simulink model "lagrange_model_v2"  (R2022a)
(part 3 of 3)

M32 = 1.3806*(0.19*cos(th4(t))*(cos(th3(t) - 1.5708)*(sin(th2(t) - 1.5708)*(1.0*cos(th1(t)) - 2.6536e-6*sin(th1(t))) - 1.3268e-6*cos(th2(t) - 1.5708)*sin(th1(t))) + sin(th3(t) - 1.5708)*(cos(th2(t) - 1.5708)*(1.0*cos(th1(t)) - 2.6536e-6*sin(th1(t))) + 1.3268e-6*sin(th2(t) - 1.5708)*sin(th1(t)))) + 0.38*cos(th3(t))*(sin(th2(t) - 1.5708)*(1.0*cos(th1(t)) - 2.6536e-6*sin(th1(t))) - 1.3268e-6*cos(th2(t) - 1.5708)*sin(th1(t))) + 0.38*sin(th3(t))*(cos(th2(t) - 1.5708)*(1.0*cos(th1(t)) - 2.6536e-6*sin(th1(t))) + 1.3268e-6*sin(th2(t) - 1.5708)*sin(th1(t))) + 0.19*sin(th4(t))*(cos(th3(t) - 1.5708)*(cos(th2(t) - 1.5708)*(1.0*cos(th1(t)) - 2.6536e-6*sin(th1(t))) + 1.3268e-6*sin(th2(t) - 1.5708)*sin(th1(t))) - 1.0*sin(th3(t) - 1.5708)*(sin(th2(t) - 1.5708)*(1.0*cos(th1(t)) - 2.6536e-6*sin(th1(t))) - 1.3268e-6*cos(th2(t) - 1.5708)*sin(th1(t)))))*(0.19*cos(th4(t))*(cos(th3(t) - 1.5708)*(sin(th2(t) - 1.5708)*(1.0*cos(th1(t)) - 2.6536e-6*sin(th1(t))) - 1.3268e-6*cos(th2(t) - 1.5708)*sin(th1(t))) + sin(th3(t) - 1.5708)*(cos(th2(t) - 1.5708)*(1.0*cos(th1(t)) - 2.6536e-6*sin(th1(t))) + 1.3268e-6*sin(th2(t) - 1.5708)*sin(th1(t)))) - 5.0418e-7*cos(th2(t))*sin(th1(t)) + 0.38*cos(th3(t))*(sin(th2(t) - 1.5708)*(1.0*cos(th1(t)) - 2.6536e-6*sin(th1(t))) - 1.3268e-6*cos(th2(t) - 1.5708)*sin(th1(t))) + 0.38*sin(th2(t))*(1.0*cos(th1(t)) - 2.6536e-6*sin(th1(t))) + 0.38*sin(th3(t))*(cos(th2(t) - 1.5708)*(1.0*cos(th1(t)) - 2.6536e-6*sin(th1(t))) + 1.3268e-6*sin(th2(t) - 1.5708)*sin(th1(t))) + 0.19*sin(th4(t))*(cos(th3(t) - 1.5708)*(cos(th2(t) - 1.5708)*(1.0*cos(th1(t)) - 2.6536e-6*sin(th1(t))) + 1.3268e-6*sin(th2(t) - 1.5708)*sin(th1(t))) - 1.0*sin(th3(t) - 1.5708)*(sin(th2(t) - 1.5708)*(1.0*cos(th1(t)) - 2.6536e-6*sin(th1(t))) - 1.3268e-6*cos(th2(t) - 1.5708)*sin(th1(t))))) - 1.3806*(0.38*sin(th3(t))*(3.5208e-12*cos(th2(t) - 1.5708) + 1.0*sin(th2(t) - 1.5708)) + 0.19*sin(th4(t))*(cos(th3(t) - 1.5708)*(3.5208e-12*cos(th2(t) - 1.5708) + 1.0*sin(th2(t) - 1.5708)) + sin(th3(t) - 1.5708)*(1.0*cos(th2(t) - 1.5708) - 3.5208e-12*sin(th2(t) - 1.5708))) - 0.19*cos(th4(t))*(cos(th3(t) - 1.5708)*(1.0*cos(th2(t) - 1.5708) - 3.5208e-12*sin(th2(t) - 1.5708)) - 1.0*sin(th3(t) - 1.5708)*(3.5208e-12*cos(th2(t) - 1.5708) + 1.0*sin(th2(t) - 1.5708))) - 0.38*cos(th3(t))*(1.0*cos(th2(t) - 1.5708) - 3.5208e-12*sin(th2(t) - 1.5708)))*(0.38*cos(th2(t)) - 1.3379e-12*sin(th2(t)) - 0.38*sin(th3(t))*(3.5208e-12*cos(th2(t) - 1.5708) + 1.0*sin(th2(t) - 1.5708)) - 0.19*sin(th4(t))*(cos(th3(t) - 1.5708)*(3.5208e-12*cos(th2(t) - 1.5708) + 1.0*sin(th2(t) - 1.5708)) + sin(th3(t) - 1.5708)*(1.0*cos(th2(t) - 1.5708) - 3.5208e-12*sin(th2(t) - 1.5708))) + 0.19*cos(th4(t))*(cos(th3(t) - 1.5708)*(1.0*cos(th2(t) - 1.5708) - 3.5208e-12*sin(th2(t) - 1.5708)) - 1.0*sin(th3(t) - 1.5708)*(3.5208e-12*cos(th2(t) - 1.5708) + 1.0*sin(th2(t) - 1.5708))) + 0.38*cos(th3(t))*(1.0*cos(th2(t) - 1.5708) - 3.5208e-12*sin(th2(t) - 1.5708))) + 0.13038*(0.38*cos(th3(t))*(sin(th2(t) - 1.5708)*(2.6536e-6*cos(th1(t)) + 1.0*sin(th1(t))) + 1.3268e-6*cos(th2(t) - 1.5708)*cos(th1(t))) - 0.38*sin(th4(t))*(sin(th3(t) - 1.5708)*(sin(th2(t) - 1.5708)*(2.6536e-6*cos(th1(t)) + 1.0*sin(th1(t))) + 1.3268e-6*cos(th2(t) - 1.5708)*cos(th1(t))) - cos(th3(t) - 1.5708)*(1.0*cos(th2(t) - 1.5708)*(2.6536e-6*cos(th1(t)) + 1.0*sin(th1(t))) - 1.3268e-6*sin(th2(t) - 1.5708)*cos(th1(t)))) + 0.38*sin(th3(t))*(1.0*cos(th2(t) - 1.5708)*(2.6536e-6*cos(th1(t)) + 1.0*sin(th1(t))) - 1.3268e-6*sin(th2(t) - 1.5708)*cos(th1(t))) - 0.02*cos(th5(t))*(sin(th4(t) - 3.1416)*(sin(th3(t) - 1.5708)*(sin(th2(t) - 1.5708)*(2.6536e-6*cos(th1(t)) + 1.0*sin(th1(t))) + 1.3268e-6*cos(th2(t) - 1.5708)*cos(th1(t))) - cos(th3(t) - 1.5708)*(1.0*cos(th2(t) - 1.5708)*(2.6536e-6*cos(th1(t)) + 1.0*sin(th1(t))) - 1.3268e-6*sin(th2(t) - 1.5708)*cos(th1(t)))) + cos(th4(t) - 3.1416)*(cos(th3(t) - 1.5708)*(sin(th2(t) - 1.5708)*(2.6536e-6*cos(th1(t)) + 1.0*sin(th1(t))) + 1.3268e-6*cos(th2(t) - 1.5708)*cos(th1(t))) + 1.0*sin(th3(t) - 1.5708)*(1.0*cos(th2(t) - 1.5708)*(2.6536e-6*cos(th1(t)) + 1.0*sin(th1(t))) - 1.3268e-6*sin(th2(t) - 1.5708)*cos(th1(t))))) + 0.38*cos(th4(t))*(cos(th3(t) - 1.5708)*(sin(th2(t) - 1.5708)*(2.6536e-6*cos(th1(t)) + 1.0*sin(th1(t))) + 1.3268e-6*cos(th2(t) - 1.5708)*cos(th1(t))) + 1.0*sin(th3(t) - 1.5708)*(1.0*cos(th2(t) - 1.5708)*(2.6536e-6*cos(th1(t)) + 1.0*sin(th1(t))) - 1.3268e-6*sin(th2(t) - 1.5708)*cos(th1(t)))) + 0.02*sin(th5(t))*(cos(th4(t) - 3.1416)*(sin(th3(t) - 1.5708)*(sin(th2(t) - 1.5708)*(2.6536e-6*cos(th1(t)) + 1.0*sin(th1(t))) + 1.3268e-6*cos(th2(t) - 1.5708)*cos(th1(t))) - cos(th3(t) - 1.5708)*(1.0*cos(th2(t) - 1.5708)*(2.6536e-6*cos(th1(t)) + 1.0*sin(th1(t))) - 1.3268e-6*sin(th2(t) - 1.5708)*cos(th1(t)))) - 1.0*sin(th4(t) - 3.1416)*(cos(th3(t) - 1.5708)*(sin(th2(t) - 1.5708)*(2.6536e-6*cos(th1(t)) + 1.0*sin(th1(t))) + 1.3268e-6*cos(th2(t) - 1.5708)*cos(th1(t))) + 1.0*sin(th3(t) - 1.5708)*(1.0*cos(th2(t) - 1.5708)*(2.6536e-6*cos(th1(t)) + 1.0*sin(th1(t))) - 1.3268e-6*sin(th2(t) - 1.5708)*cos(th1(t))))))*(0.38*cos(th3(t))*(sin(th2(t) - 1.5708)*(2.6536e-6*cos(th1(t)) + 1.0*sin(th1(t))) + 1.3268e-6*cos(th2(t) - 1.5708)*cos(th1(t))) + 0.38*sin(th2(t))*(2.6536e-6*cos(th1(t)) + 1.0*sin(th1(t))) - 0.38*sin(th4(t))*(sin(th3(t) - 1.5708)*(sin(th2(t) - 1.5708)*(2.6536e-6*cos(th1(t)) + 1.0*sin(th1(t))) + 1.3268e-6*cos(th2(t) - 1.5708)*cos(th1(t))) - cos(th3(t) - 1.5708)*(1.0*cos(th2(t) - 1.5708)*(2.6536e-6*cos(th1(t)) + 1.0*sin(th1(t))) - 1.3268e-6*sin(th2(t) - 1.5708)*cos(th1(t)))) + 0.38*sin(th3(t))*(1.0*cos(th2(t) - 1.5708)*(2.6536e-6*cos(th1(t)) + 1.0*sin(th1(t))) - 1.3268e-6*sin(th2(t) - 1.5708)*cos(th1(t))) - 0.02*cos(th5(t))*(sin(th4(t) - 3.1416)*(sin(th3(t) - 1.5708)*(sin(th2(t) - 1.5708)*(2.6536e-6*cos(th1(t)) + 1.0*sin(th1(t))) + 1.3268e-6*cos(th2(t) - 1.5708)*cos(th1(t))) - cos(th3(t) - 1.5708)*(1.0*cos(th2(t) - 1.5708)*(2.6536e-6*cos(th1(t)) + 1.0*sin(th1(t))) - 1.3268e-6*sin(th2(t) - 1.5708)*cos(th1(t)))) + cos(th4(t) - 3.1416)*(cos(th3(t) - 1.5708)*(sin(th2(t) - 1.5708)*(2.6536e-6*cos(th1(t)) + 1.0*sin(th1(t))) + 1.3268e-6*cos(th2(t) - 1.5708)*cos(th1(t))) + 1.0*sin(th3(t) - 1.5708)*(1.0*cos(th2(t) - 1.5708)*(2.6536e-6*cos(th1(t)) + 1.0*sin(th1(t))) - 1.3268e-6*sin(th2(t) - 1.5708)*cos(th1(t))))) + 0.38*cos(th4(t))*(cos(th3(t) - 1.5708)*(sin(th2(t) - 1.5708)*(2.6536e-6*cos(th1(t)) + 1.0*sin(th1(t))) + 1.3268e-6*cos(th2(t) - 1.5708)*cos(th1(t))) + 1.0*sin(th3(t) - 1.5708)*(1.0*cos(th2(t) - 1.5708)*(2.6536e-6*cos(th1(t)) + 1.0*sin(th1(t))) - 1.3268e-6*sin(th2(t) - 1.5708)*cos(th1(t)))) + 0.02*sin(th5(t))*(cos(th4(t) - 3.1416)*(sin(th3(t) - 1.5708)*(sin(th2(t) - 1.5708)*(2.6536e-6*cos(th1(t)) + 1.0*sin(th1(t))) + 1.3268e-6*cos(th2(t) - 1.5708)*cos(th1(t))) - cos(th3(t) - 1.5708)*(1.0*cos(th2(t) - 1.5708)*(2.6536e-6*cos(th1(t)) + 1.0*sin(th1(t))) - 1.3268e-6*sin(th2(t) - 1.5708)*cos(th1(t)))) - 1.0*sin(th4(t) - 3.1416)*(cos(th3(t) - 1.5708)*(sin(th2(t) - 1.5708)*(2.6536e-6*cos(th1(t)) + 1.0*sin(th1(t))) + 1.3268e-6*cos(th2(t) - 1.5708)*cos(th1(t))) + 1.0*sin(th3(t) - 1.5708)*(1.0*cos(th2(t) - 1.5708)*(2.6536e-6*cos(th1(t)) + 1.0*sin(th1(t))) - 1.3268e-6*sin(th2(t) - 1.5708)*cos(th1(t))))) + 5.0418e-7*cos(th1(t))*cos(th2(t))) + 0.49277*(0.19*cos(th3(t))*(sin(th2(t) - 1.5708)*(2.6536e-6*cos(th1(t)) + 1.0*sin(th1(t))) + 1.3268e-6*cos(th2(t) - 1.5708)*cos(th1(t))) + 0.19*sin(th3(t))*(1.0*cos(th2(t) - 1.5708)*(2.6536e-6*cos(th1(t)) + 1.0*sin(th1(t))) - 1.3268e-6*sin(th2(t) - 1.5708)*cos(th1(t))))*(0.19*cos(th3(t))*(sin(th2(t) - 1.5708)*(2.6536e-6*cos(th1(t)) + 1.0*sin(th1(t))) + 1.3268e-6*cos(th2(t) - 1.5708)*cos(th1(t))) + 0.38*sin(th2(t))*(2.6536e-6*cos(th1(t)) + 1.0*sin(th1(t))) + 0.19*sin(th3(t))*(1.0*cos(th2(t) - 1.5708)*(2.6536e-6*cos(th1(t)) + 1.0*sin(th1(t))) - 1.3268e-6*sin(th2(t) - 1.5708)*cos(th1(t))) + 5.0418e-7*cos(th1(t))*cos(th2(t))) + 0.13038*(0.38*cos(th4(t))*(cos(th3(t) - 1.5708)*(sin(th2(t) - 1.5708)*(1.0*cos(th1(t)) - 2.6536e-6*sin(th1(t))) - 1.3268e-6*cos(th2(t) - 1.5708)*sin(th1(t))) + sin(th3(t) - 1.5708)*(cos(th2(t) - 1.5708)*(1.0*cos(th1(t)) - 2.6536e-6*sin(th1(t))) + 1.3268e-6*sin(th2(t) - 1.5708)*sin(th1(t)))) + 0.38*cos(th3(t))*(sin(th2(t) - 1.5708)*(1.0*cos(th1(t)) - 2.6536e-6*sin(th1(t))) - 1.3268e-6*cos(th2(t) - 1.5708)*sin(th1(t))) + 0.38*sin(th3(t))*(cos(th2(t) - 1.5708)*(1.0*cos(th1(t)) - 2.6536e-6*sin(th1(t))) + 1.3268e-6*sin(th2(t) - 1.5708)*sin(th1(t))) - 0.02*sin(th5(t))*(sin(th4(t) - 3.1416)*(cos(th3(t) - 1.5708)*(sin(th2(t) - 1.5708)*(1.0*cos(th1(t)) - 2.6536e-6*sin(th1(t))) - 1.3268e-6*cos(th2(t) - 1.5708)*sin(th1(t))) + sin(th3(t) - 1.5708)*(cos(th2(t) - 1.5708)*(1.0*cos(th1(t)) - 2.6536e-6*sin(th1(t))) + 1.3268e-6*sin(th2(t) - 1.5708)*sin(th1(t)))) + cos(th4(t) - 3.1416)*(cos(th3(t) - 1.5708)*(cos(th2(t) - 1.5708)*(1.0*cos(th1(t)) - 2.6536e-6*sin(th1(t))) + 1.3268e-6*sin(th2(t) - 1.5708)*sin(th1(t))) - 1.0*sin(th3(t) - 1.5708)*(sin(th2(t) - 1.5708)*(1.0*cos(th1(t)) - 2.6536e-6*sin(th1(t))) - 1.3268e-6*cos(th2(t) - 1.5708)*sin(th1(t))))) + 0.38*sin(th4(t))*(cos(th3(t) - 1.5708)*(cos(th2(t) - 1.5708)*(1.0*cos(th1(t)) - 2.6536e-6*sin(th1(t))) + 1.3268e-6*sin(th2(t) - 1.5708)*sin(th1(t))) - 1.0*sin(th3(t) - 1.5708)*(sin(th2(t) - 1.5708)*(1.0*cos(th1(t)) - 2.6536e-6*sin(th1(t))) - 1.3268e-6*cos(th2(t) - 1.5708)*sin(th1(t)))) - 0.02*cos(th5(t))*(cos(th4(t) - 3.1416)*(cos(th3(t) - 1.5708)*(sin(th2(t) - 1.5708)*(1.0*cos(th1(t)) - 2.6536e-6*sin(th1(t))) - 1.3268e-6*cos(th2(t) - 1.5708)*sin(th1(t))) + sin(th3(t) - 1.5708)*(cos(th2(t) - 1.5708)*(1.0*cos(th1(t)) - 2.6536e-6*sin(th1(t))) + 1.3268e-6*sin(th2(t) - 1.5708)*sin(th1(t)))) - 1.0*sin(th4(t) - 3.1416)*(cos(th3(t) - 1.5708)*(cos(th2(t) - 1.5708)*(1.0*cos(th1(t)) - 2.6536e-6*sin(th1(t))) + 1.3268e-6*sin(th2(t) - 1.5708)*sin(th1(t))) - 1.0*sin(th3(t) - 1.5708)*(sin(th2(t) - 1.5708)*(1.0*cos(th1(t)) - 2.6536e-6*sin(th1(t))) - 1.3268e-6*cos(th2(t) - 1.5708)*sin(th1(t))))))*(0.38*cos(th4(t))*(cos(th3(t) - 1.5708)*(sin(th2(t) - 1.5708)*(1.0*cos(th1(t)) - 2.6536e-6*sin(th1(t))) - 1.3268e-6*cos(th2(t) - 1.5708)*sin(th1(t))) + sin(th3(t) - 1.5708)*(cos(th2(t) - 1.5708)*(1.0*cos(th1(t)) - 2.6536e-6*sin(th1(t))) + 1.3268e-6*sin(th2(t) - 1.5708)*sin(th1(t)))) - 5.0418e-7*cos(th2(t))*sin(th1(t)) + 0.38*cos(th3(t))*(sin(th2(t) - 1.5708)*(1.0*cos(th1(t)) - 2.6536e-6*sin(th1(t))) - 1.3268e-6*cos(th2(t) - 1.5708)*sin(th1(t))) + 0.38*sin(th2(t))*(1.0*cos(th1(t)) - 2.6536e-6*sin(th1(t))) + 0.38*sin(th3(t))*(cos(th2(t) - 1.5708)*(1.0*cos(th1(t)) - 2.6536e-6*sin(th1(t))) + 1.3268e-6*sin(th2(t) - 1.5708)*sin(th1(t))) - 0.02*sin(th5(t))*(sin(th4(t) - 3.1416)*(cos(th3(t) - 1.5708)*(sin(th2(t) - 1.5708)*(1.0*cos(th1(t)) - 2.6536e-6*sin(th1(t))) - 1.3268e-6*cos(th2(t) - 1.5708)*sin(th1(t))) + sin(th3(t) - 1.5708)*(cos(th2(t) - 1.5708)*(1.0*cos(th1(t)) - 2.6536e-6*sin(th1(t))) + 1.3268e-6*sin(th2(t) - 1.5708)*sin(th1(t)))) + cos(th4(t) - 3.1416)*(cos(th3(t) - 1.5708)*(cos(th2(t) - 1.5708)*(1.0*cos(th1(t)) - 2.6536e-6*sin(th1(t))) + 1.3268e-6*sin(th2(t) - 1.5708)*sin(th1(t))) - 1.0*sin(th3(t) - 1.5708)*(sin(th2(t) - 1.5708)*(1.0*cos(th1(t)) - 2.6536e-6*sin(th1(t))) - 1.3268e-6*cos(th2(t) - 1.5708)*sin(th1(t))))) + 0.38*sin(th4(t))*(cos(th3(t) - 1.5708)*(cos(th2(t) - 1.5708)*(1.0*cos(th1(t)) - 2.6536e-6*sin(th1(t))) + 1.3268e-6*sin(th2(t) - 1.5708)*sin(th1(t))) - 1.0*sin(th3(t) - 1.5708)*(sin(th2(t) - 1.5708)*(1.0*cos(th1(t)) - 2.6536e-6*sin(th1(t))) - 1.3268e-6*cos(th2(t) - 1.5708)*sin(th1(t)))) - 0.02*cos(th5(t))*(cos(th4(t) - 3.1416)*(cos(th3(t) - 1.5708)*(sin(th2(t) - 1.5708)*(1.0*cos(th1(t)) - 2.6536e-6*sin(th1(t))) - 1.3268e-6*cos(th2(t) - 1.5708)*sin(th1(t))) + sin(th3(t) - 1.5708)*(cos(th2(t) - 1.5708)*(1.0*cos(th1(t)) - 2.6536e-6*sin(th1(t))) + 1.3268e-6*sin(th2(t) - 1.5708)*sin(th1(t)))) - 1.0*sin(th4(t) - 3.1416)*(cos(th3(t) - 1.5708)*(cos(th2(t) - 1.5708)*(1.0*cos(th1(t)) - 2.6536e-6*sin(th1(t))) + 1.3268e-6*sin(th2(t) - 1.5708)*sin(th1(t))) - 1.0*sin(th3(t) - 1.5708)*(sin(th2(t) - 1.5708)*(1.0*cos(th1(t)) - 2.6536e-6*sin(th1(t))) - 1.3268e-6*cos(th2(t) - 1.5708)*sin(th1(t)))))) - 0.49277*(0.19*sin(th3(t))*(3.5208e-12*cos(th2(t) - 1.5708) + 1.0*sin(th2(t) - 1.5708)) - 0.19*cos(th3(t))*(1.0*cos(th2(t) - 1.5708) - 3.5208e-12*sin(th2(t) - 1.5708)))*(0.38*cos(th2(t)) - 1.3379e-12*sin(th2(t)) - 0.19*sin(th3(t))*(3.5208e-12*cos(th2(t) - 1.5708) + 1.0*sin(th2(t) - 1.5708)) + 0.19*cos(th3(t))*(1.0*cos(th2(t) - 1.5708) - 3.5208e-12*sin(th2(t) - 1.5708))) + 1.3806*(0.38*cos(th3(t))*(sin(th2(t) - 1.5708)*(2.6536e-6*cos(th1(t)) + 1.0*sin(th1(t))) + 1.3268e-6*cos(th2(t) - 1.5708)*cos(th1(t))) - 0.19*sin(th4(t))*(sin(th3(t) - 1.5708)*(sin(th2(t) - 1.5708)*(2.6536e-6*cos(th1(t)) + 1.0*sin(th1(t))) + 1.3268e-6*cos(th2(t) - 1.5708)*cos(th1(t))) - cos(th3(t) - 1.5708)*(1.0*cos(th2(t) - 1.5708)*(2.6536e-6*cos(th1(t)) + 1.0*sin(th1(t))) - 1.3268e-6*sin(th2(t) - 1.5708)*cos(th1(t)))) + 0.38*sin(th3(t))*(1.0*cos(th2(t) - 1.5708)*(2.6536e-6*cos(th1(t)) + 1.0*sin(th1(t))) - 1.3268e-6*sin(th2(t) - 1.5708)*cos(th1(t))) + 0.19*cos(th4(t))*(cos(th3(t) - 1.5708)*(sin(th2(t) - 1.5708)*(2.6536e-6*cos(th1(t)) + 1.0*sin(th1(t))) + 1.3268e-6*cos(th2(t) - 1.5708)*cos(th1(t))) + 1.0*sin(th3(t) - 1.5708)*(1.0*cos(th2(t) - 1.5708)*(2.6536e-6*cos(th1(t)) + 1.0*sin(th1(t))) - 1.3268e-6*sin(th2(t) - 1.5708)*cos(th1(t)))))*(0.38*cos(th3(t))*(sin(th2(t) - 1.5708)*(2.6536e-6*cos(th1(t)) + 1.0*sin(th1(t))) + 1.3268e-6*cos(th2(t) - 1.5708)*cos(th1(t))) + 0.38*sin(th2(t))*(2.6536e-6*cos(th1(t)) + 1.0*sin(th1(t))) - 0.19*sin(th4(t))*(sin(th3(t) - 1.5708)*(sin(th2(t) - 1.5708)*(2.6536e-6*cos(th1(t)) + 1.0*sin(th1(t))) + 1.3268e-6*cos(th2(t) - 1.5708)*cos(th1(t))) - cos(th3(t) - 1.5708)*(1.0*cos(th2(t) - 1.5708)*(2.6536e-6*cos(th1(t)) + 1.0*sin(th1(t))) - 1.3268e-6*sin(th2(t) - 1.5708)*cos(th1(t)))) + 0.38*sin(th3(t))*(1.0*cos(th2(t) - 1.5708)*(2.6536e-6*cos(th1(t)) + 1.0*sin(th1(t))) - 1.3268e-6*sin(th2(t) - 1.5708)*cos(th1(t))) + 0.19*cos(th4(t))*(cos(th3(t) - 1.5708)*(sin(th2(t) - 1.5708)*(2.6536e-6*cos(th1(t)) + 1.0*sin(th1(t))) + 1.3268e-6*cos(th2(t) - 1.5708)*cos(th1(t))) + 1.0*sin(th3(t) - 1.5708)*(1.0*cos(th2(t) - 1.5708)*(2.6536e-6*cos(th1(t)) + 1.0*sin(th1(t))) - 1.3268e-6*sin(th2(t) - 1.5708)*cos(th1(t)))) + 5.0418e-7*cos(th1(t))*cos(th2(t))) - 0.13038*(0.38*sin(th3(t))*(3.5208e-12*cos(th2(t) - 1.5708) + 1.0*sin(th2(t) - 1.5708)) - 0.02*sin(th5(t))*(cos(th4(t) - 3.1416)*(cos(th3(t) - 1.5708)*(3.5208e-12*cos(th2(t) - 1.5708) + 1.0*sin(th2(t) - 1.5708)) + sin(th3(t) - 1.5708)*(1.0*cos(th2(t) - 1.5708) - 3.5208e-12*sin(th2(t) - 1.5708))) - 1.0*sin(th4(t) - 3.1416)*(cos(th3(t) - 1.5708)*(1.0*cos(th2(t) - 1.5708) - 3.5208e-12*sin(th2(t) - 1.5708)) - 1.0*sin(th3(t) - 1.5708)*(3.5208e-12*cos(th2(t) - 1.5708) + 1.0*sin(th2(t) - 1.5708)))) + 0.38*sin(th4(t))*(cos(th3(t) - 1.5708)*(3.5208e-12*cos(th2(t) - 1.5708) + 1.0*sin(th2(t) - 1.5708)) + sin(th3(t) - 1.5708)*(1.0*cos(th2(t) - 1.5708) - 3.5208e-12*sin(th2(t) - 1.5708))) - 0.38*cos(th4(t))*(cos(th3(t) - 1.5708)*(1.0*cos(th2(t) - 1.5708) - 3.5208e-12*sin(th2(t) - 1.5708)) - 1.0*sin(th3(t) - 1.5708)*(3.5208e-12*cos(th2(t) - 1.5708) + 1.0*sin(th2(t) - 1.5708))) - 0.38*cos(th3(t))*(1.0*cos(th2(t) - 1.5708) - 3.5208e-12*sin(th2(t) - 1.5708)) + 0.02*cos(th5(t))*(sin(th4(t) - 3.1416)*(cos(th3(t) - 1.5708)*(3.5208e-12*cos(th2(t) - 1.5708) + 1.0*sin(th2(t) - 1.5708)) + sin(th3(t) - 1.5708)*(1.0*cos(th2(t) - 1.5708) - 3.5208e-12*sin(th2(t) - 1.5708))) + cos(th4(t) - 3.1416)*(cos(th3(t) - 1.5708)*(1.0*cos(th2(t) - 1.5708) - 3.5208e-12*sin(th2(t) - 1.5708)) - 1.0*sin(th3(t) - 1.5708)*(3.5208e-12*cos(th2(t) - 1.5708) + 1.0*sin(th2(t) - 1.5708)))))*(0.38*cos(th2(t)) - 1.3379e-12*sin(th2(t)) - 0.38*sin(th3(t))*(3.5208e-12*cos(th2(t) - 1.5708) + 1.0*sin(th2(t) - 1.5708)) + 0.02*sin(th5(t))*(cos(th4(t) - 3.1416)*(cos(th3(t) - 1.5708)*(3.5208e-12*cos(th2(t) - 1.5708) + 1.0*sin(th2(t) - 1.5708)) + sin(th3(t) - 1.5708)*(1.0*cos(th2(t) - 1.5708) - 3.5208e-12*sin(th2(t) - 1.5708))) - 1.0*sin(th4(t) - 3.1416)*(cos(th3(t) - 1.5708)*(1.0*cos(th2(t) - 1.5708) - 3.5208e-12*sin(th2(t) - 1.5708)) - 1.0*sin(th3(t) - 1.5708)*(3.5208e-12*cos(th2(t) - 1.5708) + 1.0*sin(th2(t) - 1.5708)))) - 0.38*sin(th4(t))*(cos(th3(t) - 1.5708)*(3.5208e-12*cos(th2(t) - 1.5708) + 1.0*sin(th2(t) - 1.5708)) + sin(th3(t) - 1.5708)*(1.0*cos(th2(t) - 1.5708) - 3.5208e-12*sin(th2(t) - 1.5708))) + 0.38*cos(th4(t))*(cos(th3(t) - 1.5708)*(1.0*cos(th2(t) - 1.5708) - 3.5208e-12*sin(th2(t) - 1.5708)) - 1.0*sin(th3(t) - 1.5708)*(3.5208e-12*cos(th2(t) - 1.5708) + 1.0*sin(th2(t) - 1.5708))) + 0.38*cos(th3(t))*(1.0*cos(th2(t) - 1.5708) - 3.5208e-12*sin(th2(t) - 1.5708)) - 0.02*cos(th5(t))*(sin(th4(t) - 3.1416)*(cos(th3(t) - 1.5708)*(3.5208e-12*cos(th2(t) - 1.5708) + 1.0*sin(th2(t) - 1.5708)) + sin(th3(t) - 1.5708)*(1.0*cos(th2(t) - 1.5708) - 3.5208e-12*sin(th2(t) - 1.5708))) + cos(th4(t) - 3.1416)*(cos(th3(t) - 1.5708)*(1.0*cos(th2(t) - 1.5708) - 3.5208e-12*sin(th2(t) - 1.5708)) - 1.0*sin(th3(t) - 1.5708)*(3.5208e-12*cos(th2(t) - 1.5708) + 1.0*sin(th2(t) - 1.5708))))) + 0.49277*(0.19*cos(th3(t))*(sin(th2(t) - 1.5708)*(1.0*cos(th1(t)) - 2.6536e-6*sin(th1(t))) - 1.3268e-6*cos(th2(t) - 1.5708)*sin(th1(t))) + 0.19*sin(th3(t))*(cos(th2(t) - 1.5708)*(1.0*cos(th1(t)) - 2.6536e-6*sin(th1(t))) + 1.3268e-6*sin(th2(t) - 1.5708)*sin(th1(t))))*(0.19*cos(th3(t))*(sin(th2(t) - 1.5708)*(1.0*cos(th1(t)) - 2.6536e-6*sin(th1(t))) - 1.3268e-6*cos(th2(t) - 1.5708)*sin(th1(t))) - 5.0418e-7*cos(th2(t))*sin(th1(t)) + 0.38*sin(th2(t))*(1.0*cos(th1(t)) - 2.6536e-6*sin(th1(t))) + 0.19*sin(th3(t))*(cos(th2(t) - 1.5708)*(1.0*cos(th1(t)) - 2.6536e-6*sin(th1(t))) + 1.3268e-6*sin(th2(t) - 1.5708)*sin(th1(t)))) + 0.051004;
M33 = 1.3806*(0.38*cos(th3(t))*(sin(th2(t) - 1.5708)*(2.6536e-6*cos(th1(t)) + 1.0*sin(th1(t))) + 1.3268e-6*cos(th2(t) - 1.5708)*cos(th1(t))) - 0.19*sin(th4(t))*(sin(th3(t) - 1.5708)*(sin(th2(t) - 1.5708)*(2.6536e-6*cos(th1(t)) + 1.0*sin(th1(t))) + 1.3268e-6*cos(th2(t) - 1.5708)*cos(th1(t))) - cos(th3(t) - 1.5708)*(1.0*cos(th2(t) - 1.5708)*(2.6536e-6*cos(th1(t)) + 1.0*sin(th1(t))) - 1.3268e-6*sin(th2(t) - 1.5708)*cos(th1(t)))) + 0.38*sin(th3(t))*(1.0*cos(th2(t) - 1.5708)*(2.6536e-6*cos(th1(t)) + 1.0*sin(th1(t))) - 1.3268e-6*sin(th2(t) - 1.5708)*cos(th1(t))) + 0.19*cos(th4(t))*(cos(th3(t) - 1.5708)*(sin(th2(t) - 1.5708)*(2.6536e-6*cos(th1(t)) + 1.0*sin(th1(t))) + 1.3268e-6*cos(th2(t) - 1.5708)*cos(th1(t))) + 1.0*sin(th3(t) - 1.5708)*(1.0*cos(th2(t) - 1.5708)*(2.6536e-6*cos(th1(t)) + 1.0*sin(th1(t))) - 1.3268e-6*sin(th2(t) - 1.5708)*cos(th1(t)))))^2 + 0.49277*(0.19*cos(th3(t))*(sin(th2(t) - 1.5708)*(1.0*cos(th1(t)) - 2.6536e-6*sin(th1(t))) - 1.3268e-6*cos(th2(t) - 1.5708)*sin(th1(t))) + 0.19*sin(th3(t))*(cos(th2(t) - 1.5708)*(1.0*cos(th1(t)) - 2.6536e-6*sin(th1(t))) + 1.3268e-6*sin(th2(t) - 1.5708)*sin(th1(t))))^2 + 0.13038*(0.38*cos(th3(t))*(sin(th2(t) - 1.5708)*(2.6536e-6*cos(th1(t)) + 1.0*sin(th1(t))) + 1.3268e-6*cos(th2(t) - 1.5708)*cos(th1(t))) - 0.38*sin(th4(t))*(sin(th3(t) - 1.5708)*(sin(th2(t) - 1.5708)*(2.6536e-6*cos(th1(t)) + 1.0*sin(th1(t))) + 1.3268e-6*cos(th2(t) - 1.5708)*cos(th1(t))) - cos(th3(t) - 1.5708)*(1.0*cos(th2(t) - 1.5708)*(2.6536e-6*cos(th1(t)) + 1.0*sin(th1(t))) - 1.3268e-6*sin(th2(t) - 1.5708)*cos(th1(t)))) + 0.38*sin(th3(t))*(1.0*cos(th2(t) - 1.5708)*(2.6536e-6*cos(th1(t)) + 1.0*sin(th1(t))) - 1.3268e-6*sin(th2(t) - 1.5708)*cos(th1(t))) - 0.02*cos(th5(t))*(sin(th4(t) - 3.1416)*(sin(th3(t) - 1.5708)*(sin(th2(t) - 1.5708)*(2.6536e-6*cos(th1(t)) + 1.0*sin(th1(t))) + 1.3268e-6*cos(th2(t) - 1.5708)*cos(th1(t))) - cos(th3(t) - 1.5708)*(1.0*cos(th2(t) - 1.5708)*(2.6536e-6*cos(th1(t)) + 1.0*sin(th1(t))) - 1.3268e-6*sin(th2(t) - 1.5708)*cos(th1(t)))) + cos(th4(t) - 3.1416)*(cos(th3(t) - 1.5708)*(sin(th2(t) - 1.5708)*(2.6536e-6*cos(th1(t)) + 1.0*sin(th1(t))) + 1.3268e-6*cos(th2(t) - 1.5708)*cos(th1(t))) + 1.0*sin(th3(t) - 1.5708)*(1.0*cos(th2(t) - 1.5708)*(2.6536e-6*cos(th1(t)) + 1.0*sin(th1(t))) - 1.3268e-6*sin(th2(t) - 1.5708)*cos(th1(t))))) + 0.38*cos(th4(t))*(cos(th3(t) - 1.5708)*(sin(th2(t) - 1.5708)*(2.6536e-6*cos(th1(t)) + 1.0*sin(th1(t))) + 1.3268e-6*cos(th2(t) - 1.5708)*cos(th1(t))) + 1.0*sin(th3(t) - 1.5708)*(1.0*cos(th2(t) - 1.5708)*(2.6536e-6*cos(th1(t)) + 1.0*sin(th1(t))) - 1.3268e-6*sin(th2(t) - 1.5708)*cos(th1(t)))) + 0.02*sin(th5(t))*(cos(th4(t) - 3.1416)*(sin(th3(t) - 1.5708)*(sin(th2(t) - 1.5708)*(2.6536e-6*cos(th1(t)) + 1.0*sin(th1(t))) + 1.3268e-6*cos(th2(t) - 1.5708)*cos(th1(t))) - cos(th3(t) - 1.5708)*(1.0*cos(th2(t) - 1.5708)*(2.6536e-6*cos(th1(t)) + 1.0*sin(th1(t))) - 1.3268e-6*sin(th2(t) - 1.5708)*cos(th1(t)))) - 1.0*sin(th4(t) - 3.1416)*(cos(th3(t) - 1.5708)*(sin(th2(t) - 1.5708)*(2.6536e-6*cos(th1(t)) + 1.0*sin(th1(t))) + 1.3268e-6*cos(th2(t) - 1.5708)*cos(th1(t))) + 1.0*sin(th3(t) - 1.5708)*(1.0*cos(th2(t) - 1.5708)*(2.6536e-6*cos(th1(t)) + 1.0*sin(th1(t))) - 1.3268e-6*sin(th2(t) - 1.5708)*cos(th1(t))))))^2 + 0.49277*(0.19*cos(th3(t))*(sin(th2(t) - 1.5708)*(2.6536e-6*cos(th1(t)) + 1.0*sin(th1(t))) + 1.3268e-6*cos(th2(t) - 1.5708)*cos(th1(t))) + 0.19*sin(th3(t))*(1.0*cos(th2(t) - 1.5708)*(2.6536e-6*cos(th1(t)) + 1.0*sin(th1(t))) - 1.3268e-6*sin(th2(t) - 1.5708)*cos(th1(t))))^2 + 0.13038*(0.38*cos(th4(t))*(cos(th3(t) - 1.5708)*(sin(th2(t) - 1.5708)*(1.0*cos(th1(t)) - 2.6536e-6*sin(th1(t))) - 1.3268e-6*cos(th2(t) - 1.5708)*sin(th1(t))) + sin(th3(t) - 1.5708)*(cos(th2(t) - 1.5708)*(1.0*cos(th1(t)) - 2.6536e-6*sin(th1(t))) + 1.3268e-6*sin(th2(t) - 1.5708)*sin(th1(t)))) + 0.38*cos(th3(t))*(sin(th2(t) - 1.5708)*(1.0*cos(th1(t)) - 2.6536e-6*sin(th1(t))) - 1.3268e-6*cos(th2(t) - 1.5708)*sin(th1(t))) + 0.38*sin(th3(t))*(cos(th2(t) - 1.5708)*(1.0*cos(th1(t)) - 2.6536e-6*sin(th1(t))) + 1.3268e-6*sin(th2(t) - 1.5708)*sin(th1(t))) - 0.02*sin(th5(t))*(sin(th4(t) - 3.1416)*(cos(th3(t) - 1.5708)*(sin(th2(t) - 1.5708)*(1.0*cos(th1(t)) - 2.6536e-6*sin(th1(t))) - 1.3268e-6*cos(th2(t) - 1.5708)*sin(th1(t))) + sin(th3(t) - 1.5708)*(cos(th2(t) - 1.5708)*(1.0*cos(th1(t)) - 2.6536e-6*sin(th1(t))) + 1.3268e-6*sin(th2(t) - 1.5708)*sin(th1(t)))) + cos(th4(t) - 3.1416)*(cos(th3(t) - 1.5708)*(cos(th2(t) - 1.5708)*(1.0*cos(th1(t)) - 2.6536e-6*sin(th1(t))) + 1.3268e-6*sin(th2(t) - 1.5708)*sin(th1(t))) - 1.0*sin(th3(t) - 1.5708)*(sin(th2(t) - 1.5708)*(1.0*cos(th1(t)) - 2.6536e-6*sin(th1(t))) - 1.3268e-6*cos(th2(t) - 1.5708)*sin(th1(t))))) + 0.38*sin(th4(t))*(cos(th3(t) - 1.5708)*(cos(th2(t) - 1.5708)*(1.0*cos(th1(t)) - 2.6536e-6*sin(th1(t))) + 1.3268e-6*sin(th2(t) - 1.5708)*sin(th1(t))) - 1.0*sin(th3(t) - 1.5708)*(sin(th2(t) - 1.5708)*(1.0*cos(th1(t)) - 2.6536e-6*sin(th1(t))) - 1.3268e-6*cos(th2(t) - 1.5708)*sin(th1(t)))) - 0.02*cos(th5(t))*(cos(th4(t) - 3.1416)*(cos(th3(t) - 1.5708)*(sin(th2(t) - 1.5708)*(1.0*cos(th1(t)) - 2.6536e-6*sin(th1(t))) - 1.3268e-6*cos(th2(t) - 1.5708)*sin(th1(t))) + sin(th3(t) - 1.5708)*(cos(th2(t) - 1.5708)*(1.0*cos(th1(t)) - 2.6536e-6*sin(th1(t))) + 1.3268e-6*sin(th2(t) - 1.5708)*sin(th1(t)))) - 1.0*sin(th4(t) - 3.1416)*(cos(th3(t) - 1.5708)*(cos(th2(t) - 1.5708)*(1.0*cos(th1(t)) - 2.6536e-6*sin(th1(t))) + 1.3268e-6*sin(th2(t) - 1.5708)*sin(th1(t))) - 1.0*sin(th3(t) - 1.5708)*(sin(th2(t) - 1.5708)*(1.0*cos(th1(t)) - 2.6536e-6*sin(th1(t))) - 1.3268e-6*cos(th2(t) - 1.5708)*sin(th1(t))))))^2 + 0.49277*(0.19*sin(th3(t))*(3.5208e-12*cos(th2(t) - 1.5708) + 1.0*sin(th2(t) - 1.5708)) - 0.19*cos(th3(t))*(1.0*cos(th2(t) - 1.5708) - 3.5208e-12*sin(th2(t) - 1.5708)))^2 + 0.13038*(0.38*sin(th3(t))*(3.5208e-12*cos(th2(t) - 1.5708) + 1.0*sin(th2(t) - 1.5708)) - 0.02*sin(th5(t))*(cos(th4(t) - 3.1416)*(cos(th3(t) - 1.5708)*(3.5208e-12*cos(th2(t) - 1.5708) + 1.0*sin(th2(t) - 1.5708)) + sin(th3(t) - 1.5708)*(1.0*cos(th2(t) - 1.5708) - 3.5208e-12*sin(th2(t) - 1.5708))) - 1.0*sin(th4(t) - 3.1416)*(cos(th3(t) - 1.5708)*(1.0*cos(th2(t) - 1.5708) - 3.5208e-12*sin(th2(t) - 1.5708)) - 1.0*sin(th3(t) - 1.5708)*(3.5208e-12*cos(th2(t) - 1.5708) + 1.0*sin(th2(t) - 1.5708)))) + 0.38*sin(th4(t))*(cos(th3(t) - 1.5708)*(3.5208e-12*cos(th2(t) - 1.5708) + 1.0*sin(th2(t) - 1.5708)) + sin(th3(t) - 1.5708)*(1.0*cos(th2(t) - 1.5708) - 3.5208e-12*sin(th2(t) - 1.5708))) - 0.38*cos(th4(t))*(cos(th3(t) - 1.5708)*(1.0*cos(th2(t) - 1.5708) - 3.5208e-12*sin(th2(t) - 1.5708)) - 1.0*sin(th3(t) - 1.5708)*(3.5208e-12*cos(th2(t) - 1.5708) + 1.0*sin(th2(t) - 1.5708))) - 0.38*cos(th3(t))*(1.0*cos(th2(t) - 1.5708) - 3.5208e-12*sin(th2(t) - 1.5708)) + 0.02*cos(th5(t))*(sin(th4(t) - 3.1416)*(cos(th3(t) - 1.5708)*(3.5208e-12*cos(th2(t) - 1.5708) + 1.0*sin(th2(t) - 1.5708)) + sin(th3(t) - 1.5708)*(1.0*cos(th2(t) - 1.5708) - 3.5208e-12*sin(th2(t) - 1.5708))) + cos(th4(t) - 3.1416)*(cos(th3(t) - 1.5708)*(1.0*cos(th2(t) - 1.5708) - 3.5208e-12*sin(th2(t) - 1.5708)) - 1.0*sin(th3(t) - 1.5708)*(3.5208e-12*cos(th2(t) - 1.5708) + 1.0*sin(th2(t) - 1.5708)))))^2 + 1.3806*(0.38*sin(th3(t))*(3.5208e-12*cos(th2(t) - 1.5708) + 1.0*sin(th2(t) - 1.5708)) + 0.19*sin(th4(t))*(cos(th3(t) - 1.5708)*(3.5208e-12*cos(th2(t) - 1.5708) + 1.0*sin(th2(t) - 1.5708)) + sin(th3(t) - 1.5708)*(1.0*cos(th2(t) - 1.5708) - 3.5208e-12*sin(th2(t) - 1.5708))) - 0.19*cos(th4(t))*(cos(th3(t) - 1.5708)*(1.0*cos(th2(t) - 1.5708) - 3.5208e-12*sin(th2(t) - 1.5708)) - 1.0*sin(th3(t) - 1.5708)*(3.5208e-12*cos(th2(t) - 1.5708) + 1.0*sin(th2(t) - 1.5708))) - 0.38*cos(th3(t))*(1.0*cos(th2(t) - 1.5708) - 3.5208e-12*sin(th2(t) - 1.5708)))^2 + 1.3806*(0.19*cos(th4(t))*(cos(th3(t) - 1.5708)*(sin(th2(t) - 1.5708)*(1.0*cos(th1(t)) - 2.6536e-6*sin(th1(t))) - 1.3268e-6*cos(th2(t) - 1.5708)*sin(th1(t))) + sin(th3(t) - 1.5708)*(cos(th2(t) - 1.5708)*(1.0*cos(th1(t)) - 2.6536e-6*sin(th1(t))) + 1.3268e-6*sin(th2(t) - 1.5708)*sin(th1(t)))) + 0.38*cos(th3(t))*(sin(th2(t) - 1.5708)*(1.0*cos(th1(t)) - 2.6536e-6*sin(th1(t))) - 1.3268e-6*cos(th2(t) - 1.5708)*sin(th1(t))) + 0.38*sin(th3(t))*(cos(th2(t) - 1.5708)*(1.0*cos(th1(t)) - 2.6536e-6*sin(th1(t))) + 1.3268e-6*sin(th2(t) - 1.5708)*sin(th1(t))) + 0.19*sin(th4(t))*(cos(th3(t) - 1.5708)*(cos(th2(t) - 1.5708)*(1.0*cos(th1(t)) - 2.6536e-6*sin(th1(t))) + 1.3268e-6*sin(th2(t) - 1.5708)*sin(th1(t))) - 1.0*sin(th3(t) - 1.5708)*(sin(th2(t) - 1.5708)*(1.0*cos(th1(t)) - 2.6536e-6*sin(th1(t))) - 1.3268e-6*cos(th2(t) - 1.5708)*sin(th1(t)))))^2 + 0.051004;
M34 = 0.13038*(0.02*sin(th5(t))*(cos(th4(t) - 3.1416)*(cos(th3(t) - 1.5708)*(3.5208e-12*cos(th2(t) - 1.5708) + 1.0*sin(th2(t) - 1.5708)) + sin(th3(t) - 1.5708)*(1.0*cos(th2(t) - 1.5708) - 3.5208e-12*sin(th2(t) - 1.5708))) - 1.0*sin(th4(t) - 3.1416)*(cos(th3(t) - 1.5708)*(1.0*cos(th2(t) - 1.5708) - 3.5208e-12*sin(th2(t) - 1.5708)) - 1.0*sin(th3(t) - 1.5708)*(3.5208e-12*cos(th2(t) - 1.5708) + 1.0*sin(th2(t) - 1.5708)))) + 0.38*sin(th4(t))*(cos(th3(t) - 1.5708)*(3.5208e-12*cos(th2(t) - 1.5708) + 1.0*sin(th2(t) - 1.5708)) + sin(th3(t) - 1.5708)*(1.0*cos(th2(t) - 1.5708) - 3.5208e-12*sin(th2(t) - 1.5708))) - 0.38*cos(th4(t))*(cos(th3(t) - 1.5708)*(1.0*cos(th2(t) - 1.5708) - 3.5208e-12*sin(th2(t) - 1.5708)) - 1.0*sin(th3(t) - 1.5708)*(3.5208e-12*cos(th2(t) - 1.5708) + 1.0*sin(th2(t) - 1.5708))) - 0.02*cos(th5(t))*(sin(th4(t) - 3.1416)*(cos(th3(t) - 1.5708)*(3.5208e-12*cos(th2(t) - 1.5708) + 1.0*sin(th2(t) - 1.5708)) + sin(th3(t) - 1.5708)*(1.0*cos(th2(t) - 1.5708) - 3.5208e-12*sin(th2(t) - 1.5708))) + cos(th4(t) - 3.1416)*(cos(th3(t) - 1.5708)*(1.0*cos(th2(t) - 1.5708) - 3.5208e-12*sin(th2(t) - 1.5708)) - 1.0*sin(th3(t) - 1.5708)*(3.5208e-12*cos(th2(t) - 1.5708) + 1.0*sin(th2(t) - 1.5708)))))*(0.38*sin(th3(t))*(3.5208e-12*cos(th2(t) - 1.5708) + 1.0*sin(th2(t) - 1.5708)) - 0.02*sin(th5(t))*(cos(th4(t) - 3.1416)*(cos(th3(t) - 1.5708)*(3.5208e-12*cos(th2(t) - 1.5708) + 1.0*sin(th2(t) - 1.5708)) + sin(th3(t) - 1.5708)*(1.0*cos(th2(t) - 1.5708) - 3.5208e-12*sin(th2(t) - 1.5708))) - 1.0*sin(th4(t) - 3.1416)*(cos(th3(t) - 1.5708)*(1.0*cos(th2(t) - 1.5708) - 3.5208e-12*sin(th2(t) - 1.5708)) - 1.0*sin(th3(t) - 1.5708)*(3.5208e-12*cos(th2(t) - 1.5708) + 1.0*sin(th2(t) - 1.5708)))) + 0.38*sin(th4(t))*(cos(th3(t) - 1.5708)*(3.5208e-12*cos(th2(t) - 1.5708) + 1.0*sin(th2(t) - 1.5708)) + sin(th3(t) - 1.5708)*(1.0*cos(th2(t) - 1.5708) - 3.5208e-12*sin(th2(t) - 1.5708))) - 0.38*cos(th4(t))*(cos(th3(t) - 1.5708)*(1.0*cos(th2(t) - 1.5708) - 3.5208e-12*sin(th2(t) - 1.5708)) - 1.0*sin(th3(t) - 1.5708)*(3.5208e-12*cos(th2(t) - 1.5708) + 1.0*sin(th2(t) - 1.5708))) - 0.38*cos(th3(t))*(1.0*cos(th2(t) - 1.5708) - 3.5208e-12*sin(th2(t) - 1.5708)) + 0.02*cos(th5(t))*(sin(th4(t) - 3.1416)*(cos(th3(t) - 1.5708)*(3.5208e-12*cos(th2(t) - 1.5708) + 1.0*sin(th2(t) - 1.5708)) + sin(th3(t) - 1.5708)*(1.0*cos(th2(t) - 1.5708) - 3.5208e-12*sin(th2(t) - 1.5708))) + cos(th4(t) - 3.1416)*(cos(th3(t) - 1.5708)*(1.0*cos(th2(t) - 1.5708) - 3.5208e-12*sin(th2(t) - 1.5708)) - 1.0*sin(th3(t) - 1.5708)*(3.5208e-12*cos(th2(t) - 1.5708) + 1.0*sin(th2(t) - 1.5708))))) + 1.3806*(0.19*sin(th4(t))*(cos(th3(t) - 1.5708)*(3.5208e-12*cos(th2(t) - 1.5708) + 1.0*sin(th2(t) - 1.5708)) + sin(th3(t) - 1.5708)*(1.0*cos(th2(t) - 1.5708) - 3.5208e-12*sin(th2(t) - 1.5708))) - 0.19*cos(th4(t))*(cos(th3(t) - 1.5708)*(1.0*cos(th2(t) - 1.5708) - 3.5208e-12*sin(th2(t) - 1.5708)) - 1.0*sin(th3(t) - 1.5708)*(3.5208e-12*cos(th2(t) - 1.5708) + 1.0*sin(th2(t) - 1.5708))))*(0.38*sin(th3(t))*(3.5208e-12*cos(th2(t) - 1.5708) + 1.0*sin(th2(t) - 1.5708)) + 0.19*sin(th4(t))*(cos(th3(t) - 1.5708)*(3.5208e-12*cos(th2(t) - 1.5708) + 1.0*sin(th2(t) - 1.5708)) + sin(th3(t) - 1.5708)*(1.0*cos(th2(t) - 1.5708) - 3.5208e-12*sin(th2(t) - 1.5708))) - 0.19*cos(th4(t))*(cos(th3(t) - 1.5708)*(1.0*cos(th2(t) - 1.5708) - 3.5208e-12*sin(th2(t) - 1.5708)) - 1.0*sin(th3(t) - 1.5708)*(3.5208e-12*cos(th2(t) - 1.5708) + 1.0*sin(th2(t) - 1.5708))) - 0.38*cos(th3(t))*(1.0*cos(th2(t) - 1.5708) - 3.5208e-12*sin(th2(t) - 1.5708))) - 1.3806*(0.19*sin(th4(t))*(sin(th3(t) - 1.5708)*(sin(th2(t) - 1.5708)*(2.6536e-6*cos(th1(t)) + 1.0*sin(th1(t))) + 1.3268e-6*cos(th2(t) - 1.5708)*cos(th1(t))) - cos(th3(t) - 1.5708)*(1.0*cos(th2(t) - 1.5708)*(2.6536e-6*cos(th1(t)) + 1.0*sin(th1(t))) - 1.3268e-6*sin(th2(t) - 1.5708)*cos(th1(t)))) - 0.19*cos(th4(t))*(cos(th3(t) - 1.5708)*(sin(th2(t) - 1.5708)*(2.6536e-6*cos(th1(t)) + 1.0*sin(th1(t))) + 1.3268e-6*cos(th2(t) - 1.5708)*cos(th1(t))) + 1.0*sin(th3(t) - 1.5708)*(1.0*cos(th2(t) - 1.5708)*(2.6536e-6*cos(th1(t)) + 1.0*sin(th1(t))) - 1.3268e-6*sin(th2(t) - 1.5708)*cos(th1(t)))))*(0.38*cos(th3(t))*(sin(th2(t) - 1.5708)*(2.6536e-6*cos(th1(t)) + 1.0*sin(th1(t))) + 1.3268e-6*cos(th2(t) - 1.5708)*cos(th1(t))) - 0.19*sin(th4(t))*(sin(th3(t) - 1.5708)*(sin(th2(t) - 1.5708)*(2.6536e-6*cos(th1(t)) + 1.0*sin(th1(t))) + 1.3268e-6*cos(th2(t) - 1.5708)*cos(th1(t))) - cos(th3(t) - 1.5708)*(1.0*cos(th2(t) - 1.5708)*(2.6536e-6*cos(th1(t)) + 1.0*sin(th1(t))) - 1.3268e-6*sin(th2(t) - 1.5708)*cos(th1(t)))) + 0.38*sin(th3(t))*(1.0*cos(th2(t) - 1.5708)*(2.6536e-6*cos(th1(t)) + 1.0*sin(th1(t))) - 1.3268e-6*sin(th2(t) - 1.5708)*cos(th1(t))) + 0.19*cos(th4(t))*(cos(th3(t) - 1.5708)*(sin(th2(t) - 1.5708)*(2.6536e-6*cos(th1(t)) + 1.0*sin(th1(t))) + 1.3268e-6*cos(th2(t) - 1.5708)*cos(th1(t))) + 1.0*sin(th3(t) - 1.5708)*(1.0*cos(th2(t) - 1.5708)*(2.6536e-6*cos(th1(t)) + 1.0*sin(th1(t))) - 1.3268e-6*sin(th2(t) - 1.5708)*cos(th1(t))))) - 0.13038*(0.38*sin(th4(t))*(sin(th3(t) - 1.5708)*(sin(th2(t) - 1.5708)*(2.6536e-6*cos(th1(t)) + 1.0*sin(th1(t))) + 1.3268e-6*cos(th2(t) - 1.5708)*cos(th1(t))) - cos(th3(t) - 1.5708)*(1.0*cos(th2(t) - 1.5708)*(2.6536e-6*cos(th1(t)) + 1.0*sin(th1(t))) - 1.3268e-6*sin(th2(t) - 1.5708)*cos(th1(t)))) - 0.02*cos(th5(t))*(sin(th4(t) - 3.1416)*(sin(th3(t) - 1.5708)*(sin(th2(t) - 1.5708)*(2.6536e-6*cos(th1(t)) + 1.0*sin(th1(t))) + 1.3268e-6*cos(th2(t) - 1.5708)*cos(th1(t))) - cos(th3(t) - 1.5708)*(1.0*cos(th2(t) - 1.5708)*(2.6536e-6*cos(th1(t)) + 1.0*sin(th1(t))) - 1.3268e-6*sin(th2(t) - 1.5708)*cos(th1(t)))) + cos(th4(t) - 3.1416)*(cos(th3(t) - 1.5708)*(sin(th2(t) - 1.5708)*(2.6536e-6*cos(th1(t)) + 1.0*sin(th1(t))) + 1.3268e-6*cos(th2(t) - 1.5708)*cos(th1(t))) + 1.0*sin(th3(t) - 1.5708)*(1.0*cos(th2(t) - 1.5708)*(2.6536e-6*cos(th1(t)) + 1.0*sin(th1(t))) - 1.3268e-6*sin(th2(t) - 1.5708)*cos(th1(t))))) - 0.38*cos(th4(t))*(cos(th3(t) - 1.5708)*(sin(th2(t) - 1.5708)*(2.6536e-6*cos(th1(t)) + 1.0*sin(th1(t))) + 1.3268e-6*cos(th2(t) - 1.5708)*cos(th1(t))) + 1.0*sin(th3(t) - 1.5708)*(1.0*cos(th2(t) - 1.5708)*(2.6536e-6*cos(th1(t)) + 1.0*sin(th1(t))) - 1.3268e-6*sin(th2(t) - 1.5708)*cos(th1(t)))) + 0.02*sin(th5(t))*(cos(th4(t) - 3.1416)*(sin(th3(t) - 1.5708)*(sin(th2(t) - 1.5708)*(2.6536e-6*cos(th1(t)) + 1.0*sin(th1(t))) + 1.3268e-6*cos(th2(t) - 1.5708)*cos(th1(t))) - cos(th3(t) - 1.5708)*(1.0*cos(th2(t) - 1.5708)*(2.6536e-6*cos(th1(t)) + 1.0*sin(th1(t))) - 1.3268e-6*sin(th2(t) - 1.5708)*cos(th1(t)))) - 1.0*sin(th4(t) - 3.1416)*(cos(th3(t) - 1.5708)*(sin(th2(t) - 1.5708)*(2.6536e-6*cos(th1(t)) + 1.0*sin(th1(t))) + 1.3268e-6*cos(th2(t) - 1.5708)*cos(th1(t))) + 1.0*sin(th3(t) - 1.5708)*(1.0*cos(th2(t) - 1.5708)*(2.6536e-6*cos(th1(t)) + 1.0*sin(th1(t))) - 1.3268e-6*sin(th2(t) - 1.5708)*cos(th1(t))))))*(0.38*cos(th3(t))*(sin(th2(t) - 1.5708)*(2.6536e-6*cos(th1(t)) + 1.0*sin(th1(t))) + 1.3268e-6*cos(th2(t) - 1.5708)*cos(th1(t))) - 0.38*sin(th4(t))*(sin(th3(t) - 1.5708)*(sin(th2(t) - 1.5708)*(2.6536e-6*cos(th1(t)) + 1.0*sin(th1(t))) + 1.3268e-6*cos(th2(t) - 1.5708)*cos(th1(t))) - cos(th3(t) - 1.5708)*(1.0*cos(th2(t) - 1.5708)*(2.6536e-6*cos(th1(t)) + 1.0*sin(th1(t))) - 1.3268e-6*sin(th2(t) - 1.5708)*cos(th1(t)))) + 0.38*sin(th3(t))*(1.0*cos(th2(t) - 1.5708)*(2.6536e-6*cos(th1(t)) + 1.0*sin(th1(t))) - 1.3268e-6*sin(th2(t) - 1.5708)*cos(th1(t))) - 0.02*cos(th5(t))*(sin(th4(t) - 3.1416)*(sin(th3(t) - 1.5708)*(sin(th2(t) - 1.5708)*(2.6536e-6*cos(th1(t)) + 1.0*sin(th1(t))) + 1.3268e-6*cos(th2(t) - 1.5708)*cos(th1(t))) - cos(th3(t) - 1.5708)*(1.0*cos(th2(t) - 1.5708)*(2.6536e-6*cos(th1(t)) + 1.0*sin(th1(t))) - 1.3268e-6*sin(th2(t) - 1.5708)*cos(th1(t)))) + cos(th4(t) - 3.1416)*(cos(th3(t) - 1.5708)*(sin(th2(t) - 1.5708)*(2.6536e-6*cos(th1(t)) + 1.0*sin(th1(t))) + 1.3268e-6*cos(th2(t) - 1.5708)*cos(th1(t))) + 1.0*sin(th3(t) - 1.5708)*(1.0*cos(th2(t) - 1.5708)*(2.6536e-6*cos(th1(t)) + 1.0*sin(th1(t))) - 1.3268e-6*sin(th2(t) - 1.5708)*cos(th1(t))))) + 0.38*cos(th4(t))*(cos(th3(t) - 1.5708)*(sin(th2(t) - 1.5708)*(2.6536e-6*cos(th1(t)) + 1.0*sin(th1(t))) + 1.3268e-6*cos(th2(t) - 1.5708)*cos(th1(t))) + 1.0*sin(th3(t) - 1.5708)*(1.0*cos(th2(t) - 1.5708)*(2.6536e-6*cos(th1(t)) + 1.0*sin(th1(t))) - 1.3268e-6*sin(th2(t) - 1.5708)*cos(th1(t)))) + 0.02*sin(th5(t))*(cos(th4(t) - 3.1416)*(sin(th3(t) - 1.5708)*(sin(th2(t) - 1.5708)*(2.6536e-6*cos(th1(t)) + 1.0*sin(th1(t))) + 1.3268e-6*cos(th2(t) - 1.5708)*cos(th1(t))) - cos(th3(t) - 1.5708)*(1.0*cos(th2(t) - 1.5708)*(2.6536e-6*cos(th1(t)) + 1.0*sin(th1(t))) - 1.3268e-6*sin(th2(t) - 1.5708)*cos(th1(t)))) - 1.0*sin(th4(t) - 3.1416)*(cos(th3(t) - 1.5708)*(sin(th2(t) - 1.5708)*(2.6536e-6*cos(th1(t)) + 1.0*sin(th1(t))) + 1.3268e-6*cos(th2(t) - 1.5708)*cos(th1(t))) + 1.0*sin(th3(t) - 1.5708)*(1.0*cos(th2(t) - 1.5708)*(2.6536e-6*cos(th1(t)) + 1.0*sin(th1(t))) - 1.3268e-6*sin(th2(t) - 1.5708)*cos(th1(t)))))) + 1.3806*(0.19*cos(th4(t))*(cos(th3(t) - 1.5708)*(sin(th2(t) - 1.5708)*(1.0*cos(th1(t)) - 2.6536e-6*sin(th1(t))) - 1.3268e-6*cos(th2(t) - 1.5708)*sin(th1(t))) + sin(th3(t) - 1.5708)*(cos(th2(t) - 1.5708)*(1.0*cos(th1(t)) - 2.6536e-6*sin(th1(t))) + 1.3268e-6*sin(th2(t) - 1.5708)*sin(th1(t)))) + 0.19*sin(th4(t))*(cos(th3(t) - 1.5708)*(cos(th2(t) - 1.5708)*(1.0*cos(th1(t)) - 2.6536e-6*sin(th1(t))) + 1.3268e-6*sin(th2(t) - 1.5708)*sin(th1(t))) - 1.0*sin(th3(t) - 1.5708)*(sin(th2(t) - 1.5708)*(1.0*cos(th1(t)) - 2.6536e-6*sin(th1(t))) - 1.3268e-6*cos(th2(t) - 1.5708)*sin(th1(t)))))*(0.19*cos(th4(t))*(cos(th3(t) - 1.5708)*(sin(th2(t) - 1.5708)*(1.0*cos(th1(t)) - 2.6536e-6*sin(th1(t))) - 1.3268e-6*cos(th2(t) - 1.5708)*sin(th1(t))) + sin(th3(t) - 1.5708)*(cos(th2(t) - 1.5708)*(1.0*cos(th1(t)) - 2.6536e-6*sin(th1(t))) + 1.3268e-6*sin(th2(t) - 1.5708)*sin(th1(t)))) + 0.38*cos(th3(t))*(sin(th2(t) - 1.5708)*(1.0*cos(th1(t)) - 2.6536e-6*sin(th1(t))) - 1.3268e-6*cos(th2(t) - 1.5708)*sin(th1(t))) + 0.38*sin(th3(t))*(cos(th2(t) - 1.5708)*(1.0*cos(th1(t)) - 2.6536e-6*sin(th1(t))) + 1.3268e-6*sin(th2(t) - 1.5708)*sin(th1(t))) + 0.19*sin(th4(t))*(cos(th3(t) - 1.5708)*(cos(th2(t) - 1.5708)*(1.0*cos(th1(t)) - 2.6536e-6*sin(th1(t))) + 1.3268e-6*sin(th2(t) - 1.5708)*sin(th1(t))) - 1.0*sin(th3(t) - 1.5708)*(sin(th2(t) - 1.5708)*(1.0*cos(th1(t)) - 2.6536e-6*sin(th1(t))) - 1.3268e-6*cos(th2(t) - 1.5708)*sin(th1(t))))) + 0.13038*(0.38*cos(th4(t))*(cos(th3(t) - 1.5708)*(sin(th2(t) - 1.5708)*(1.0*cos(th1(t)) - 2.6536e-6*sin(th1(t))) - 1.3268e-6*cos(th2(t) - 1.5708)*sin(th1(t))) + sin(th3(t) - 1.5708)*(cos(th2(t) - 1.5708)*(1.0*cos(th1(t)) - 2.6536e-6*sin(th1(t))) + 1.3268e-6*sin(th2(t) - 1.5708)*sin(th1(t)))) + 0.02*sin(th5(t))*(sin(th4(t) - 3.1416)*(cos(th3(t) - 1.5708)*(sin(th2(t) - 1.5708)*(1.0*cos(th1(t)) - 2.6536e-6*sin(th1(t))) - 1.3268e-6*cos(th2(t) - 1.5708)*sin(th1(t))) + sin(th3(t) - 1.5708)*(cos(th2(t) - 1.5708)*(1.0*cos(th1(t)) - 2.6536e-6*sin(th1(t))) + 1.3268e-6*sin(th2(t) - 1.5708)*sin(th1(t)))) + cos(th4(t) - 3.1416)*(cos(th3(t) - 1.5708)*(cos(th2(t) - 1.5708)*(1.0*cos(th1(t)) - 2.6536e-6*sin(th1(t))) + 1.3268e-6*sin(th2(t) - 1.5708)*sin(th1(t))) - 1.0*sin(th3(t) - 1.5708)*(sin(th2(t) - 1.5708)*(1.0*cos(th1(t)) - 2.6536e-6*sin(th1(t))) - 1.3268e-6*cos(th2(t) - 1.5708)*sin(th1(t))))) + 0.38*sin(th4(t))*(cos(th3(t) - 1.5708)*(cos(th2(t) - 1.5708)*(1.0*cos(th1(t)) - 2.6536e-6*sin(th1(t))) + 1.3268e-6*sin(th2(t) - 1.5708)*sin(th1(t))) - 1.0*sin(th3(t) - 1.5708)*(sin(th2(t) - 1.5708)*(1.0*cos(th1(t)) - 2.6536e-6*sin(th1(t))) - 1.3268e-6*cos(th2(t) - 1.5708)*sin(th1(t)))) + 0.02*cos(th5(t))*(cos(th4(t) - 3.1416)*(cos(th3(t) - 1.5708)*(sin(th2(t) - 1.5708)*(1.0*cos(th1(t)) - 2.6536e-6*sin(th1(t))) - 1.3268e-6*cos(th2(t) - 1.5708)*sin(th1(t))) + sin(th3(t) - 1.5708)*(cos(th2(t) - 1.5708)*(1.0*cos(th1(t)) - 2.6536e-6*sin(th1(t))) + 1.3268e-6*sin(th2(t) - 1.5708)*sin(th1(t)))) - 1.0*sin(th4(t) - 3.1416)*(cos(th3(t) - 1.5708)*(cos(th2(t) - 1.5708)*(1.0*cos(th1(t)) - 2.6536e-6*sin(th1(t))) + 1.3268e-6*sin(th2(t) - 1.5708)*sin(th1(t))) - 1.0*sin(th3(t) - 1.5708)*(sin(th2(t) - 1.5708)*(1.0*cos(th1(t)) - 2.6536e-6*sin(th1(t))) - 1.3268e-6*cos(th2(t) - 1.5708)*sin(th1(t))))))*(0.38*cos(th4(t))*(cos(th3(t) - 1.5708)*(sin(th2(t) - 1.5708)*(1.0*cos(th1(t)) - 2.6536e-6*sin(th1(t))) - 1.3268e-6*cos(th2(t) - 1.5708)*sin(th1(t))) + sin(th3(t) - 1.5708)*(cos(th2(t) - 1.5708)*(1.0*cos(th1(t)) - 2.6536e-6*sin(th1(t))) + 1.3268e-6*sin(th2(t) - 1.5708)*sin(th1(t)))) + 0.38*cos(th3(t))*(sin(th2(t) - 1.5708)*(1.0*cos(th1(t)) - 2.6536e-6*sin(th1(t))) - 1.3268e-6*cos(th2(t) - 1.5708)*sin(th1(t))) + 0.38*sin(th3(t))*(cos(th2(t) - 1.5708)*(1.0*cos(th1(t)) - 2.6536e-6*sin(th1(t))) + 1.3268e-6*sin(th2(t) - 1.5708)*sin(th1(t))) - 0.02*sin(th5(t))*(sin(th4(t) - 3.1416)*(cos(th3(t) - 1.5708)*(sin(th2(t) - 1.5708)*(1.0*cos(th1(t)) - 2.6536e-6*sin(th1(t))) - 1.3268e-6*cos(th2(t) - 1.5708)*sin(th1(t))) + sin(th3(t) - 1.5708)*(cos(th2(t) - 1.5708)*(1.0*cos(th1(t)) - 2.6536e-6*sin(th1(t))) + 1.3268e-6*sin(th2(t) - 1.5708)*sin(th1(t)))) + cos(th4(t) - 3.1416)*(cos(th3(t) - 1.5708)*(cos(th2(t) - 1.5708)*(1.0*cos(th1(t)) - 2.6536e-6*sin(th1(t))) + 1.3268e-6*sin(th2(t) - 1.5708)*sin(th1(t))) - 1.0*sin(th3(t) - 1.5708)*(sin(th2(t) - 1.5708)*(1.0*cos(th1(t)) - 2.6536e-6*sin(th1(t))) - 1.3268e-6*cos(th2(t) - 1.5708)*sin(th1(t))))) + 0.38*sin(th4(t))*(cos(th3(t) - 1.5708)*(cos(th2(t) - 1.5708)*(1.0*cos(th1(t)) - 2.6536e-6*sin(th1(t))) + 1.3268e-6*sin(th2(t) - 1.5708)*sin(th1(t))) - 1.0*sin(th3(t) - 1.5708)*(sin(th2(t) - 1.5708)*(1.0*cos(th1(t)) - 2.6536e-6*sin(th1(t))) - 1.3268e-6*cos(th2(t) - 1.5708)*sin(th1(t)))) - 0.02*cos(th5(t))*(cos(th4(t) - 3.1416)*(cos(th3(t) - 1.5708)*(sin(th2(t) - 1.5708)*(1.0*cos(th1(t)) - 2.6536e-6*sin(th1(t))) - 1.3268e-6*cos(th2(t) - 1.5708)*sin(th1(t))) + sin(th3(t) - 1.5708)*(cos(th2(t) - 1.5708)*(1.0*cos(th1(t)) - 2.6536e-6*sin(th1(t))) + 1.3268e-6*sin(th2(t) - 1.5708)*sin(th1(t)))) - 1.0*sin(th4(t) - 3.1416)*(cos(th3(t) - 1.5708)*(cos(th2(t) - 1.5708)*(1.0*cos(th1(t)) - 2.6536e-6*sin(th1(t))) + 1.3268e-6*sin(th2(t) - 1.5708)*sin(th1(t))) - 1.0*sin(th3(t) - 1.5708)*(sin(th2(t) - 1.5708)*(1.0*cos(th1(t)) - 2.6536e-6*sin(th1(t))) - 1.3268e-6*cos(th2(t) - 1.5708)*sin(th1(t)))))) + 0.042427;
M35 = 0.00018665 - 0.13038*(0.02*cos(th5(t))*(sin(th4(t) - 3.1416)*(sin(th3(t) - 1.5708)*(sin(th2(t) - 1.5708)*(2.6536e-6*cos(th1(t)) + 1.0*sin(th1(t))) + 1.3268e-6*cos(th2(t) - 1.5708)*cos(th1(t))) - cos(th3(t) - 1.5708)*(1.0*cos(th2(t) - 1.5708)*(2.6536e-6*cos(th1(t)) + 1.0*sin(th1(t))) - 1.3268e-6*sin(th2(t) - 1.5708)*cos(th1(t)))) + cos(th4(t) - 3.1416)*(cos(th3(t) - 1.5708)*(sin(th2(t) - 1.5708)*(2.6536e-6*cos(th1(t)) + 1.0*sin(th1(t))) + 1.3268e-6*cos(th2(t) - 1.5708)*cos(th1(t))) + 1.0*sin(th3(t) - 1.5708)*(1.0*cos(th2(t) - 1.5708)*(2.6536e-6*cos(th1(t)) + 1.0*sin(th1(t))) - 1.3268e-6*sin(th2(t) - 1.5708)*cos(th1(t))))) - 0.02*sin(th5(t))*(cos(th4(t) - 3.1416)*(sin(th3(t) - 1.5708)*(sin(th2(t) - 1.5708)*(2.6536e-6*cos(th1(t)) + 1.0*sin(th1(t))) + 1.3268e-6*cos(th2(t) - 1.5708)*cos(th1(t))) - cos(th3(t) - 1.5708)*(1.0*cos(th2(t) - 1.5708)*(2.6536e-6*cos(th1(t)) + 1.0*sin(th1(t))) - 1.3268e-6*sin(th2(t) - 1.5708)*cos(th1(t)))) - 1.0*sin(th4(t) - 3.1416)*(cos(th3(t) - 1.5708)*(sin(th2(t) - 1.5708)*(2.6536e-6*cos(th1(t)) + 1.0*sin(th1(t))) + 1.3268e-6*cos(th2(t) - 1.5708)*cos(th1(t))) + 1.0*sin(th3(t) - 1.5708)*(1.0*cos(th2(t) - 1.5708)*(2.6536e-6*cos(th1(t)) + 1.0*sin(th1(t))) - 1.3268e-6*sin(th2(t) - 1.5708)*cos(th1(t))))))*(0.38*cos(th3(t))*(sin(th2(t) - 1.5708)*(2.6536e-6*cos(th1(t)) + 1.0*sin(th1(t))) + 1.3268e-6*cos(th2(t) - 1.5708)*cos(th1(t))) - 0.38*sin(th4(t))*(sin(th3(t) - 1.5708)*(sin(th2(t) - 1.5708)*(2.6536e-6*cos(th1(t)) + 1.0*sin(th1(t))) + 1.3268e-6*cos(th2(t) - 1.5708)*cos(th1(t))) - cos(th3(t) - 1.5708)*(1.0*cos(th2(t) - 1.5708)*(2.6536e-6*cos(th1(t)) + 1.0*sin(th1(t))) - 1.3268e-6*sin(th2(t) - 1.5708)*cos(th1(t)))) + 0.38*sin(th3(t))*(1.0*cos(th2(t) - 1.5708)*(2.6536e-6*cos(th1(t)) + 1.0*sin(th1(t))) - 1.3268e-6*sin(th2(t) - 1.5708)*cos(th1(t))) - 0.02*cos(th5(t))*(sin(th4(t) - 3.1416)*(sin(th3(t) - 1.5708)*(sin(th2(t) - 1.5708)*(2.6536e-6*cos(th1(t)) + 1.0*sin(th1(t))) + 1.3268e-6*cos(th2(t) - 1.5708)*cos(th1(t))) - cos(th3(t) - 1.5708)*(1.0*cos(th2(t) - 1.5708)*(2.6536e-6*cos(th1(t)) + 1.0*sin(th1(t))) - 1.3268e-6*sin(th2(t) - 1.5708)*cos(th1(t)))) + cos(th4(t) - 3.1416)*(cos(th3(t) - 1.5708)*(sin(th2(t) - 1.5708)*(2.6536e-6*cos(th1(t)) + 1.0*sin(th1(t))) + 1.3268e-6*cos(th2(t) - 1.5708)*cos(th1(t))) + 1.0*sin(th3(t) - 1.5708)*(1.0*cos(th2(t) - 1.5708)*(2.6536e-6*cos(th1(t)) + 1.0*sin(th1(t))) - 1.3268e-6*sin(th2(t) - 1.5708)*cos(th1(t))))) + 0.38*cos(th4(t))*(cos(th3(t) - 1.5708)*(sin(th2(t) - 1.5708)*(2.6536e-6*cos(th1(t)) + 1.0*sin(th1(t))) + 1.3268e-6*cos(th2(t) - 1.5708)*cos(th1(t))) + 1.0*sin(th3(t) - 1.5708)*(1.0*cos(th2(t) - 1.5708)*(2.6536e-6*cos(th1(t)) + 1.0*sin(th1(t))) - 1.3268e-6*sin(th2(t) - 1.5708)*cos(th1(t)))) + 0.02*sin(th5(t))*(cos(th4(t) - 3.1416)*(sin(th3(t) - 1.5708)*(sin(th2(t) - 1.5708)*(2.6536e-6*cos(th1(t)) + 1.0*sin(th1(t))) + 1.3268e-6*cos(th2(t) - 1.5708)*cos(th1(t))) - cos(th3(t) - 1.5708)*(1.0*cos(th2(t) - 1.5708)*(2.6536e-6*cos(th1(t)) + 1.0*sin(th1(t))) - 1.3268e-6*sin(th2(t) - 1.5708)*cos(th1(t)))) - 1.0*sin(th4(t) - 3.1416)*(cos(th3(t) - 1.5708)*(sin(th2(t) - 1.5708)*(2.6536e-6*cos(th1(t)) + 1.0*sin(th1(t))) + 1.3268e-6*cos(th2(t) - 1.5708)*cos(th1(t))) + 1.0*sin(th3(t) - 1.5708)*(1.0*cos(th2(t) - 1.5708)*(2.6536e-6*cos(th1(t)) + 1.0*sin(th1(t))) - 1.3268e-6*sin(th2(t) - 1.5708)*cos(th1(t)))))) - 0.13038*(0.02*sin(th5(t))*(cos(th4(t) - 3.1416)*(cos(th3(t) - 1.5708)*(3.5208e-12*cos(th2(t) - 1.5708) + 1.0*sin(th2(t) - 1.5708)) + sin(th3(t) - 1.5708)*(1.0*cos(th2(t) - 1.5708) - 3.5208e-12*sin(th2(t) - 1.5708))) - 1.0*sin(th4(t) - 3.1416)*(cos(th3(t) - 1.5708)*(1.0*cos(th2(t) - 1.5708) - 3.5208e-12*sin(th2(t) - 1.5708)) - 1.0*sin(th3(t) - 1.5708)*(3.5208e-12*cos(th2(t) - 1.5708) + 1.0*sin(th2(t) - 1.5708)))) - 0.02*cos(th5(t))*(sin(th4(t) - 3.1416)*(cos(th3(t) - 1.5708)*(3.5208e-12*cos(th2(t) - 1.5708) + 1.0*sin(th2(t) - 1.5708)) + sin(th3(t) - 1.5708)*(1.0*cos(th2(t) - 1.5708) - 3.5208e-12*sin(th2(t) - 1.5708))) + cos(th4(t) - 3.1416)*(cos(th3(t) - 1.5708)*(1.0*cos(th2(t) - 1.5708) - 3.5208e-12*sin(th2(t) - 1.5708)) - 1.0*sin(th3(t) - 1.5708)*(3.5208e-12*cos(th2(t) - 1.5708) + 1.0*sin(th2(t) - 1.5708)))))*(0.38*sin(th3(t))*(3.5208e-12*cos(th2(t) - 1.5708) + 1.0*sin(th2(t) - 1.5708)) - 0.02*sin(th5(t))*(cos(th4(t) - 3.1416)*(cos(th3(t) - 1.5708)*(3.5208e-12*cos(th2(t) - 1.5708) + 1.0*sin(th2(t) - 1.5708)) + sin(th3(t) - 1.5708)*(1.0*cos(th2(t) - 1.5708) - 3.5208e-12*sin(th2(t) - 1.5708))) - 1.0*sin(th4(t) - 3.1416)*(cos(th3(t) - 1.5708)*(1.0*cos(th2(t) - 1.5708) - 3.5208e-12*sin(th2(t) - 1.5708)) - 1.0*sin(th3(t) - 1.5708)*(3.5208e-12*cos(th2(t) - 1.5708) + 1.0*sin(th2(t) - 1.5708)))) + 0.38*sin(th4(t))*(cos(th3(t) - 1.5708)*(3.5208e-12*cos(th2(t) - 1.5708) + 1.0*sin(th2(t) - 1.5708)) + sin(th3(t) - 1.5708)*(1.0*cos(th2(t) - 1.5708) - 3.5208e-12*sin(th2(t) - 1.5708))) - 0.38*cos(th4(t))*(cos(th3(t) - 1.5708)*(1.0*cos(th2(t) - 1.5708) - 3.5208e-12*sin(th2(t) - 1.5708)) - 1.0*sin(th3(t) - 1.5708)*(3.5208e-12*cos(th2(t) - 1.5708) + 1.0*sin(th2(t) - 1.5708))) - 0.38*cos(th3(t))*(1.0*cos(th2(t) - 1.5708) - 3.5208e-12*sin(th2(t) - 1.5708)) + 0.02*cos(th5(t))*(sin(th4(t) - 3.1416)*(cos(th3(t) - 1.5708)*(3.5208e-12*cos(th2(t) - 1.5708) + 1.0*sin(th2(t) - 1.5708)) + sin(th3(t) - 1.5708)*(1.0*cos(th2(t) - 1.5708) - 3.5208e-12*sin(th2(t) - 1.5708))) + cos(th4(t) - 3.1416)*(cos(th3(t) - 1.5708)*(1.0*cos(th2(t) - 1.5708) - 3.5208e-12*sin(th2(t) - 1.5708)) - 1.0*sin(th3(t) - 1.5708)*(3.5208e-12*cos(th2(t) - 1.5708) + 1.0*sin(th2(t) - 1.5708))))) - 0.13038*(0.02*sin(th5(t))*(sin(th4(t) - 3.1416)*(cos(th3(t) - 1.5708)*(sin(th2(t) - 1.5708)*(1.0*cos(th1(t)) - 2.6536e-6*sin(th1(t))) - 1.3268e-6*cos(th2(t) - 1.5708)*sin(th1(t))) + sin(th3(t) - 1.5708)*(cos(th2(t) - 1.5708)*(1.0*cos(th1(t)) - 2.6536e-6*sin(th1(t))) + 1.3268e-6*sin(th2(t) - 1.5708)*sin(th1(t)))) + cos(th4(t) - 3.1416)*(cos(th3(t) - 1.5708)*(cos(th2(t) - 1.5708)*(1.0*cos(th1(t)) - 2.6536e-6*sin(th1(t))) + 1.3268e-6*sin(th2(t) - 1.5708)*sin(th1(t))) - 1.0*sin(th3(t) - 1.5708)*(sin(th2(t) - 1.5708)*(1.0*cos(th1(t)) - 2.6536e-6*sin(th1(t))) - 1.3268e-6*cos(th2(t) - 1.5708)*sin(th1(t))))) + 0.02*cos(th5(t))*(cos(th4(t) - 3.1416)*(cos(th3(t) - 1.5708)*(sin(th2(t) - 1.5708)*(1.0*cos(th1(t)) - 2.6536e-6*sin(th1(t))) - 1.3268e-6*cos(th2(t) - 1.5708)*sin(th1(t))) + sin(th3(t) - 1.5708)*(cos(th2(t) - 1.5708)*(1.0*cos(th1(t)) - 2.6536e-6*sin(th1(t))) + 1.3268e-6*sin(th2(t) - 1.5708)*sin(th1(t)))) - 1.0*sin(th4(t) - 3.1416)*(cos(th3(t) - 1.5708)*(cos(th2(t) - 1.5708)*(1.0*cos(th1(t)) - 2.6536e-6*sin(th1(t))) + 1.3268e-6*sin(th2(t) - 1.5708)*sin(th1(t))) - 1.0*sin(th3(t) - 1.5708)*(sin(th2(t) - 1.5708)*(1.0*cos(th1(t)) - 2.6536e-6*sin(th1(t))) - 1.3268e-6*cos(th2(t) - 1.5708)*sin(th1(t))))))*(0.38*cos(th4(t))*(cos(th3(t) - 1.5708)*(sin(th2(t) - 1.5708)*(1.0*cos(th1(t)) - 2.6536e-6*sin(th1(t))) - 1.3268e-6*cos(th2(t) - 1.5708)*sin(th1(t))) + sin(th3(t) - 1.5708)*(cos(th2(t) - 1.5708)*(1.0*cos(th1(t)) - 2.6536e-6*sin(th1(t))) + 1.3268e-6*sin(th2(t) - 1.5708)*sin(th1(t)))) + 0.38*cos(th3(t))*(sin(th2(t) - 1.5708)*(1.0*cos(th1(t)) - 2.6536e-6*sin(th1(t))) - 1.3268e-6*cos(th2(t) - 1.5708)*sin(th1(t))) + 0.38*sin(th3(t))*(cos(th2(t) - 1.5708)*(1.0*cos(th1(t)) - 2.6536e-6*sin(th1(t))) + 1.3268e-6*sin(th2(t) - 1.5708)*sin(th1(t))) - 0.02*sin(th5(t))*(sin(th4(t) - 3.1416)*(cos(th3(t) - 1.5708)*(sin(th2(t) - 1.5708)*(1.0*cos(th1(t)) - 2.6536e-6*sin(th1(t))) - 1.3268e-6*cos(th2(t) - 1.5708)*sin(th1(t))) + sin(th3(t) - 1.5708)*(cos(th2(t) - 1.5708)*(1.0*cos(th1(t)) - 2.6536e-6*sin(th1(t))) + 1.3268e-6*sin(th2(t) - 1.5708)*sin(th1(t)))) + cos(th4(t) - 3.1416)*(cos(th3(t) - 1.5708)*(cos(th2(t) - 1.5708)*(1.0*cos(th1(t)) - 2.6536e-6*sin(th1(t))) + 1.3268e-6*sin(th2(t) - 1.5708)*sin(th1(t))) - 1.0*sin(th3(t) - 1.5708)*(sin(th2(t) - 1.5708)*(1.0*cos(th1(t)) - 2.6536e-6*sin(th1(t))) - 1.3268e-6*cos(th2(t) - 1.5708)*sin(th1(t))))) + 0.38*sin(th4(t))*(cos(th3(t) - 1.5708)*(cos(th2(t) - 1.5708)*(1.0*cos(th1(t)) - 2.6536e-6*sin(th1(t))) + 1.3268e-6*sin(th2(t) - 1.5708)*sin(th1(t))) - 1.0*sin(th3(t) - 1.5708)*(sin(th2(t) - 1.5708)*(1.0*cos(th1(t)) - 2.6536e-6*sin(th1(t))) - 1.3268e-6*cos(th2(t) - 1.5708)*sin(th1(t)))) - 0.02*cos(th5(t))*(cos(th4(t) - 3.1416)*(cos(th3(t) - 1.5708)*(sin(th2(t) - 1.5708)*(1.0*cos(th1(t)) - 2.6536e-6*sin(th1(t))) - 1.3268e-6*cos(th2(t) - 1.5708)*sin(th1(t))) + sin(th3(t) - 1.5708)*(cos(th2(t) - 1.5708)*(1.0*cos(th1(t)) - 2.6536e-6*sin(th1(t))) + 1.3268e-6*sin(th2(t) - 1.5708)*sin(th1(t)))) - 1.0*sin(th4(t) - 3.1416)*(cos(th3(t) - 1.5708)*(cos(th2(t) - 1.5708)*(1.0*cos(th1(t)) - 2.6536e-6*sin(th1(t))) + 1.3268e-6*sin(th2(t) - 1.5708)*sin(th1(t))) - 1.0*sin(th3(t) - 1.5708)*(sin(th2(t) - 1.5708)*(1.0*cos(th1(t)) - 2.6536e-6*sin(th1(t))) - 1.3268e-6*cos(th2(t) - 1.5708)*sin(th1(t))))));

M41 = 0.13038*(0.38*sin(th4(t))*(sin(th3(t) - 1.5708)*(sin(th2(t) - 1.5708)*(2.6536e-6*cos(th1(t)) + 1.0*sin(th1(t))) + 1.3268e-6*cos(th2(t) - 1.5708)*cos(th1(t))) - cos(th3(t) - 1.5708)*(1.0*cos(th2(t) - 1.5708)*(2.6536e-6*cos(th1(t)) + 1.0*sin(th1(t))) - 1.3268e-6*sin(th2(t) - 1.5708)*cos(th1(t)))) - 0.02*cos(th5(t))*(sin(th4(t) - 3.1416)*(sin(th3(t) - 1.5708)*(sin(th2(t) - 1.5708)*(2.6536e-6*cos(th1(t)) + 1.0*sin(th1(t))) + 1.3268e-6*cos(th2(t) - 1.5708)*cos(th1(t))) - cos(th3(t) - 1.5708)*(1.0*cos(th2(t) - 1.5708)*(2.6536e-6*cos(th1(t)) + 1.0*sin(th1(t))) - 1.3268e-6*sin(th2(t) - 1.5708)*cos(th1(t)))) + cos(th4(t) - 3.1416)*(cos(th3(t) - 1.5708)*(sin(th2(t) - 1.5708)*(2.6536e-6*cos(th1(t)) + 1.0*sin(th1(t))) + 1.3268e-6*cos(th2(t) - 1.5708)*cos(th1(t))) + 1.0*sin(th3(t) - 1.5708)*(1.0*cos(th2(t) - 1.5708)*(2.6536e-6*cos(th1(t)) + 1.0*sin(th1(t))) - 1.3268e-6*sin(th2(t) - 1.5708)*cos(th1(t))))) - 0.38*cos(th4(t))*(cos(th3(t) - 1.5708)*(sin(th2(t) - 1.5708)*(2.6536e-6*cos(th1(t)) + 1.0*sin(th1(t))) + 1.3268e-6*cos(th2(t) - 1.5708)*cos(th1(t))) + 1.0*sin(th3(t) - 1.5708)*(1.0*cos(th2(t) - 1.5708)*(2.6536e-6*cos(th1(t)) + 1.0*sin(th1(t))) - 1.3268e-6*sin(th2(t) - 1.5708)*cos(th1(t)))) + 0.02*sin(th5(t))*(cos(th4(t) - 3.1416)*(sin(th3(t) - 1.5708)*(sin(th2(t) - 1.5708)*(2.6536e-6*cos(th1(t)) + 1.0*sin(th1(t))) + 1.3268e-6*cos(th2(t) - 1.5708)*cos(th1(t))) - cos(th3(t) - 1.5708)*(1.0*cos(th2(t) - 1.5708)*(2.6536e-6*cos(th1(t)) + 1.0*sin(th1(t))) - 1.3268e-6*sin(th2(t) - 1.5708)*cos(th1(t)))) - 1.0*sin(th4(t) - 3.1416)*(cos(th3(t) - 1.5708)*(sin(th2(t) - 1.5708)*(2.6536e-6*cos(th1(t)) + 1.0*sin(th1(t))) + 1.3268e-6*cos(th2(t) - 1.5708)*cos(th1(t))) + 1.0*sin(th3(t) - 1.5708)*(1.0*cos(th2(t) - 1.5708)*(2.6536e-6*cos(th1(t)) + 1.0*sin(th1(t))) - 1.3268e-6*sin(th2(t) - 1.5708)*cos(th1(t))))))*(5.0418e-7*sin(th1(t))*sin(th2(t)) - 0.02*cos(th5(t))*(cos(th4(t) - 3.1416)*(cos(th3(t) - 1.5708)*(cos(th2(t) - 1.5708)*(1.0*cos(th1(t)) - 2.6536e-6*sin(th1(t))) + 1.3268e-6*sin(th2(t) - 1.5708)*sin(th1(t))) - sin(th3(t) - 1.5708)*(1.0*sin(th2(t) - 1.5708)*(1.0*cos(th1(t)) - 2.6536e-6*sin(th1(t))) - 1.3268e-6*cos(th2(t) - 1.5708)*sin(th1(t)))) + 1.0*sin(th4(t) - 3.1416)*(1.0*sin(th3(t) - 1.5708)*(cos(th2(t) - 1.5708)*(1.0*cos(th1(t)) - 2.6536e-6*sin(th1(t))) + 1.3268e-6*sin(th2(t) - 1.5708)*sin(th1(t))) + cos(th3(t) - 1.5708)*(1.0*sin(th2(t) - 1.5708)*(1.0*cos(th1(t)) - 2.6536e-6*sin(th1(t))) - 1.3268e-6*cos(th2(t) - 1.5708)*sin(th1(t))))) + 0.38*cos(th2(t))*(1.0*cos(th1(t)) - 2.6536e-6*sin(th1(t))) + 0.38*cos(th3(t))*(cos(th2(t) - 1.5708)*(1.0*cos(th1(t)) - 2.6536e-6*sin(th1(t))) + 1.3268e-6*sin(th2(t) - 1.5708)*sin(th1(t))) + 0.38*cos(th4(t))*(cos(th3(t) - 1.5708)*(cos(th2(t) - 1.5708)*(1.0*cos(th1(t)) - 2.6536e-6*sin(th1(t))) + 1.3268e-6*sin(th2(t) - 1.5708)*sin(th1(t))) - sin(th3(t) - 1.5708)*(1.0*sin(th2(t) - 1.5708)*(1.0*cos(th1(t)) - 2.6536e-6*sin(th1(t))) - 1.3268e-6*cos(th2(t) - 1.5708)*sin(th1(t)))) - 0.38*sin(th3(t))*(1.0*sin(th2(t) - 1.5708)*(1.0*cos(th1(t)) - 2.6536e-6*sin(th1(t))) - 1.3268e-6*cos(th2(t) - 1.5708)*sin(th1(t))) - 0.38*sin(th4(t))*(1.0*sin(th3(t) - 1.5708)*(cos(th2(t) - 1.5708)*(1.0*cos(th1(t)) - 2.6536e-6*sin(th1(t))) + 1.3268e-6*sin(th2(t) - 1.5708)*sin(th1(t))) + cos(th3(t) - 1.5708)*(1.0*sin(th2(t) - 1.5708)*(1.0*cos(th1(t)) - 2.6536e-6*sin(th1(t))) - 1.3268e-6*cos(th2(t) - 1.5708)*sin(th1(t)))) - 0.02*sin(th5(t))*(sin(th4(t) - 3.1416)*(cos(th3(t) - 1.5708)*(cos(th2(t) - 1.5708)*(1.0*cos(th1(t)) - 2.6536e-6*sin(th1(t))) + 1.3268e-6*sin(th2(t) - 1.5708)*sin(th1(t))) - sin(th3(t) - 1.5708)*(1.0*sin(th2(t) - 1.5708)*(1.0*cos(th1(t)) - 2.6536e-6*sin(th1(t))) - 1.3268e-6*cos(th2(t) - 1.5708)*sin(th1(t)))) - cos(th4(t) - 3.1416)*(1.0*sin(th3(t) - 1.5708)*(cos(th2(t) - 1.5708)*(1.0*cos(th1(t)) - 2.6536e-6*sin(th1(t))) + 1.3268e-6*sin(th2(t) - 1.5708)*sin(th1(t))) + cos(th3(t) - 1.5708)*(1.0*sin(th2(t) - 1.5708)*(1.0*cos(th1(t)) - 2.6536e-6*sin(th1(t))) - 1.3268e-6*cos(th2(t) - 1.5708)*sin(th1(t)))))) - 1.3806*(0.19*cos(th4(t))*(cos(th3(t) - 1.5708)*(sin(th2(t) - 1.5708)*(1.0*cos(th1(t)) - 2.6536e-6*sin(th1(t))) - 1.3268e-6*cos(th2(t) - 1.5708)*sin(th1(t))) + sin(th3(t) - 1.5708)*(cos(th2(t) - 1.5708)*(1.0*cos(th1(t)) - 2.6536e-6*sin(th1(t))) + 1.3268e-6*sin(th2(t) - 1.5708)*sin(th1(t)))) + 0.19*sin(th4(t))*(cos(th3(t) - 1.5708)*(cos(th2(t) - 1.5708)*(1.0*cos(th1(t)) - 2.6536e-6*sin(th1(t))) + 1.3268e-6*sin(th2(t) - 1.5708)*sin(th1(t))) - 1.0*sin(th3(t) - 1.5708)*(sin(th2(t) - 1.5708)*(1.0*cos(th1(t)) - 2.6536e-6*sin(th1(t))) - 1.3268e-6*cos(th2(t) - 1.5708)*sin(th1(t)))))*(5.0418e-7*cos(th1(t))*sin(th2(t)) + 0.19*sin(th4(t))*(cos(th3(t) - 1.5708)*(sin(th2(t) - 1.5708)*(2.6536e-6*cos(th1(t)) + 1.0*sin(th1(t))) + 1.3268e-6*cos(th2(t) - 1.5708)*cos(th1(t))) + sin(th3(t) - 1.5708)*(cos(th2(t) - 1.5708)*(2.6536e-6*cos(th1(t)) + 1.0*sin(th1(t))) - 1.3268e-6*sin(th2(t) - 1.5708)*cos(th1(t)))) - 0.38*cos(th3(t))*(cos(th2(t) - 1.5708)*(2.6536e-6*cos(th1(t)) + 1.0*sin(th1(t))) - 1.3268e-6*sin(th2(t) - 1.5708)*cos(th1(t))) - 0.38*cos(th2(t))*(2.6536e-6*cos(th1(t)) + 1.0*sin(th1(t))) + 0.38*sin(th3(t))*(sin(th2(t) - 1.5708)*(2.6536e-6*cos(th1(t)) + 1.0*sin(th1(t))) + 1.3268e-6*cos(th2(t) - 1.5708)*cos(th1(t))) - 0.19*cos(th4(t))*(cos(th3(t) - 1.5708)*(cos(th2(t) - 1.5708)*(2.6536e-6*cos(th1(t)) + 1.0*sin(th1(t))) - 1.3268e-6*sin(th2(t) - 1.5708)*cos(th1(t))) - 1.0*sin(th3(t) - 1.5708)*(sin(th2(t) - 1.5708)*(2.6536e-6*cos(th1(t)) + 1.0*sin(th1(t))) + 1.3268e-6*cos(th2(t) - 1.5708)*cos(th1(t))))) - 0.13038*(0.38*cos(th4(t))*(cos(th3(t) - 1.5708)*(sin(th2(t) - 1.5708)*(1.0*cos(th1(t)) - 2.6536e-6*sin(th1(t))) - 1.3268e-6*cos(th2(t) - 1.5708)*sin(th1(t))) + sin(th3(t) - 1.5708)*(cos(th2(t) - 1.5708)*(1.0*cos(th1(t)) - 2.6536e-6*sin(th1(t))) + 1.3268e-6*sin(th2(t) - 1.5708)*sin(th1(t)))) + 0.02*sin(th5(t))*(sin(th4(t) - 3.1416)*(cos(th3(t) - 1.5708)*(sin(th2(t) - 1.5708)*(1.0*cos(th1(t)) - 2.6536e-6*sin(th1(t))) - 1.3268e-6*cos(th2(t) - 1.5708)*sin(th1(t))) + sin(th3(t) - 1.5708)*(cos(th2(t) - 1.5708)*(1.0*cos(th1(t)) - 2.6536e-6*sin(th1(t))) + 1.3268e-6*sin(th2(t) - 1.5708)*sin(th1(t)))) + cos(th4(t) - 3.1416)*(cos(th3(t) - 1.5708)*(cos(th2(t) - 1.5708)*(1.0*cos(th1(t)) - 2.6536e-6*sin(th1(t))) + 1.3268e-6*sin(th2(t) - 1.5708)*sin(th1(t))) - 1.0*sin(th3(t) - 1.5708)*(sin(th2(t) - 1.5708)*(1.0*cos(th1(t)) - 2.6536e-6*sin(th1(t))) - 1.3268e-6*cos(th2(t) - 1.5708)*sin(th1(t))))) + 0.38*sin(th4(t))*(cos(th3(t) - 1.5708)*(cos(th2(t) - 1.5708)*(1.0*cos(th1(t)) - 2.6536e-6*sin(th1(t))) + 1.3268e-6*sin(th2(t) - 1.5708)*sin(th1(t))) - 1.0*sin(th3(t) - 1.5708)*(sin(th2(t) - 1.5708)*(1.0*cos(th1(t)) - 2.6536e-6*sin(th1(t))) - 1.3268e-6*cos(th2(t) - 1.5708)*sin(th1(t)))) + 0.02*cos(th5(t))*(cos(th4(t) - 3.1416)*(cos(th3(t) - 1.5708)*(sin(th2(t) - 1.5708)*(1.0*cos(th1(t)) - 2.6536e-6*sin(th1(t))) - 1.3268e-6*cos(th2(t) - 1.5708)*sin(th1(t))) + sin(th3(t) - 1.5708)*(cos(th2(t) - 1.5708)*(1.0*cos(th1(t)) - 2.6536e-6*sin(th1(t))) + 1.3268e-6*sin(th2(t) - 1.5708)*sin(th1(t)))) - 1.0*sin(th4(t) - 3.1416)*(cos(th3(t) - 1.5708)*(cos(th2(t) - 1.5708)*(1.0*cos(th1(t)) - 2.6536e-6*sin(th1(t))) + 1.3268e-6*sin(th2(t) - 1.5708)*sin(th1(t))) - 1.0*sin(th3(t) - 1.5708)*(sin(th2(t) - 1.5708)*(1.0*cos(th1(t)) - 2.6536e-6*sin(th1(t))) - 1.3268e-6*cos(th2(t) - 1.5708)*sin(th1(t))))))*(5.0418e-7*cos(th1(t))*sin(th2(t)) + 0.02*cos(th5(t))*(cos(th4(t) - 3.1416)*(cos(th3(t) - 1.5708)*(cos(th2(t) - 1.5708)*(2.6536e-6*cos(th1(t)) + 1.0*sin(th1(t))) - 1.3268e-6*sin(th2(t) - 1.5708)*cos(th1(t))) - 1.0*sin(th3(t) - 1.5708)*(sin(th2(t) - 1.5708)*(2.6536e-6*cos(th1(t)) + 1.0*sin(th1(t))) + 1.3268e-6*cos(th2(t) - 1.5708)*cos(th1(t)))) + sin(th4(t) - 3.1416)*(cos(th3(t) - 1.5708)*(sin(th2(t) - 1.5708)*(2.6536e-6*cos(th1(t)) + 1.0*sin(th1(t))) + 1.3268e-6*cos(th2(t) - 1.5708)*cos(th1(t))) + sin(th3(t) - 1.5708)*(cos(th2(t) - 1.5708)*(2.6536e-6*cos(th1(t)) + 1.0*sin(th1(t))) - 1.3268e-6*sin(th2(t) - 1.5708)*cos(th1(t))))) + 0.38*sin(th4(t))*(cos(th3(t) - 1.5708)*(sin(th2(t) - 1.5708)*(2.6536e-6*cos(th1(t)) + 1.0*sin(th1(t))) + 1.3268e-6*cos(th2(t) - 1.5708)*cos(th1(t))) + sin(th3(t) - 1.5708)*(cos(th2(t) - 1.5708)*(2.6536e-6*cos(th1(t)) + 1.0*sin(th1(t))) - 1.3268e-6*sin(th2(t) - 1.5708)*cos(th1(t)))) - 0.38*cos(th3(t))*(cos(th2(t) - 1.5708)*(2.6536e-6*cos(th1(t)) + 1.0*sin(th1(t))) - 1.3268e-6*sin(th2(t) - 1.5708)*cos(th1(t))) - 0.38*cos(th2(t))*(2.6536e-6*cos(th1(t)) + 1.0*sin(th1(t))) + 0.38*sin(th3(t))*(sin(th2(t) - 1.5708)*(2.6536e-6*cos(th1(t)) + 1.0*sin(th1(t))) + 1.3268e-6*cos(th2(t) - 1.5708)*cos(th1(t))) - 0.38*cos(th4(t))*(cos(th3(t) - 1.5708)*(cos(th2(t) - 1.5708)*(2.6536e-6*cos(th1(t)) + 1.0*sin(th1(t))) - 1.3268e-6*sin(th2(t) - 1.5708)*cos(th1(t))) - 1.0*sin(th3(t) - 1.5708)*(sin(th2(t) - 1.5708)*(2.6536e-6*cos(th1(t)) + 1.0*sin(th1(t))) + 1.3268e-6*cos(th2(t) - 1.5708)*cos(th1(t)))) + 0.02*sin(th5(t))*(1.0*sin(th4(t) - 3.1416)*(cos(th3(t) - 1.5708)*(cos(th2(t) - 1.5708)*(2.6536e-6*cos(th1(t)) + 1.0*sin(th1(t))) - 1.3268e-6*sin(th2(t) - 1.5708)*cos(th1(t))) - 1.0*sin(th3(t) - 1.5708)*(sin(th2(t) - 1.5708)*(2.6536e-6*cos(th1(t)) + 1.0*sin(th1(t))) + 1.3268e-6*cos(th2(t) - 1.5708)*cos(th1(t)))) - cos(th4(t) - 3.1416)*(cos(th3(t) - 1.5708)*(sin(th2(t) - 1.5708)*(2.6536e-6*cos(th1(t)) + 1.0*sin(th1(t))) + 1.3268e-6*cos(th2(t) - 1.5708)*cos(th1(t))) + sin(th3(t) - 1.5708)*(cos(th2(t) - 1.5708)*(2.6536e-6*cos(th1(t)) + 1.0*sin(th1(t))) - 1.3268e-6*sin(th2(t) - 1.5708)*cos(th1(t)))))) + 1.3806*(0.19*sin(th4(t))*(sin(th3(t) - 1.5708)*(sin(th2(t) - 1.5708)*(2.6536e-6*cos(th1(t)) + 1.0*sin(th1(t))) + 1.3268e-6*cos(th2(t) - 1.5708)*cos(th1(t))) - cos(th3(t) - 1.5708)*(1.0*cos(th2(t) - 1.5708)*(2.6536e-6*cos(th1(t)) + 1.0*sin(th1(t))) - 1.3268e-6*sin(th2(t) - 1.5708)*cos(th1(t)))) - 0.19*cos(th4(t))*(cos(th3(t) - 1.5708)*(sin(th2(t) - 1.5708)*(2.6536e-6*cos(th1(t)) + 1.0*sin(th1(t))) + 1.3268e-6*cos(th2(t) - 1.5708)*cos(th1(t))) + 1.0*sin(th3(t) - 1.5708)*(1.0*cos(th2(t) - 1.5708)*(2.6536e-6*cos(th1(t)) + 1.0*sin(th1(t))) - 1.3268e-6*sin(th2(t) - 1.5708)*cos(th1(t)))))*(5.0418e-7*sin(th1(t))*sin(th2(t)) + 0.38*cos(th2(t))*(1.0*cos(th1(t)) - 2.6536e-6*sin(th1(t))) + 0.38*cos(th3(t))*(cos(th2(t) - 1.5708)*(1.0*cos(th1(t)) - 2.6536e-6*sin(th1(t))) + 1.3268e-6*sin(th2(t) - 1.5708)*sin(th1(t))) + 0.19*cos(th4(t))*(cos(th3(t) - 1.5708)*(cos(th2(t) - 1.5708)*(1.0*cos(th1(t)) - 2.6536e-6*sin(th1(t))) + 1.3268e-6*sin(th2(t) - 1.5708)*sin(th1(t))) - sin(th3(t) - 1.5708)*(1.0*sin(th2(t) - 1.5708)*(1.0*cos(th1(t)) - 2.6536e-6*sin(th1(t))) - 1.3268e-6*cos(th2(t) - 1.5708)*sin(th1(t)))) - 0.38*sin(th3(t))*(1.0*sin(th2(t) - 1.5708)*(1.0*cos(th1(t)) - 2.6536e-6*sin(th1(t))) - 1.3268e-6*cos(th2(t) - 1.5708)*sin(th1(t))) - 0.19*sin(th4(t))*(1.0*sin(th3(t) - 1.5708)*(cos(th2(t) - 1.5708)*(1.0*cos(th1(t)) - 2.6536e-6*sin(th1(t))) + 1.3268e-6*sin(th2(t) - 1.5708)*sin(th1(t))) + cos(th3(t) - 1.5708)*(1.0*sin(th2(t) - 1.5708)*(1.0*cos(th1(t)) - 2.6536e-6*sin(th1(t))) - 1.3268e-6*cos(th2(t) - 1.5708)*sin(th1(t))))) + 0.042427;
M42 = 0.13038*(0.38*cos(th4(t))*(cos(th3(t) - 1.5708)*(sin(th2(t) - 1.5708)*(1.0*cos(th1(t)) - 2.6536e-6*sin(th1(t))) - 1.3268e-6*cos(th2(t) - 1.5708)*sin(th1(t))) + sin(th3(t) - 1.5708)*(cos(th2(t) - 1.5708)*(1.0*cos(th1(t)) - 2.6536e-6*sin(th1(t))) + 1.3268e-6*sin(th2(t) - 1.5708)*sin(th1(t)))) + 0.02*sin(th5(t))*(sin(th4(t) - 3.1416)*(cos(th3(t) - 1.5708)*(sin(th2(t) - 1.5708)*(1.0*cos(th1(t)) - 2.6536e-6*sin(th1(t))) - 1.3268e-6*cos(th2(t) - 1.5708)*sin(th1(t))) + sin(th3(t) - 1.5708)*(cos(th2(t) - 1.5708)*(1.0*cos(th1(t)) - 2.6536e-6*sin(th1(t))) + 1.3268e-6*sin(th2(t) - 1.5708)*sin(th1(t)))) + cos(th4(t) - 3.1416)*(cos(th3(t) - 1.5708)*(cos(th2(t) - 1.5708)*(1.0*cos(th1(t)) - 2.6536e-6*sin(th1(t))) + 1.3268e-6*sin(th2(t) - 1.5708)*sin(th1(t))) - 1.0*sin(th3(t) - 1.5708)*(sin(th2(t) - 1.5708)*(1.0*cos(th1(t)) - 2.6536e-6*sin(th1(t))) - 1.3268e-6*cos(th2(t) - 1.5708)*sin(th1(t))))) + 0.38*sin(th4(t))*(cos(th3(t) - 1.5708)*(cos(th2(t) - 1.5708)*(1.0*cos(th1(t)) - 2.6536e-6*sin(th1(t))) + 1.3268e-6*sin(th2(t) - 1.5708)*sin(th1(t))) - 1.0*sin(th3(t) - 1.5708)*(sin(th2(t) - 1.5708)*(1.0*cos(th1(t)) - 2.6536e-6*sin(th1(t))) - 1.3268e-6*cos(th2(t) - 1.5708)*sin(th1(t)))) + 0.02*cos(th5(t))*(cos(th4(t) - 3.1416)*(cos(th3(t) - 1.5708)*(sin(th2(t) - 1.5708)*(1.0*cos(th1(t)) - 2.6536e-6*sin(th1(t))) - 1.3268e-6*cos(th2(t) - 1.5708)*sin(th1(t))) + sin(th3(t) - 1.5708)*(cos(th2(t) - 1.5708)*(1.0*cos(th1(t)) - 2.6536e-6*sin(th1(t))) + 1.3268e-6*sin(th2(t) - 1.5708)*sin(th1(t)))) - 1.0*sin(th4(t) - 3.1416)*(cos(th3(t) - 1.5708)*(cos(th2(t) - 1.5708)*(1.0*cos(th1(t)) - 2.6536e-6*sin(th1(t))) + 1.3268e-6*sin(th2(t) - 1.5708)*sin(th1(t))) - 1.0*sin(th3(t) - 1.5708)*(sin(th2(t) - 1.5708)*(1.0*cos(th1(t)) - 2.6536e-6*sin(th1(t))) - 1.3268e-6*cos(th2(t) - 1.5708)*sin(th1(t))))))*(0.38*cos(th4(t))*(cos(th3(t) - 1.5708)*(sin(th2(t) - 1.5708)*(1.0*cos(th1(t)) - 2.6536e-6*sin(th1(t))) - 1.3268e-6*cos(th2(t) - 1.5708)*sin(th1(t))) + sin(th3(t) - 1.5708)*(cos(th2(t) - 1.5708)*(1.0*cos(th1(t)) - 2.6536e-6*sin(th1(t))) + 1.3268e-6*sin(th2(t) - 1.5708)*sin(th1(t)))) - 5.0418e-7*cos(th2(t))*sin(th1(t)) + 0.38*cos(th3(t))*(sin(th2(t) - 1.5708)*(1.0*cos(th1(t)) - 2.6536e-6*sin(th1(t))) - 1.3268e-6*cos(th2(t) - 1.5708)*sin(th1(t))) + 0.38*sin(th2(t))*(1.0*cos(th1(t)) - 2.6536e-6*sin(th1(t))) + 0.38*sin(th3(t))*(cos(th2(t) - 1.5708)*(1.0*cos(th1(t)) - 2.6536e-6*sin(th1(t))) + 1.3268e-6*sin(th2(t) - 1.5708)*sin(th1(t))) - 0.02*sin(th5(t))*(sin(th4(t) - 3.1416)*(cos(th3(t) - 1.5708)*(sin(th2(t) - 1.5708)*(1.0*cos(th1(t)) - 2.6536e-6*sin(th1(t))) - 1.3268e-6*cos(th2(t) - 1.5708)*sin(th1(t))) + sin(th3(t) - 1.5708)*(cos(th2(t) - 1.5708)*(1.0*cos(th1(t)) - 2.6536e-6*sin(th1(t))) + 1.3268e-6*sin(th2(t) - 1.5708)*sin(th1(t)))) + cos(th4(t) - 3.1416)*(cos(th3(t) - 1.5708)*(cos(th2(t) - 1.5708)*(1.0*cos(th1(t)) - 2.6536e-6*sin(th1(t))) + 1.3268e-6*sin(th2(t) - 1.5708)*sin(th1(t))) - 1.0*sin(th3(t) - 1.5708)*(sin(th2(t) - 1.5708)*(1.0*cos(th1(t)) - 2.6536e-6*sin(th1(t))) - 1.3268e-6*cos(th2(t) - 1.5708)*sin(th1(t))))) + 0.38*sin(th4(t))*(cos(th3(t) - 1.5708)*(cos(th2(t) - 1.5708)*(1.0*cos(th1(t)) - 2.6536e-6*sin(th1(t))) + 1.3268e-6*sin(th2(t) - 1.5708)*sin(th1(t))) - 1.0*sin(th3(t) - 1.5708)*(sin(th2(t) - 1.5708)*(1.0*cos(th1(t)) - 2.6536e-6*sin(th1(t))) - 1.3268e-6*cos(th2(t) - 1.5708)*sin(th1(t)))) - 0.02*cos(th5(t))*(cos(th4(t) - 3.1416)*(cos(th3(t) - 1.5708)*(sin(th2(t) - 1.5708)*(1.0*cos(th1(t)) - 2.6536e-6*sin(th1(t))) - 1.3268e-6*cos(th2(t) - 1.5708)*sin(th1(t))) + sin(th3(t) - 1.5708)*(cos(th2(t) - 1.5708)*(1.0*cos(th1(t)) - 2.6536e-6*sin(th1(t))) + 1.3268e-6*sin(th2(t) - 1.5708)*sin(th1(t)))) - 1.0*sin(th4(t) - 3.1416)*(cos(th3(t) - 1.5708)*(cos(th2(t) - 1.5708)*(1.0*cos(th1(t)) - 2.6536e-6*sin(th1(t))) + 1.3268e-6*sin(th2(t) - 1.5708)*sin(th1(t))) - 1.0*sin(th3(t) - 1.5708)*(sin(th2(t) - 1.5708)*(1.0*cos(th1(t)) - 2.6536e-6*sin(th1(t))) - 1.3268e-6*cos(th2(t) - 1.5708)*sin(th1(t)))))) - 0.13038*(0.02*sin(th5(t))*(cos(th4(t) - 3.1416)*(cos(th3(t) - 1.5708)*(3.5208e-12*cos(th2(t) - 1.5708) + 1.0*sin(th2(t) - 1.5708)) + sin(th3(t) - 1.5708)*(1.0*cos(th2(t) - 1.5708) - 3.5208e-12*sin(th2(t) - 1.5708))) - 1.0*sin(th4(t) - 3.1416)*(cos(th3(t) - 1.5708)*(1.0*cos(th2(t) - 1.5708) - 3.5208e-12*sin(th2(t) - 1.5708)) - 1.0*sin(th3(t) - 1.5708)*(3.5208e-12*cos(th2(t) - 1.5708) + 1.0*sin(th2(t) - 1.5708)))) + 0.38*sin(th4(t))*(cos(th3(t) - 1.5708)*(3.5208e-12*cos(th2(t) - 1.5708) + 1.0*sin(th2(t) - 1.5708)) + sin(th3(t) - 1.5708)*(1.0*cos(th2(t) - 1.5708) - 3.5208e-12*sin(th2(t) - 1.5708))) - 0.38*cos(th4(t))*(cos(th3(t) - 1.5708)*(1.0*cos(th2(t) - 1.5708) - 3.5208e-12*sin(th2(t) - 1.5708)) - 1.0*sin(th3(t) - 1.5708)*(3.5208e-12*cos(th2(t) - 1.5708) + 1.0*sin(th2(t) - 1.5708))) - 0.02*cos(th5(t))*(sin(th4(t) - 3.1416)*(cos(th3(t) - 1.5708)*(3.5208e-12*cos(th2(t) - 1.5708) + 1.0*sin(th2(t) - 1.5708)) + sin(th3(t) - 1.5708)*(1.0*cos(th2(t) - 1.5708) - 3.5208e-12*sin(th2(t) - 1.5708))) + cos(th4(t) - 3.1416)*(cos(th3(t) - 1.5708)*(1.0*cos(th2(t) - 1.5708) - 3.5208e-12*sin(th2(t) - 1.5708)) - 1.0*sin(th3(t) - 1.5708)*(3.5208e-12*cos(th2(t) - 1.5708) + 1.0*sin(th2(t) - 1.5708)))))*(0.38*cos(th2(t)) - 1.3379e-12*sin(th2(t)) - 0.38*sin(th3(t))*(3.5208e-12*cos(th2(t) - 1.5708) + 1.0*sin(th2(t) - 1.5708)) + 0.02*sin(th5(t))*(cos(th4(t) - 3.1416)*(cos(th3(t) - 1.5708)*(3.5208e-12*cos(th2(t) - 1.5708) + 1.0*sin(th2(t) - 1.5708)) + sin(th3(t) - 1.5708)*(1.0*cos(th2(t) - 1.5708) - 3.5208e-12*sin(th2(t) - 1.5708))) - 1.0*sin(th4(t) - 3.1416)*(cos(th3(t) - 1.5708)*(1.0*cos(th2(t) - 1.5708) - 3.5208e-12*sin(th2(t) - 1.5708)) - 1.0*sin(th3(t) - 1.5708)*(3.5208e-12*cos(th2(t) - 1.5708) + 1.0*sin(th2(t) - 1.5708)))) - 0.38*sin(th4(t))*(cos(th3(t) - 1.5708)*(3.5208e-12*cos(th2(t) - 1.5708) + 1.0*sin(th2(t) - 1.5708)) + sin(th3(t) - 1.5708)*(1.0*cos(th2(t) - 1.5708) - 3.5208e-12*sin(th2(t) - 1.5708))) + 0.38*cos(th4(t))*(cos(th3(t) - 1.5708)*(1.0*cos(th2(t) - 1.5708) - 3.5208e-12*sin(th2(t) - 1.5708)) - 1.0*sin(th3(t) - 1.5708)*(3.5208e-12*cos(th2(t) - 1.5708) + 1.0*sin(th2(t) - 1.5708))) + 0.38*cos(th3(t))*(1.0*cos(th2(t) - 1.5708) - 3.5208e-12*sin(th2(t) - 1.5708)) - 0.02*cos(th5(t))*(sin(th4(t) - 3.1416)*(cos(th3(t) - 1.5708)*(3.5208e-12*cos(th2(t) - 1.5708) + 1.0*sin(th2(t) - 1.5708)) + sin(th3(t) - 1.5708)*(1.0*cos(th2(t) - 1.5708) - 3.5208e-12*sin(th2(t) - 1.5708))) + cos(th4(t) - 3.1416)*(cos(th3(t) - 1.5708)*(1.0*cos(th2(t) - 1.5708) - 3.5208e-12*sin(th2(t) - 1.5708)) - 1.0*sin(th3(t) - 1.5708)*(3.5208e-12*cos(th2(t) - 1.5708) + 1.0*sin(th2(t) - 1.5708))))) - 1.3806*(0.19*sin(th4(t))*(sin(th3(t) - 1.5708)*(sin(th2(t) - 1.5708)*(2.6536e-6*cos(th1(t)) + 1.0*sin(th1(t))) + 1.3268e-6*cos(th2(t) - 1.5708)*cos(th1(t))) - cos(th3(t) - 1.5708)*(1.0*cos(th2(t) - 1.5708)*(2.6536e-6*cos(th1(t)) + 1.0*sin(th1(t))) - 1.3268e-6*sin(th2(t) - 1.5708)*cos(th1(t)))) - 0.19*cos(th4(t))*(cos(th3(t) - 1.5708)*(sin(th2(t) - 1.5708)*(2.6536e-6*cos(th1(t)) + 1.0*sin(th1(t))) + 1.3268e-6*cos(th2(t) - 1.5708)*cos(th1(t))) + 1.0*sin(th3(t) - 1.5708)*(1.0*cos(th2(t) - 1.5708)*(2.6536e-6*cos(th1(t)) + 1.0*sin(th1(t))) - 1.3268e-6*sin(th2(t) - 1.5708)*cos(th1(t)))))*(0.38*cos(th3(t))*(sin(th2(t) - 1.5708)*(2.6536e-6*cos(th1(t)) + 1.0*sin(th1(t))) + 1.3268e-6*cos(th2(t) - 1.5708)*cos(th1(t))) + 0.38*sin(th2(t))*(2.6536e-6*cos(th1(t)) + 1.0*sin(th1(t))) - 0.19*sin(th4(t))*(sin(th3(t) - 1.5708)*(sin(th2(t) - 1.5708)*(2.6536e-6*cos(th1(t)) + 1.0*sin(th1(t))) + 1.3268e-6*cos(th2(t) - 1.5708)*cos(th1(t))) - cos(th3(t) - 1.5708)*(1.0*cos(th2(t) - 1.5708)*(2.6536e-6*cos(th1(t)) + 1.0*sin(th1(t))) - 1.3268e-6*sin(th2(t) - 1.5708)*cos(th1(t)))) + 0.38*sin(th3(t))*(1.0*cos(th2(t) - 1.5708)*(2.6536e-6*cos(th1(t)) + 1.0*sin(th1(t))) - 1.3268e-6*sin(th2(t) - 1.5708)*cos(th1(t))) + 0.19*cos(th4(t))*(cos(th3(t) - 1.5708)*(sin(th2(t) - 1.5708)*(2.6536e-6*cos(th1(t)) + 1.0*sin(th1(t))) + 1.3268e-6*cos(th2(t) - 1.5708)*cos(th1(t))) + 1.0*sin(th3(t) - 1.5708)*(1.0*cos(th2(t) - 1.5708)*(2.6536e-6*cos(th1(t)) + 1.0*sin(th1(t))) - 1.3268e-6*sin(th2(t) - 1.5708)*cos(th1(t)))) + 5.0418e-7*cos(th1(t))*cos(th2(t))) - 1.3806*(0.19*sin(th4(t))*(cos(th3(t) - 1.5708)*(3.5208e-12*cos(th2(t) - 1.5708) + 1.0*sin(th2(t) - 1.5708)) + sin(th3(t) - 1.5708)*(1.0*cos(th2(t) - 1.5708) - 3.5208e-12*sin(th2(t) - 1.5708))) - 0.19*cos(th4(t))*(cos(th3(t) - 1.5708)*(1.0*cos(th2(t) - 1.5708) - 3.5208e-12*sin(th2(t) - 1.5708)) - 1.0*sin(th3(t) - 1.5708)*(3.5208e-12*cos(th2(t) - 1.5708) + 1.0*sin(th2(t) - 1.5708))))*(0.38*cos(th2(t)) - 1.3379e-12*sin(th2(t)) - 0.38*sin(th3(t))*(3.5208e-12*cos(th2(t) - 1.5708) + 1.0*sin(th2(t) - 1.5708)) - 0.19*sin(th4(t))*(cos(th3(t) - 1.5708)*(3.5208e-12*cos(th2(t) - 1.5708) + 1.0*sin(th2(t) - 1.5708)) + sin(th3(t) - 1.5708)*(1.0*cos(th2(t) - 1.5708) - 3.5208e-12*sin(th2(t) - 1.5708))) + 0.19*cos(th4(t))*(cos(th3(t) - 1.5708)*(1.0*cos(th2(t) - 1.5708) - 3.5208e-12*sin(th2(t) - 1.5708)) - 1.0*sin(th3(t) - 1.5708)*(3.5208e-12*cos(th2(t) - 1.5708) + 1.0*sin(th2(t) - 1.5708))) + 0.38*cos(th3(t))*(1.0*cos(th2(t) - 1.5708) - 3.5208e-12*sin(th2(t) - 1.5708))) - 0.13038*(0.38*sin(th4(t))*(sin(th3(t) - 1.5708)*(sin(th2(t) - 1.5708)*(2.6536e-6*cos(th1(t)) + 1.0*sin(th1(t))) + 1.3268e-6*cos(th2(t) - 1.5708)*cos(th1(t))) - cos(th3(t) - 1.5708)*(1.0*cos(th2(t) - 1.5708)*(2.6536e-6*cos(th1(t)) + 1.0*sin(th1(t))) - 1.3268e-6*sin(th2(t) - 1.5708)*cos(th1(t)))) - 0.02*cos(th5(t))*(sin(th4(t) - 3.1416)*(sin(th3(t) - 1.5708)*(sin(th2(t) - 1.5708)*(2.6536e-6*cos(th1(t)) + 1.0*sin(th1(t))) + 1.3268e-6*cos(th2(t) - 1.5708)*cos(th1(t))) - cos(th3(t) - 1.5708)*(1.0*cos(th2(t) - 1.5708)*(2.6536e-6*cos(th1(t)) + 1.0*sin(th1(t))) - 1.3268e-6*sin(th2(t) - 1.5708)*cos(th1(t)))) + cos(th4(t) - 3.1416)*(cos(th3(t) - 1.5708)*(sin(th2(t) - 1.5708)*(2.6536e-6*cos(th1(t)) + 1.0*sin(th1(t))) + 1.3268e-6*cos(th2(t) - 1.5708)*cos(th1(t))) + 1.0*sin(th3(t) - 1.5708)*(1.0*cos(th2(t) - 1.5708)*(2.6536e-6*cos(th1(t)) + 1.0*sin(th1(t))) - 1.3268e-6*sin(th2(t) - 1.5708)*cos(th1(t))))) - 0.38*cos(th4(t))*(cos(th3(t) - 1.5708)*(sin(th2(t) - 1.5708)*(2.6536e-6*cos(th1(t)) + 1.0*sin(th1(t))) + 1.3268e-6*cos(th2(t) - 1.5708)*cos(th1(t))) + 1.0*sin(th3(t) - 1.5708)*(1.0*cos(th2(t) - 1.5708)*(2.6536e-6*cos(th1(t)) + 1.0*sin(th1(t))) - 1.3268e-6*sin(th2(t) - 1.5708)*cos(th1(t)))) + 0.02*sin(th5(t))*(cos(th4(t) - 3.1416)*(sin(th3(t) - 1.5708)*(sin(th2(t) - 1.5708)*(2.6536e-6*cos(th1(t)) + 1.0*sin(th1(t))) + 1.3268e-6*cos(th2(t) - 1.5708)*cos(th1(t))) - cos(th3(t) - 1.5708)*(1.0*cos(th2(t) - 1.5708)*(2.6536e-6*cos(th1(t)) + 1.0*sin(th1(t))) - 1.3268e-6*sin(th2(t) - 1.5708)*cos(th1(t)))) - 1.0*sin(th4(t) - 3.1416)*(cos(th3(t) - 1.5708)*(sin(th2(t) - 1.5708)*(2.6536e-6*cos(th1(t)) + 1.0*sin(th1(t))) + 1.3268e-6*cos(th2(t) - 1.5708)*cos(th1(t))) + 1.0*sin(th3(t) - 1.5708)*(1.0*cos(th2(t) - 1.5708)*(2.6536e-6*cos(th1(t)) + 1.0*sin(th1(t))) - 1.3268e-6*sin(th2(t) - 1.5708)*cos(th1(t))))))*(0.38*cos(th3(t))*(sin(th2(t) - 1.5708)*(2.6536e-6*cos(th1(t)) + 1.0*sin(th1(t))) + 1.3268e-6*cos(th2(t) - 1.5708)*cos(th1(t))) + 0.38*sin(th2(t))*(2.6536e-6*cos(th1(t)) + 1.0*sin(th1(t))) - 0.38*sin(th4(t))*(sin(th3(t) - 1.5708)*(sin(th2(t) - 1.5708)*(2.6536e-6*cos(th1(t)) + 1.0*sin(th1(t))) + 1.3268e-6*cos(th2(t) - 1.5708)*cos(th1(t))) - cos(th3(t) - 1.5708)*(1.0*cos(th2(t) - 1.5708)*(2.6536e-6*cos(th1(t)) + 1.0*sin(th1(t))) - 1.3268e-6*sin(th2(t) - 1.5708)*cos(th1(t)))) + 0.38*sin(th3(t))*(1.0*cos(th2(t) - 1.5708)*(2.6536e-6*cos(th1(t)) + 1.0*sin(th1(t))) - 1.3268e-6*sin(th2(t) - 1.5708)*cos(th1(t))) - 0.02*cos(th5(t))*(sin(th4(t) - 3.1416)*(sin(th3(t) - 1.5708)*(sin(th2(t) - 1.5708)*(2.6536e-6*cos(th1(t)) + 1.0*sin(th1(t))) + 1.3268e-6*cos(th2(t) - 1.5708)*cos(th1(t))) - cos(th3(t) - 1.5708)*(1.0*cos(th2(t) - 1.5708)*(2.6536e-6*cos(th1(t)) + 1.0*sin(th1(t))) - 1.3268e-6*sin(th2(t) - 1.5708)*cos(th1(t)))) + cos(th4(t) - 3.1416)*(cos(th3(t) - 1.5708)*(sin(th2(t) - 1.5708)*(2.6536e-6*cos(th1(t)) + 1.0*sin(th1(t))) + 1.3268e-6*cos(th2(t) - 1.5708)*cos(th1(t))) + 1.0*sin(th3(t) - 1.5708)*(1.0*cos(th2(t) - 1.5708)*(2.6536e-6*cos(th1(t)) + 1.0*sin(th1(t))) - 1.3268e-6*sin(th2(t) - 1.5708)*cos(th1(t))))) + 0.38*cos(th4(t))*(cos(th3(t) - 1.5708)*(sin(th2(t) - 1.5708)*(2.6536e-6*cos(th1(t)) + 1.0*sin(th1(t))) + 1.3268e-6*cos(th2(t) - 1.5708)*cos(th1(t))) + 1.0*sin(th3(t) - 1.5708)*(1.0*cos(th2(t) - 1.5708)*(2.6536e-6*cos(th1(t)) + 1.0*sin(th1(t))) - 1.3268e-6*sin(th2(t) - 1.5708)*cos(th1(t)))) + 0.02*sin(th5(t))*(cos(th4(t) - 3.1416)*(sin(th3(t) - 1.5708)*(sin(th2(t) - 1.5708)*(2.6536e-6*cos(th1(t)) + 1.0*sin(th1(t))) + 1.3268e-6*cos(th2(t) - 1.5708)*cos(th1(t))) - cos(th3(t) - 1.5708)*(1.0*cos(th2(t) - 1.5708)*(2.6536e-6*cos(th1(t)) + 1.0*sin(th1(t))) - 1.3268e-6*sin(th2(t) - 1.5708)*cos(th1(t)))) - 1.0*sin(th4(t) - 3.1416)*(cos(th3(t) - 1.5708)*(sin(th2(t) - 1.5708)*(2.6536e-6*cos(th1(t)) + 1.0*sin(th1(t))) + 1.3268e-6*cos(th2(t) - 1.5708)*cos(th1(t))) + 1.0*sin(th3(t) - 1.5708)*(1.0*cos(th2(t) - 1.5708)*(2.6536e-6*cos(th1(t)) + 1.0*sin(th1(t))) - 1.3268e-6*sin(th2(t) - 1.5708)*cos(th1(t))))) + 5.0418e-7*cos(th1(t))*cos(th2(t))) + 1.3806*(0.19*cos(th4(t))*(cos(th3(t) - 1.5708)*(sin(th2(t) - 1.5708)*(1.0*cos(th1(t)) - 2.6536e-6*sin(th1(t))) - 1.3268e-6*cos(th2(t) - 1.5708)*sin(th1(t))) + sin(th3(t) - 1.5708)*(cos(th2(t) - 1.5708)*(1.0*cos(th1(t)) - 2.6536e-6*sin(th1(t))) + 1.3268e-6*sin(th2(t) - 1.5708)*sin(th1(t)))) + 0.19*sin(th4(t))*(cos(th3(t) - 1.5708)*(cos(th2(t) - 1.5708)*(1.0*cos(th1(t)) - 2.6536e-6*sin(th1(t))) + 1.3268e-6*sin(th2(t) - 1.5708)*sin(th1(t))) - 1.0*sin(th3(t) - 1.5708)*(sin(th2(t) - 1.5708)*(1.0*cos(th1(t)) - 2.6536e-6*sin(th1(t))) - 1.3268e-6*cos(th2(t) - 1.5708)*sin(th1(t)))))*(0.19*cos(th4(t))*(cos(th3(t) - 1.5708)*(sin(th2(t) - 1.5708)*(1.0*cos(th1(t)) - 2.6536e-6*sin(th1(t))) - 1.3268e-6*cos(th2(t) - 1.5708)*sin(th1(t))) + sin(th3(t) - 1.5708)*(cos(th2(t) - 1.5708)*(1.0*cos(th1(t)) - 2.6536e-6*sin(th1(t))) + 1.3268e-6*sin(th2(t) - 1.5708)*sin(th1(t)))) - 5.0418e-7*cos(th2(t))*sin(th1(t)) + 0.38*cos(th3(t))*(sin(th2(t) - 1.5708)*(1.0*cos(th1(t)) - 2.6536e-6*sin(th1(t))) - 1.3268e-6*cos(th2(t) - 1.5708)*sin(th1(t))) + 0.38*sin(th2(t))*(1.0*cos(th1(t)) - 2.6536e-6*sin(th1(t))) + 0.38*sin(th3(t))*(cos(th2(t) - 1.5708)*(1.0*cos(th1(t)) - 2.6536e-6*sin(th1(t))) + 1.3268e-6*sin(th2(t) - 1.5708)*sin(th1(t))) + 0.19*sin(th4(t))*(cos(th3(t) - 1.5708)*(cos(th2(t) - 1.5708)*(1.0*cos(th1(t)) - 2.6536e-6*sin(th1(t))) + 1.3268e-6*sin(th2(t) - 1.5708)*sin(th1(t))) - 1.0*sin(th3(t) - 1.5708)*(sin(th2(t) - 1.5708)*(1.0*cos(th1(t)) - 2.6536e-6*sin(th1(t))) - 1.3268e-6*cos(th2(t) - 1.5708)*sin(th1(t))))) + 0.042427;
M43 = 0.13038*(0.02*sin(th5(t))*(cos(th4(t) - 3.1416)*(cos(th3(t) - 1.5708)*(3.5208e-12*cos(th2(t) - 1.5708) + 1.0*sin(th2(t) - 1.5708)) + sin(th3(t) - 1.5708)*(1.0*cos(th2(t) - 1.5708) - 3.5208e-12*sin(th2(t) - 1.5708))) - 1.0*sin(th4(t) - 3.1416)*(cos(th3(t) - 1.5708)*(1.0*cos(th2(t) - 1.5708) - 3.5208e-12*sin(th2(t) - 1.5708)) - 1.0*sin(th3(t) - 1.5708)*(3.5208e-12*cos(th2(t) - 1.5708) + 1.0*sin(th2(t) - 1.5708)))) + 0.38*sin(th4(t))*(cos(th3(t) - 1.5708)*(3.5208e-12*cos(th2(t) - 1.5708) + 1.0*sin(th2(t) - 1.5708)) + sin(th3(t) - 1.5708)*(1.0*cos(th2(t) - 1.5708) - 3.5208e-12*sin(th2(t) - 1.5708))) - 0.38*cos(th4(t))*(cos(th3(t) - 1.5708)*(1.0*cos(th2(t) - 1.5708) - 3.5208e-12*sin(th2(t) - 1.5708)) - 1.0*sin(th3(t) - 1.5708)*(3.5208e-12*cos(th2(t) - 1.5708) + 1.0*sin(th2(t) - 1.5708))) - 0.02*cos(th5(t))*(sin(th4(t) - 3.1416)*(cos(th3(t) - 1.5708)*(3.5208e-12*cos(th2(t) - 1.5708) + 1.0*sin(th2(t) - 1.5708)) + sin(th3(t) - 1.5708)*(1.0*cos(th2(t) - 1.5708) - 3.5208e-12*sin(th2(t) - 1.5708))) + cos(th4(t) - 3.1416)*(cos(th3(t) - 1.5708)*(1.0*cos(th2(t) - 1.5708) - 3.5208e-12*sin(th2(t) - 1.5708)) - 1.0*sin(th3(t) - 1.5708)*(3.5208e-12*cos(th2(t) - 1.5708) + 1.0*sin(th2(t) - 1.5708)))))*(0.38*sin(th3(t))*(3.5208e-12*cos(th2(t) - 1.5708) + 1.0*sin(th2(t) - 1.5708)) - 0.02*sin(th5(t))*(cos(th4(t) - 3.1416)*(cos(th3(t) - 1.5708)*(3.5208e-12*cos(th2(t) - 1.5708) + 1.0*sin(th2(t) - 1.5708)) + sin(th3(t) - 1.5708)*(1.0*cos(th2(t) - 1.5708) - 3.5208e-12*sin(th2(t) - 1.5708))) - 1.0*sin(th4(t) - 3.1416)*(cos(th3(t) - 1.5708)*(1.0*cos(th2(t) - 1.5708) - 3.5208e-12*sin(th2(t) - 1.5708)) - 1.0*sin(th3(t) - 1.5708)*(3.5208e-12*cos(th2(t) - 1.5708) + 1.0*sin(th2(t) - 1.5708)))) + 0.38*sin(th4(t))*(cos(th3(t) - 1.5708)*(3.5208e-12*cos(th2(t) - 1.5708) + 1.0*sin(th2(t) - 1.5708)) + sin(th3(t) - 1.5708)*(1.0*cos(th2(t) - 1.5708) - 3.5208e-12*sin(th2(t) - 1.5708))) - 0.38*cos(th4(t))*(cos(th3(t) - 1.5708)*(1.0*cos(th2(t) - 1.5708) - 3.5208e-12*sin(th2(t) - 1.5708)) - 1.0*sin(th3(t) - 1.5708)*(3.5208e-12*cos(th2(t) - 1.5708) + 1.0*sin(th2(t) - 1.5708))) - 0.38*cos(th3(t))*(1.0*cos(th2(t) - 1.5708) - 3.5208e-12*sin(th2(t) - 1.5708)) + 0.02*cos(th5(t))*(sin(th4(t) - 3.1416)*(cos(th3(t) - 1.5708)*(3.5208e-12*cos(th2(t) - 1.5708) + 1.0*sin(th2(t) - 1.5708)) + sin(th3(t) - 1.5708)*(1.0*cos(th2(t) - 1.5708) - 3.5208e-12*sin(th2(t) - 1.5708))) + cos(th4(t) - 3.1416)*(cos(th3(t) - 1.5708)*(1.0*cos(th2(t) - 1.5708) - 3.5208e-12*sin(th2(t) - 1.5708)) - 1.0*sin(th3(t) - 1.5708)*(3.5208e-12*cos(th2(t) - 1.5708) + 1.0*sin(th2(t) - 1.5708))))) + 1.3806*(0.19*sin(th4(t))*(cos(th3(t) - 1.5708)*(3.5208e-12*cos(th2(t) - 1.5708) + 1.0*sin(th2(t) - 1.5708)) + sin(th3(t) - 1.5708)*(1.0*cos(th2(t) - 1.5708) - 3.5208e-12*sin(th2(t) - 1.5708))) - 0.19*cos(th4(t))*(cos(th3(t) - 1.5708)*(1.0*cos(th2(t) - 1.5708) - 3.5208e-12*sin(th2(t) - 1.5708)) - 1.0*sin(th3(t) - 1.5708)*(3.5208e-12*cos(th2(t) - 1.5708) + 1.0*sin(th2(t) - 1.5708))))*(0.38*sin(th3(t))*(3.5208e-12*cos(th2(t) - 1.5708) + 1.0*sin(th2(t) - 1.5708)) + 0.19*sin(th4(t))*(cos(th3(t) - 1.5708)*(3.5208e-12*cos(th2(t) - 1.5708) + 1.0*sin(th2(t) - 1.5708)) + sin(th3(t) - 1.5708)*(1.0*cos(th2(t) - 1.5708) - 3.5208e-12*sin(th2(t) - 1.5708))) - 0.19*cos(th4(t))*(cos(th3(t) - 1.5708)*(1.0*cos(th2(t) - 1.5708) - 3.5208e-12*sin(th2(t) - 1.5708)) - 1.0*sin(th3(t) - 1.5708)*(3.5208e-12*cos(th2(t) - 1.5708) + 1.0*sin(th2(t) - 1.5708))) - 0.38*cos(th3(t))*(1.0*cos(th2(t) - 1.5708) - 3.5208e-12*sin(th2(t) - 1.5708))) - 1.3806*(0.19*sin(th4(t))*(sin(th3(t) - 1.5708)*(sin(th2(t) - 1.5708)*(2.6536e-6*cos(th1(t)) + 1.0*sin(th1(t))) + 1.3268e-6*cos(th2(t) - 1.5708)*cos(th1(t))) - cos(th3(t) - 1.5708)*(1.0*cos(th2(t) - 1.5708)*(2.6536e-6*cos(th1(t)) + 1.0*sin(th1(t))) - 1.3268e-6*sin(th2(t) - 1.5708)*cos(th1(t)))) - 0.19*cos(th4(t))*(cos(th3(t) - 1.5708)*(sin(th2(t) - 1.5708)*(2.6536e-6*cos(th1(t)) + 1.0*sin(th1(t))) + 1.3268e-6*cos(th2(t) - 1.5708)*cos(th1(t))) + 1.0*sin(th3(t) - 1.5708)*(1.0*cos(th2(t) - 1.5708)*(2.6536e-6*cos(th1(t)) + 1.0*sin(th1(t))) - 1.3268e-6*sin(th2(t) - 1.5708)*cos(th1(t)))))*(0.38*cos(th3(t))*(sin(th2(t) - 1.5708)*(2.6536e-6*cos(th1(t)) + 1.0*sin(th1(t))) + 1.3268e-6*cos(th2(t) - 1.5708)*cos(th1(t))) - 0.19*sin(th4(t))*(sin(th3(t) - 1.5708)*(sin(th2(t) - 1.5708)*(2.6536e-6*cos(th1(t)) + 1.0*sin(th1(t))) + 1.3268e-6*cos(th2(t) - 1.5708)*cos(th1(t))) - cos(th3(t) - 1.5708)*(1.0*cos(th2(t) - 1.5708)*(2.6536e-6*cos(th1(t)) + 1.0*sin(th1(t))) - 1.3268e-6*sin(th2(t) - 1.5708)*cos(th1(t)))) + 0.38*sin(th3(t))*(1.0*cos(th2(t) - 1.5708)*(2.6536e-6*cos(th1(t)) + 1.0*sin(th1(t))) - 1.3268e-6*sin(th2(t) - 1.5708)*cos(th1(t))) + 0.19*cos(th4(t))*(cos(th3(t) - 1.5708)*(sin(th2(t) - 1.5708)*(2.6536e-6*cos(th1(t)) + 1.0*sin(th1(t))) + 1.3268e-6*cos(th2(t) - 1.5708)*cos(th1(t))) + 1.0*sin(th3(t) - 1.5708)*(1.0*cos(th2(t) - 1.5708)*(2.6536e-6*cos(th1(t)) + 1.0*sin(th1(t))) - 1.3268e-6*sin(th2(t) - 1.5708)*cos(th1(t))))) - 0.13038*(0.38*sin(th4(t))*(sin(th3(t) - 1.5708)*(sin(th2(t) - 1.5708)*(2.6536e-6*cos(th1(t)) + 1.0*sin(th1(t))) + 1.3268e-6*cos(th2(t) - 1.5708)*cos(th1(t))) - cos(th3(t) - 1.5708)*(1.0*cos(th2(t) - 1.5708)*(2.6536e-6*cos(th1(t)) + 1.0*sin(th1(t))) - 1.3268e-6*sin(th2(t) - 1.5708)*cos(th1(t)))) - 0.02*cos(th5(t))*(sin(th4(t) - 3.1416)*(sin(th3(t) - 1.5708)*(sin(th2(t) - 1.5708)*(2.6536e-6*cos(th1(t)) + 1.0*sin(th1(t))) + 1.3268e-6*cos(th2(t) - 1.5708)*cos(th1(t))) - cos(th3(t) - 1.5708)*(1.0*cos(th2(t) - 1.5708)*(2.6536e-6*cos(th1(t)) + 1.0*sin(th1(t))) - 1.3268e-6*sin(th2(t) - 1.5708)*cos(th1(t)))) + cos(th4(t) - 3.1416)*(cos(th3(t) - 1.5708)*(sin(th2(t) - 1.5708)*(2.6536e-6*cos(th1(t)) + 1.0*sin(th1(t))) + 1.3268e-6*cos(th2(t) - 1.5708)*cos(th1(t))) + 1.0*sin(th3(t) - 1.5708)*(1.0*cos(th2(t) - 1.5708)*(2.6536e-6*cos(th1(t)) + 1.0*sin(th1(t))) - 1.3268e-6*sin(th2(t) - 1.5708)*cos(th1(t))))) - 0.38*cos(th4(t))*(cos(th3(t) - 1.5708)*(sin(th2(t) - 1.5708)*(2.6536e-6*cos(th1(t)) + 1.0*sin(th1(t))) + 1.3268e-6*cos(th2(t) - 1.5708)*cos(th1(t))) + 1.0*sin(th3(t) - 1.5708)*(1.0*cos(th2(t) - 1.5708)*(2.6536e-6*cos(th1(t)) + 1.0*sin(th1(t))) - 1.3268e-6*sin(th2(t) - 1.5708)*cos(th1(t)))) + 0.02*sin(th5(t))*(cos(th4(t) - 3.1416)*(sin(th3(t) - 1.5708)*(sin(th2(t) - 1.5708)*(2.6536e-6*cos(th1(t)) + 1.0*sin(th1(t))) + 1.3268e-6*cos(th2(t) - 1.5708)*cos(th1(t))) - cos(th3(t) - 1.5708)*(1.0*cos(th2(t) - 1.5708)*(2.6536e-6*cos(th1(t)) + 1.0*sin(th1(t))) - 1.3268e-6*sin(th2(t) - 1.5708)*cos(th1(t)))) - 1.0*sin(th4(t) - 3.1416)*(cos(th3(t) - 1.5708)*(sin(th2(t) - 1.5708)*(2.6536e-6*cos(th1(t)) + 1.0*sin(th1(t))) + 1.3268e-6*cos(th2(t) - 1.5708)*cos(th1(t))) + 1.0*sin(th3(t) - 1.5708)*(1.0*cos(th2(t) - 1.5708)*(2.6536e-6*cos(th1(t)) + 1.0*sin(th1(t))) - 1.3268e-6*sin(th2(t) - 1.5708)*cos(th1(t))))))*(0.38*cos(th3(t))*(sin(th2(t) - 1.5708)*(2.6536e-6*cos(th1(t)) + 1.0*sin(th1(t))) + 1.3268e-6*cos(th2(t) - 1.5708)*cos(th1(t))) - 0.38*sin(th4(t))*(sin(th3(t) - 1.5708)*(sin(th2(t) - 1.5708)*(2.6536e-6*cos(th1(t)) + 1.0*sin(th1(t))) + 1.3268e-6*cos(th2(t) - 1.5708)*cos(th1(t))) - cos(th3(t) - 1.5708)*(1.0*cos(th2(t) - 1.5708)*(2.6536e-6*cos(th1(t)) + 1.0*sin(th1(t))) - 1.3268e-6*sin(th2(t) - 1.5708)*cos(th1(t)))) + 0.38*sin(th3(t))*(1.0*cos(th2(t) - 1.5708)*(2.6536e-6*cos(th1(t)) + 1.0*sin(th1(t))) - 1.3268e-6*sin(th2(t) - 1.5708)*cos(th1(t))) - 0.02*cos(th5(t))*(sin(th4(t) - 3.1416)*(sin(th3(t) - 1.5708)*(sin(th2(t) - 1.5708)*(2.6536e-6*cos(th1(t)) + 1.0*sin(th1(t))) + 1.3268e-6*cos(th2(t) - 1.5708)*cos(th1(t))) - cos(th3(t) - 1.5708)*(1.0*cos(th2(t) - 1.5708)*(2.6536e-6*cos(th1(t)) + 1.0*sin(th1(t))) - 1.3268e-6*sin(th2(t) - 1.5708)*cos(th1(t)))) + cos(th4(t) - 3.1416)*(cos(th3(t) - 1.5708)*(sin(th2(t) - 1.5708)*(2.6536e-6*cos(th1(t)) + 1.0*sin(th1(t))) + 1.3268e-6*cos(th2(t) - 1.5708)*cos(th1(t))) + 1.0*sin(th3(t) - 1.5708)*(1.0*cos(th2(t) - 1.5708)*(2.6536e-6*cos(th1(t)) + 1.0*sin(th1(t))) - 1.3268e-6*sin(th2(t) - 1.5708)*cos(th1(t))))) + 0.38*cos(th4(t))*(cos(th3(t) - 1.5708)*(sin(th2(t) - 1.5708)*(2.6536e-6*cos(th1(t)) + 1.0*sin(th1(t))) + 1.3268e-6*cos(th2(t) - 1.5708)*cos(th1(t))) + 1.0*sin(th3(t) - 1.5708)*(1.0*cos(th2(t) - 1.5708)*(2.6536e-6*cos(th1(t)) + 1.0*sin(th1(t))) - 1.3268e-6*sin(th2(t) - 1.5708)*cos(th1(t)))) + 0.02*sin(th5(t))*(cos(th4(t) - 3.1416)*(sin(th3(t) - 1.5708)*(sin(th2(t) - 1.5708)*(2.6536e-6*cos(th1(t)) + 1.0*sin(th1(t))) + 1.3268e-6*cos(th2(t) - 1.5708)*cos(th1(t))) - cos(th3(t) - 1.5708)*(1.0*cos(th2(t) - 1.5708)*(2.6536e-6*cos(th1(t)) + 1.0*sin(th1(t))) - 1.3268e-6*sin(th2(t) - 1.5708)*cos(th1(t)))) - 1.0*sin(th4(t) - 3.1416)*(cos(th3(t) - 1.5708)*(sin(th2(t) - 1.5708)*(2.6536e-6*cos(th1(t)) + 1.0*sin(th1(t))) + 1.3268e-6*cos(th2(t) - 1.5708)*cos(th1(t))) + 1.0*sin(th3(t) - 1.5708)*(1.0*cos(th2(t) - 1.5708)*(2.6536e-6*cos(th1(t)) + 1.0*sin(th1(t))) - 1.3268e-6*sin(th2(t) - 1.5708)*cos(th1(t)))))) + 1.3806*(0.19*cos(th4(t))*(cos(th3(t) - 1.5708)*(sin(th2(t) - 1.5708)*(1.0*cos(th1(t)) - 2.6536e-6*sin(th1(t))) - 1.3268e-6*cos(th2(t) - 1.5708)*sin(th1(t))) + sin(th3(t) - 1.5708)*(cos(th2(t) - 1.5708)*(1.0*cos(th1(t)) - 2.6536e-6*sin(th1(t))) + 1.3268e-6*sin(th2(t) - 1.5708)*sin(th1(t)))) + 0.19*sin(th4(t))*(cos(th3(t) - 1.5708)*(cos(th2(t) - 1.5708)*(1.0*cos(th1(t)) - 2.6536e-6*sin(th1(t))) + 1.3268e-6*sin(th2(t) - 1.5708)*sin(th1(t))) - 1.0*sin(th3(t) - 1.5708)*(sin(th2(t) - 1.5708)*(1.0*cos(th1(t)) - 2.6536e-6*sin(th1(t))) - 1.3268e-6*cos(th2(t) - 1.5708)*sin(th1(t)))))*(0.19*cos(th4(t))*(cos(th3(t) - 1.5708)*(sin(th2(t) - 1.5708)*(1.0*cos(th1(t)) - 2.6536e-6*sin(th1(t))) - 1.3268e-6*cos(th2(t) - 1.5708)*sin(th1(t))) + sin(th3(t) - 1.5708)*(cos(th2(t) - 1.5708)*(1.0*cos(th1(t)) - 2.6536e-6*sin(th1(t))) + 1.3268e-6*sin(th2(t) - 1.5708)*sin(th1(t)))) + 0.38*cos(th3(t))*(sin(th2(t) - 1.5708)*(1.0*cos(th1(t)) - 2.6536e-6*sin(th1(t))) - 1.3268e-6*cos(th2(t) - 1.5708)*sin(th1(t))) + 0.38*sin(th3(t))*(cos(th2(t) - 1.5708)*(1.0*cos(th1(t)) - 2.6536e-6*sin(th1(t))) + 1.3268e-6*sin(th2(t) - 1.5708)*sin(th1(t))) + 0.19*sin(th4(t))*(cos(th3(t) - 1.5708)*(cos(th2(t) - 1.5708)*(1.0*cos(th1(t)) - 2.6536e-6*sin(th1(t))) + 1.3268e-6*sin(th2(t) - 1.5708)*sin(th1(t))) - 1.0*sin(th3(t) - 1.5708)*(sin(th2(t) - 1.5708)*(1.0*cos(th1(t)) - 2.6536e-6*sin(th1(t))) - 1.3268e-6*cos(th2(t) - 1.5708)*sin(th1(t))))) + 0.13038*(0.38*cos(th4(t))*(cos(th3(t) - 1.5708)*(sin(th2(t) - 1.5708)*(1.0*cos(th1(t)) - 2.6536e-6*sin(th1(t))) - 1.3268e-6*cos(th2(t) - 1.5708)*sin(th1(t))) + sin(th3(t) - 1.5708)*(cos(th2(t) - 1.5708)*(1.0*cos(th1(t)) - 2.6536e-6*sin(th1(t))) + 1.3268e-6*sin(th2(t) - 1.5708)*sin(th1(t)))) + 0.02*sin(th5(t))*(sin(th4(t) - 3.1416)*(cos(th3(t) - 1.5708)*(sin(th2(t) - 1.5708)*(1.0*cos(th1(t)) - 2.6536e-6*sin(th1(t))) - 1.3268e-6*cos(th2(t) - 1.5708)*sin(th1(t))) + sin(th3(t) - 1.5708)*(cos(th2(t) - 1.5708)*(1.0*cos(th1(t)) - 2.6536e-6*sin(th1(t))) + 1.3268e-6*sin(th2(t) - 1.5708)*sin(th1(t)))) + cos(th4(t) - 3.1416)*(cos(th3(t) - 1.5708)*(cos(th2(t) - 1.5708)*(1.0*cos(th1(t)) - 2.6536e-6*sin(th1(t))) + 1.3268e-6*sin(th2(t) - 1.5708)*sin(th1(t))) - 1.0*sin(th3(t) - 1.5708)*(sin(th2(t) - 1.5708)*(1.0*cos(th1(t)) - 2.6536e-6*sin(th1(t))) - 1.3268e-6*cos(th2(t) - 1.5708)*sin(th1(t))))) + 0.38*sin(th4(t))*(cos(th3(t) - 1.5708)*(cos(th2(t) - 1.5708)*(1.0*cos(th1(t)) - 2.6536e-6*sin(th1(t))) + 1.3268e-6*sin(th2(t) - 1.5708)*sin(th1(t))) - 1.0*sin(th3(t) - 1.5708)*(sin(th2(t) - 1.5708)*(1.0*cos(th1(t)) - 2.6536e-6*sin(th1(t))) - 1.3268e-6*cos(th2(t) - 1.5708)*sin(th1(t)))) + 0.02*cos(th5(t))*(cos(th4(t) - 3.1416)*(cos(th3(t) - 1.5708)*(sin(th2(t) - 1.5708)*(1.0*cos(th1(t)) - 2.6536e-6*sin(th1(t))) - 1.3268e-6*cos(th2(t) - 1.5708)*sin(th1(t))) + sin(th3(t) - 1.5708)*(cos(th2(t) - 1.5708)*(1.0*cos(th1(t)) - 2.6536e-6*sin(th1(t))) + 1.3268e-6*sin(th2(t) - 1.5708)*sin(th1(t)))) - 1.0*sin(th4(t) - 3.1416)*(cos(th3(t) - 1.5708)*(cos(th2(t) - 1.5708)*(1.0*cos(th1(t)) - 2.6536e-6*sin(th1(t))) + 1.3268e-6*sin(th2(t) - 1.5708)*sin(th1(t))) - 1.0*sin(th3(t) - 1.5708)*(sin(th2(t) - 1.5708)*(1.0*cos(th1(t)) - 2.6536e-6*sin(th1(t))) - 1.3268e-6*cos(th2(t) - 1.5708)*sin(th1(t))))))*(0.38*cos(th4(t))*(cos(th3(t) - 1.5708)*(sin(th2(t) - 1.5708)*(1.0*cos(th1(t)) - 2.6536e-6*sin(th1(t))) - 1.3268e-6*cos(th2(t) - 1.5708)*sin(th1(t))) + sin(th3(t) - 1.5708)*(cos(th2(t) - 1.5708)*(1.0*cos(th1(t)) - 2.6536e-6*sin(th1(t))) + 1.3268e-6*sin(th2(t) - 1.5708)*sin(th1(t)))) + 0.38*cos(th3(t))*(sin(th2(t) - 1.5708)*(1.0*cos(th1(t)) - 2.6536e-6*sin(th1(t))) - 1.3268e-6*cos(th2(t) - 1.5708)*sin(th1(t))) + 0.38*sin(th3(t))*(cos(th2(t) - 1.5708)*(1.0*cos(th1(t)) - 2.6536e-6*sin(th1(t))) + 1.3268e-6*sin(th2(t) - 1.5708)*sin(th1(t))) - 0.02*sin(th5(t))*(sin(th4(t) - 3.1416)*(cos(th3(t) - 1.5708)*(sin(th2(t) - 1.5708)*(1.0*cos(th1(t)) - 2.6536e-6*sin(th1(t))) - 1.3268e-6*cos(th2(t) - 1.5708)*sin(th1(t))) + sin(th3(t) - 1.5708)*(cos(th2(t) - 1.5708)*(1.0*cos(th1(t)) - 2.6536e-6*sin(th1(t))) + 1.3268e-6*sin(th2(t) - 1.5708)*sin(th1(t)))) + cos(th4(t) - 3.1416)*(cos(th3(t) - 1.5708)*(cos(th2(t) - 1.5708)*(1.0*cos(th1(t)) - 2.6536e-6*sin(th1(t))) + 1.3268e-6*sin(th2(t) - 1.5708)*sin(th1(t))) - 1.0*sin(th3(t) - 1.5708)*(sin(th2(t) - 1.5708)*(1.0*cos(th1(t)) - 2.6536e-6*sin(th1(t))) - 1.3268e-6*cos(th2(t) - 1.5708)*sin(th1(t))))) + 0.38*sin(th4(t))*(cos(th3(t) - 1.5708)*(cos(th2(t) - 1.5708)*(1.0*cos(th1(t)) - 2.6536e-6*sin(th1(t))) + 1.3268e-6*sin(th2(t) - 1.5708)*sin(th1(t))) - 1.0*sin(th3(t) - 1.5708)*(sin(th2(t) - 1.5708)*(1.0*cos(th1(t)) - 2.6536e-6*sin(th1(t))) - 1.3268e-6*cos(th2(t) - 1.5708)*sin(th1(t)))) - 0.02*cos(th5(t))*(cos(th4(t) - 3.1416)*(cos(th3(t) - 1.5708)*(sin(th2(t) - 1.5708)*(1.0*cos(th1(t)) - 2.6536e-6*sin(th1(t))) - 1.3268e-6*cos(th2(t) - 1.5708)*sin(th1(t))) + sin(th3(t) - 1.5708)*(cos(th2(t) - 1.5708)*(1.0*cos(th1(t)) - 2.6536e-6*sin(th1(t))) + 1.3268e-6*sin(th2(t) - 1.5708)*sin(th1(t)))) - 1.0*sin(th4(t) - 3.1416)*(cos(th3(t) - 1.5708)*(cos(th2(t) - 1.5708)*(1.0*cos(th1(t)) - 2.6536e-6*sin(th1(t))) + 1.3268e-6*sin(th2(t) - 1.5708)*sin(th1(t))) - 1.0*sin(th3(t) - 1.5708)*(sin(th2(t) - 1.5708)*(1.0*cos(th1(t)) - 2.6536e-6*sin(th1(t))) - 1.3268e-6*cos(th2(t) - 1.5708)*sin(th1(t)))))) + 0.042427;
M44 = 1.3806*(0.19*cos(th4(t))*(cos(th3(t) - 1.5708)*(sin(th2(t) - 1.5708)*(1.0*cos(th1(t)) - 2.6536e-6*sin(th1(t))) - 1.3268e-6*cos(th2(t) - 1.5708)*sin(th1(t))) + sin(th3(t) - 1.5708)*(cos(th2(t) - 1.5708)*(1.0*cos(th1(t)) - 2.6536e-6*sin(th1(t))) + 1.3268e-6*sin(th2(t) - 1.5708)*sin(th1(t)))) + 0.19*sin(th4(t))*(cos(th3(t) - 1.5708)*(cos(th2(t) - 1.5708)*(1.0*cos(th1(t)) - 2.6536e-6*sin(th1(t))) + 1.3268e-6*sin(th2(t) - 1.5708)*sin(th1(t))) - 1.0*sin(th3(t) - 1.5708)*(sin(th2(t) - 1.5708)*(1.0*cos(th1(t)) - 2.6536e-6*sin(th1(t))) - 1.3268e-6*cos(th2(t) - 1.5708)*sin(th1(t)))))^2 + 1.3806*(0.19*sin(th4(t))*(sin(th3(t) - 1.5708)*(sin(th2(t) - 1.5708)*(2.6536e-6*cos(th1(t)) + 1.0*sin(th1(t))) + 1.3268e-6*cos(th2(t) - 1.5708)*cos(th1(t))) - cos(th3(t) - 1.5708)*(1.0*cos(th2(t) - 1.5708)*(2.6536e-6*cos(th1(t)) + 1.0*sin(th1(t))) - 1.3268e-6*sin(th2(t) - 1.5708)*cos(th1(t)))) - 0.19*cos(th4(t))*(cos(th3(t) - 1.5708)*(sin(th2(t) - 1.5708)*(2.6536e-6*cos(th1(t)) + 1.0*sin(th1(t))) + 1.3268e-6*cos(th2(t) - 1.5708)*cos(th1(t))) + 1.0*sin(th3(t) - 1.5708)*(1.0*cos(th2(t) - 1.5708)*(2.6536e-6*cos(th1(t)) + 1.0*sin(th1(t))) - 1.3268e-6*sin(th2(t) - 1.5708)*cos(th1(t)))))^2 + 0.13038*(0.38*sin(th4(t))*(sin(th3(t) - 1.5708)*(sin(th2(t) - 1.5708)*(2.6536e-6*cos(th1(t)) + 1.0*sin(th1(t))) + 1.3268e-6*cos(th2(t) - 1.5708)*cos(th1(t))) - cos(th3(t) - 1.5708)*(1.0*cos(th2(t) - 1.5708)*(2.6536e-6*cos(th1(t)) + 1.0*sin(th1(t))) - 1.3268e-6*sin(th2(t) - 1.5708)*cos(th1(t)))) - 0.02*cos(th5(t))*(sin(th4(t) - 3.1416)*(sin(th3(t) - 1.5708)*(sin(th2(t) - 1.5708)*(2.6536e-6*cos(th1(t)) + 1.0*sin(th1(t))) + 1.3268e-6*cos(th2(t) - 1.5708)*cos(th1(t))) - cos(th3(t) - 1.5708)*(1.0*cos(th2(t) - 1.5708)*(2.6536e-6*cos(th1(t)) + 1.0*sin(th1(t))) - 1.3268e-6*sin(th2(t) - 1.5708)*cos(th1(t)))) + cos(th4(t) - 3.1416)*(cos(th3(t) - 1.5708)*(sin(th2(t) - 1.5708)*(2.6536e-6*cos(th1(t)) + 1.0*sin(th1(t))) + 1.3268e-6*cos(th2(t) - 1.5708)*cos(th1(t))) + 1.0*sin(th3(t) - 1.5708)*(1.0*cos(th2(t) - 1.5708)*(2.6536e-6*cos(th1(t)) + 1.0*sin(th1(t))) - 1.3268e-6*sin(th2(t) - 1.5708)*cos(th1(t))))) - 0.38*cos(th4(t))*(cos(th3(t) - 1.5708)*(sin(th2(t) - 1.5708)*(2.6536e-6*cos(th1(t)) + 1.0*sin(th1(t))) + 1.3268e-6*cos(th2(t) - 1.5708)*cos(th1(t))) + 1.0*sin(th3(t) - 1.5708)*(1.0*cos(th2(t) - 1.5708)*(2.6536e-6*cos(th1(t)) + 1.0*sin(th1(t))) - 1.3268e-6*sin(th2(t) - 1.5708)*cos(th1(t)))) + 0.02*sin(th5(t))*(cos(th4(t) - 3.1416)*(sin(th3(t) - 1.5708)*(sin(th2(t) - 1.5708)*(2.6536e-6*cos(th1(t)) + 1.0*sin(th1(t))) + 1.3268e-6*cos(th2(t) - 1.5708)*cos(th1(t))) - cos(th3(t) - 1.5708)*(1.0*cos(th2(t) - 1.5708)*(2.6536e-6*cos(th1(t)) + 1.0*sin(th1(t))) - 1.3268e-6*sin(th2(t) - 1.5708)*cos(th1(t)))) - 1.0*sin(th4(t) - 3.1416)*(cos(th3(t) - 1.5708)*(sin(th2(t) - 1.5708)*(2.6536e-6*cos(th1(t)) + 1.0*sin(th1(t))) + 1.3268e-6*cos(th2(t) - 1.5708)*cos(th1(t))) + 1.0*sin(th3(t) - 1.5708)*(1.0*cos(th2(t) - 1.5708)*(2.6536e-6*cos(th1(t)) + 1.0*sin(th1(t))) - 1.3268e-6*sin(th2(t) - 1.5708)*cos(th1(t))))))^2 + 0.13038*(0.02*sin(th5(t))*(cos(th4(t) - 3.1416)*(cos(th3(t) - 1.5708)*(3.5208e-12*cos(th2(t) - 1.5708) + 1.0*sin(th2(t) - 1.5708)) + sin(th3(t) - 1.5708)*(1.0*cos(th2(t) - 1.5708) - 3.5208e-12*sin(th2(t) - 1.5708))) - 1.0*sin(th4(t) - 3.1416)*(cos(th3(t) - 1.5708)*(1.0*cos(th2(t) - 1.5708) - 3.5208e-12*sin(th2(t) - 1.5708)) - 1.0*sin(th3(t) - 1.5708)*(3.5208e-12*cos(th2(t) - 1.5708) + 1.0*sin(th2(t) - 1.5708)))) + 0.38*sin(th4(t))*(cos(th3(t) - 1.5708)*(3.5208e-12*cos(th2(t) - 1.5708) + 1.0*sin(th2(t) - 1.5708)) + sin(th3(t) - 1.5708)*(1.0*cos(th2(t) - 1.5708) - 3.5208e-12*sin(th2(t) - 1.5708))) - 0.38*cos(th4(t))*(cos(th3(t) - 1.5708)*(1.0*cos(th2(t) - 1.5708) - 3.5208e-12*sin(th2(t) - 1.5708)) - 1.0*sin(th3(t) - 1.5708)*(3.5208e-12*cos(th2(t) - 1.5708) + 1.0*sin(th2(t) - 1.5708))) - 0.02*cos(th5(t))*(sin(th4(t) - 3.1416)*(cos(th3(t) - 1.5708)*(3.5208e-12*cos(th2(t) - 1.5708) + 1.0*sin(th2(t) - 1.5708)) + sin(th3(t) - 1.5708)*(1.0*cos(th2(t) - 1.5708) - 3.5208e-12*sin(th2(t) - 1.5708))) + cos(th4(t) - 3.1416)*(cos(th3(t) - 1.5708)*(1.0*cos(th2(t) - 1.5708) - 3.5208e-12*sin(th2(t) - 1.5708)) - 1.0*sin(th3(t) - 1.5708)*(3.5208e-12*cos(th2(t) - 1.5708) + 1.0*sin(th2(t) - 1.5708)))))^2 + 1.3806*(0.19*sin(th4(t))*(cos(th3(t) - 1.5708)*(3.5208e-12*cos(th2(t) - 1.5708) + 1.0*sin(th2(t) - 1.5708)) + sin(th3(t) - 1.5708)*(1.0*cos(th2(t) - 1.5708) - 3.5208e-12*sin(th2(t) - 1.5708))) - 0.19*cos(th4(t))*(cos(th3(t) - 1.5708)*(1.0*cos(th2(t) - 1.5708) - 3.5208e-12*sin(th2(t) - 1.5708)) - 1.0*sin(th3(t) - 1.5708)*(3.5208e-12*cos(th2(t) - 1.5708) + 1.0*sin(th2(t) - 1.5708))))^2 + 0.13038*(0.38*cos(th4(t))*(cos(th3(t) - 1.5708)*(sin(th2(t) - 1.5708)*(1.0*cos(th1(t)) - 2.6536e-6*sin(th1(t))) - 1.3268e-6*cos(th2(t) - 1.5708)*sin(th1(t))) + sin(th3(t) - 1.5708)*(cos(th2(t) - 1.5708)*(1.0*cos(th1(t)) - 2.6536e-6*sin(th1(t))) + 1.3268e-6*sin(th2(t) - 1.5708)*sin(th1(t)))) + 0.02*sin(th5(t))*(sin(th4(t) - 3.1416)*(cos(th3(t) - 1.5708)*(sin(th2(t) - 1.5708)*(1.0*cos(th1(t)) - 2.6536e-6*sin(th1(t))) - 1.3268e-6*cos(th2(t) - 1.5708)*sin(th1(t))) + sin(th3(t) - 1.5708)*(cos(th2(t) - 1.5708)*(1.0*cos(th1(t)) - 2.6536e-6*sin(th1(t))) + 1.3268e-6*sin(th2(t) - 1.5708)*sin(th1(t)))) + cos(th4(t) - 3.1416)*(cos(th3(t) - 1.5708)*(cos(th2(t) - 1.5708)*(1.0*cos(th1(t)) - 2.6536e-6*sin(th1(t))) + 1.3268e-6*sin(th2(t) - 1.5708)*sin(th1(t))) - 1.0*sin(th3(t) - 1.5708)*(sin(th2(t) - 1.5708)*(1.0*cos(th1(t)) - 2.6536e-6*sin(th1(t))) - 1.3268e-6*cos(th2(t) - 1.5708)*sin(th1(t))))) + 0.38*sin(th4(t))*(cos(th3(t) - 1.5708)*(cos(th2(t) - 1.5708)*(1.0*cos(th1(t)) - 2.6536e-6*sin(th1(t))) + 1.3268e-6*sin(th2(t) - 1.5708)*sin(th1(t))) - 1.0*sin(th3(t) - 1.5708)*(sin(th2(t) - 1.5708)*(1.0*cos(th1(t)) - 2.6536e-6*sin(th1(t))) - 1.3268e-6*cos(th2(t) - 1.5708)*sin(th1(t)))) + 0.02*cos(th5(t))*(cos(th4(t) - 3.1416)*(cos(th3(t) - 1.5708)*(sin(th2(t) - 1.5708)*(1.0*cos(th1(t)) - 2.6536e-6*sin(th1(t))) - 1.3268e-6*cos(th2(t) - 1.5708)*sin(th1(t))) + sin(th3(t) - 1.5708)*(cos(th2(t) - 1.5708)*(1.0*cos(th1(t)) - 2.6536e-6*sin(th1(t))) + 1.3268e-6*sin(th2(t) - 1.5708)*sin(th1(t)))) - 1.0*sin(th4(t) - 3.1416)*(cos(th3(t) - 1.5708)*(cos(th2(t) - 1.5708)*(1.0*cos(th1(t)) - 2.6536e-6*sin(th1(t))) + 1.3268e-6*sin(th2(t) - 1.5708)*sin(th1(t))) - 1.0*sin(th3(t) - 1.5708)*(sin(th2(t) - 1.5708)*(1.0*cos(th1(t)) - 2.6536e-6*sin(th1(t))) - 1.3268e-6*cos(th2(t) - 1.5708)*sin(th1(t))))))^2 + 0.042427;
M45 = 0.13038*(0.02*cos(th5(t))*(sin(th4(t) - 3.1416)*(sin(th3(t) - 1.5708)*(sin(th2(t) - 1.5708)*(2.6536e-6*cos(th1(t)) + 1.0*sin(th1(t))) + 1.3268e-6*cos(th2(t) - 1.5708)*cos(th1(t))) - cos(th3(t) - 1.5708)*(1.0*cos(th2(t) - 1.5708)*(2.6536e-6*cos(th1(t)) + 1.0*sin(th1(t))) - 1.3268e-6*sin(th2(t) - 1.5708)*cos(th1(t)))) + cos(th4(t) - 3.1416)*(cos(th3(t) - 1.5708)*(sin(th2(t) - 1.5708)*(2.6536e-6*cos(th1(t)) + 1.0*sin(th1(t))) + 1.3268e-6*cos(th2(t) - 1.5708)*cos(th1(t))) + 1.0*sin(th3(t) - 1.5708)*(1.0*cos(th2(t) - 1.5708)*(2.6536e-6*cos(th1(t)) + 1.0*sin(th1(t))) - 1.3268e-6*sin(th2(t) - 1.5708)*cos(th1(t))))) - 0.02*sin(th5(t))*(cos(th4(t) - 3.1416)*(sin(th3(t) - 1.5708)*(sin(th2(t) - 1.5708)*(2.6536e-6*cos(th1(t)) + 1.0*sin(th1(t))) + 1.3268e-6*cos(th2(t) - 1.5708)*cos(th1(t))) - cos(th3(t) - 1.5708)*(1.0*cos(th2(t) - 1.5708)*(2.6536e-6*cos(th1(t)) + 1.0*sin(th1(t))) - 1.3268e-6*sin(th2(t) - 1.5708)*cos(th1(t)))) - 1.0*sin(th4(t) - 3.1416)*(cos(th3(t) - 1.5708)*(sin(th2(t) - 1.5708)*(2.6536e-6*cos(th1(t)) + 1.0*sin(th1(t))) + 1.3268e-6*cos(th2(t) - 1.5708)*cos(th1(t))) + 1.0*sin(th3(t) - 1.5708)*(1.0*cos(th2(t) - 1.5708)*(2.6536e-6*cos(th1(t)) + 1.0*sin(th1(t))) - 1.3268e-6*sin(th2(t) - 1.5708)*cos(th1(t))))))*(0.38*sin(th4(t))*(sin(th3(t) - 1.5708)*(sin(th2(t) - 1.5708)*(2.6536e-6*cos(th1(t)) + 1.0*sin(th1(t))) + 1.3268e-6*cos(th2(t) - 1.5708)*cos(th1(t))) - cos(th3(t) - 1.5708)*(1.0*cos(th2(t) - 1.5708)*(2.6536e-6*cos(th1(t)) + 1.0*sin(th1(t))) - 1.3268e-6*sin(th2(t) - 1.5708)*cos(th1(t)))) - 0.02*cos(th5(t))*(sin(th4(t) - 3.1416)*(sin(th3(t) - 1.5708)*(sin(th2(t) - 1.5708)*(2.6536e-6*cos(th1(t)) + 1.0*sin(th1(t))) + 1.3268e-6*cos(th2(t) - 1.5708)*cos(th1(t))) - cos(th3(t) - 1.5708)*(1.0*cos(th2(t) - 1.5708)*(2.6536e-6*cos(th1(t)) + 1.0*sin(th1(t))) - 1.3268e-6*sin(th2(t) - 1.5708)*cos(th1(t)))) + cos(th4(t) - 3.1416)*(cos(th3(t) - 1.5708)*(sin(th2(t) - 1.5708)*(2.6536e-6*cos(th1(t)) + 1.0*sin(th1(t))) + 1.3268e-6*cos(th2(t) - 1.5708)*cos(th1(t))) + 1.0*sin(th3(t) - 1.5708)*(1.0*cos(th2(t) - 1.5708)*(2.6536e-6*cos(th1(t)) + 1.0*sin(th1(t))) - 1.3268e-6*sin(th2(t) - 1.5708)*cos(th1(t))))) - 0.38*cos(th4(t))*(cos(th3(t) - 1.5708)*(sin(th2(t) - 1.5708)*(2.6536e-6*cos(th1(t)) + 1.0*sin(th1(t))) + 1.3268e-6*cos(th2(t) - 1.5708)*cos(th1(t))) + 1.0*sin(th3(t) - 1.5708)*(1.0*cos(th2(t) - 1.5708)*(2.6536e-6*cos(th1(t)) + 1.0*sin(th1(t))) - 1.3268e-6*sin(th2(t) - 1.5708)*cos(th1(t)))) + 0.02*sin(th5(t))*(cos(th4(t) - 3.1416)*(sin(th3(t) - 1.5708)*(sin(th2(t) - 1.5708)*(2.6536e-6*cos(th1(t)) + 1.0*sin(th1(t))) + 1.3268e-6*cos(th2(t) - 1.5708)*cos(th1(t))) - cos(th3(t) - 1.5708)*(1.0*cos(th2(t) - 1.5708)*(2.6536e-6*cos(th1(t)) + 1.0*sin(th1(t))) - 1.3268e-6*sin(th2(t) - 1.5708)*cos(th1(t)))) - 1.0*sin(th4(t) - 3.1416)*(cos(th3(t) - 1.5708)*(sin(th2(t) - 1.5708)*(2.6536e-6*cos(th1(t)) + 1.0*sin(th1(t))) + 1.3268e-6*cos(th2(t) - 1.5708)*cos(th1(t))) + 1.0*sin(th3(t) - 1.5708)*(1.0*cos(th2(t) - 1.5708)*(2.6536e-6*cos(th1(t)) + 1.0*sin(th1(t))) - 1.3268e-6*sin(th2(t) - 1.5708)*cos(th1(t)))))) - 0.13038*(0.02*sin(th5(t))*(cos(th4(t) - 3.1416)*(cos(th3(t) - 1.5708)*(3.5208e-12*cos(th2(t) - 1.5708) + 1.0*sin(th2(t) - 1.5708)) + sin(th3(t) - 1.5708)*(1.0*cos(th2(t) - 1.5708) - 3.5208e-12*sin(th2(t) - 1.5708))) - 1.0*sin(th4(t) - 3.1416)*(cos(th3(t) - 1.5708)*(1.0*cos(th2(t) - 1.5708) - 3.5208e-12*sin(th2(t) - 1.5708)) - 1.0*sin(th3(t) - 1.5708)*(3.5208e-12*cos(th2(t) - 1.5708) + 1.0*sin(th2(t) - 1.5708)))) - 0.02*cos(th5(t))*(sin(th4(t) - 3.1416)*(cos(th3(t) - 1.5708)*(3.5208e-12*cos(th2(t) - 1.5708) + 1.0*sin(th2(t) - 1.5708)) + sin(th3(t) - 1.5708)*(1.0*cos(th2(t) - 1.5708) - 3.5208e-12*sin(th2(t) - 1.5708))) + cos(th4(t) - 3.1416)*(cos(th3(t) - 1.5708)*(1.0*cos(th2(t) - 1.5708) - 3.5208e-12*sin(th2(t) - 1.5708)) - 1.0*sin(th3(t) - 1.5708)*(3.5208e-12*cos(th2(t) - 1.5708) + 1.0*sin(th2(t) - 1.5708)))))*(0.02*sin(th5(t))*(cos(th4(t) - 3.1416)*(cos(th3(t) - 1.5708)*(3.5208e-12*cos(th2(t) - 1.5708) + 1.0*sin(th2(t) - 1.5708)) + sin(th3(t) - 1.5708)*(1.0*cos(th2(t) - 1.5708) - 3.5208e-12*sin(th2(t) - 1.5708))) - 1.0*sin(th4(t) - 3.1416)*(cos(th3(t) - 1.5708)*(1.0*cos(th2(t) - 1.5708) - 3.5208e-12*sin(th2(t) - 1.5708)) - 1.0*sin(th3(t) - 1.5708)*(3.5208e-12*cos(th2(t) - 1.5708) + 1.0*sin(th2(t) - 1.5708)))) + 0.38*sin(th4(t))*(cos(th3(t) - 1.5708)*(3.5208e-12*cos(th2(t) - 1.5708) + 1.0*sin(th2(t) - 1.5708)) + sin(th3(t) - 1.5708)*(1.0*cos(th2(t) - 1.5708) - 3.5208e-12*sin(th2(t) - 1.5708))) - 0.38*cos(th4(t))*(cos(th3(t) - 1.5708)*(1.0*cos(th2(t) - 1.5708) - 3.5208e-12*sin(th2(t) - 1.5708)) - 1.0*sin(th3(t) - 1.5708)*(3.5208e-12*cos(th2(t) - 1.5708) + 1.0*sin(th2(t) - 1.5708))) - 0.02*cos(th5(t))*(sin(th4(t) - 3.1416)*(cos(th3(t) - 1.5708)*(3.5208e-12*cos(th2(t) - 1.5708) + 1.0*sin(th2(t) - 1.5708)) + sin(th3(t) - 1.5708)*(1.0*cos(th2(t) - 1.5708) - 3.5208e-12*sin(th2(t) - 1.5708))) + cos(th4(t) - 3.1416)*(cos(th3(t) - 1.5708)*(1.0*cos(th2(t) - 1.5708) - 3.5208e-12*sin(th2(t) - 1.5708)) - 1.0*sin(th3(t) - 1.5708)*(3.5208e-12*cos(th2(t) - 1.5708) + 1.0*sin(th2(t) - 1.5708))))) - 0.13038*(0.02*sin(th5(t))*(sin(th4(t) - 3.1416)*(cos(th3(t) - 1.5708)*(sin(th2(t) - 1.5708)*(1.0*cos(th1(t)) - 2.6536e-6*sin(th1(t))) - 1.3268e-6*cos(th2(t) - 1.5708)*sin(th1(t))) + sin(th3(t) - 1.5708)*(cos(th2(t) - 1.5708)*(1.0*cos(th1(t)) - 2.6536e-6*sin(th1(t))) + 1.3268e-6*sin(th2(t) - 1.5708)*sin(th1(t)))) + cos(th4(t) - 3.1416)*(cos(th3(t) - 1.5708)*(cos(th2(t) - 1.5708)*(1.0*cos(th1(t)) - 2.6536e-6*sin(th1(t))) + 1.3268e-6*sin(th2(t) - 1.5708)*sin(th1(t))) - 1.0*sin(th3(t) - 1.5708)*(sin(th2(t) - 1.5708)*(1.0*cos(th1(t)) - 2.6536e-6*sin(th1(t))) - 1.3268e-6*cos(th2(t) - 1.5708)*sin(th1(t))))) + 0.02*cos(th5(t))*(cos(th4(t) - 3.1416)*(cos(th3(t) - 1.5708)*(sin(th2(t) - 1.5708)*(1.0*cos(th1(t)) - 2.6536e-6*sin(th1(t))) - 1.3268e-6*cos(th2(t) - 1.5708)*sin(th1(t))) + sin(th3(t) - 1.5708)*(cos(th2(t) - 1.5708)*(1.0*cos(th1(t)) - 2.6536e-6*sin(th1(t))) + 1.3268e-6*sin(th2(t) - 1.5708)*sin(th1(t)))) - 1.0*sin(th4(t) - 3.1416)*(cos(th3(t) - 1.5708)*(cos(th2(t) - 1.5708)*(1.0*cos(th1(t)) - 2.6536e-6*sin(th1(t))) + 1.3268e-6*sin(th2(t) - 1.5708)*sin(th1(t))) - 1.0*sin(th3(t) - 1.5708)*(sin(th2(t) - 1.5708)*(1.0*cos(th1(t)) - 2.6536e-6*sin(th1(t))) - 1.3268e-6*cos(th2(t) - 1.5708)*sin(th1(t))))))*(0.38*cos(th4(t))*(cos(th3(t) - 1.5708)*(sin(th2(t) - 1.5708)*(1.0*cos(th1(t)) - 2.6536e-6*sin(th1(t))) - 1.3268e-6*cos(th2(t) - 1.5708)*sin(th1(t))) + sin(th3(t) - 1.5708)*(cos(th2(t) - 1.5708)*(1.0*cos(th1(t)) - 2.6536e-6*sin(th1(t))) + 1.3268e-6*sin(th2(t) - 1.5708)*sin(th1(t)))) + 0.02*sin(th5(t))*(sin(th4(t) - 3.1416)*(cos(th3(t) - 1.5708)*(sin(th2(t) - 1.5708)*(1.0*cos(th1(t)) - 2.6536e-6*sin(th1(t))) - 1.3268e-6*cos(th2(t) - 1.5708)*sin(th1(t))) + sin(th3(t) - 1.5708)*(cos(th2(t) - 1.5708)*(1.0*cos(th1(t)) - 2.6536e-6*sin(th1(t))) + 1.3268e-6*sin(th2(t) - 1.5708)*sin(th1(t)))) + cos(th4(t) - 3.1416)*(cos(th3(t) - 1.5708)*(cos(th2(t) - 1.5708)*(1.0*cos(th1(t)) - 2.6536e-6*sin(th1(t))) + 1.3268e-6*sin(th2(t) - 1.5708)*sin(th1(t))) - 1.0*sin(th3(t) - 1.5708)*(sin(th2(t) - 1.5708)*(1.0*cos(th1(t)) - 2.6536e-6*sin(th1(t))) - 1.3268e-6*cos(th2(t) - 1.5708)*sin(th1(t))))) + 0.38*sin(th4(t))*(cos(th3(t) - 1.5708)*(cos(th2(t) - 1.5708)*(1.0*cos(th1(t)) - 2.6536e-6*sin(th1(t))) + 1.3268e-6*sin(th2(t) - 1.5708)*sin(th1(t))) - 1.0*sin(th3(t) - 1.5708)*(sin(th2(t) - 1.5708)*(1.0*cos(th1(t)) - 2.6536e-6*sin(th1(t))) - 1.3268e-6*cos(th2(t) - 1.5708)*sin(th1(t)))) + 0.02*cos(th5(t))*(cos(th4(t) - 3.1416)*(cos(th3(t) - 1.5708)*(sin(th2(t) - 1.5708)*(1.0*cos(th1(t)) - 2.6536e-6*sin(th1(t))) - 1.3268e-6*cos(th2(t) - 1.5708)*sin(th1(t))) + sin(th3(t) - 1.5708)*(cos(th2(t) - 1.5708)*(1.0*cos(th1(t)) - 2.6536e-6*sin(th1(t))) + 1.3268e-6*sin(th2(t) - 1.5708)*sin(th1(t)))) - 1.0*sin(th4(t) - 3.1416)*(cos(th3(t) - 1.5708)*(cos(th2(t) - 1.5708)*(1.0*cos(th1(t)) - 2.6536e-6*sin(th1(t))) + 1.3268e-6*sin(th2(t) - 1.5708)*sin(th1(t))) - 1.0*sin(th3(t) - 1.5708)*(sin(th2(t) - 1.5708)*(1.0*cos(th1(t)) - 2.6536e-6*sin(th1(t))) - 1.3268e-6*cos(th2(t) - 1.5708)*sin(th1(t)))))) + 0.00018665;

M51 = 0.13038*(0.02*sin(th5(t))*(sin(th4(t) - 3.1416)*(cos(th3(t) - 1.5708)*(sin(th2(t) - 1.5708)*(1.0*cos(th1(t)) - 2.6536e-6*sin(th1(t))) - 1.3268e-6*cos(th2(t) - 1.5708)*sin(th1(t))) + sin(th3(t) - 1.5708)*(cos(th2(t) - 1.5708)*(1.0*cos(th1(t)) - 2.6536e-6*sin(th1(t))) + 1.3268e-6*sin(th2(t) - 1.5708)*sin(th1(t)))) + cos(th4(t) - 3.1416)*(cos(th3(t) - 1.5708)*(cos(th2(t) - 1.5708)*(1.0*cos(th1(t)) - 2.6536e-6*sin(th1(t))) + 1.3268e-6*sin(th2(t) - 1.5708)*sin(th1(t))) - 1.0*sin(th3(t) - 1.5708)*(sin(th2(t) - 1.5708)*(1.0*cos(th1(t)) - 2.6536e-6*sin(th1(t))) - 1.3268e-6*cos(th2(t) - 1.5708)*sin(th1(t))))) + 0.02*cos(th5(t))*(cos(th4(t) - 3.1416)*(cos(th3(t) - 1.5708)*(sin(th2(t) - 1.5708)*(1.0*cos(th1(t)) - 2.6536e-6*sin(th1(t))) - 1.3268e-6*cos(th2(t) - 1.5708)*sin(th1(t))) + sin(th3(t) - 1.5708)*(cos(th2(t) - 1.5708)*(1.0*cos(th1(t)) - 2.6536e-6*sin(th1(t))) + 1.3268e-6*sin(th2(t) - 1.5708)*sin(th1(t)))) - 1.0*sin(th4(t) - 3.1416)*(cos(th3(t) - 1.5708)*(cos(th2(t) - 1.5708)*(1.0*cos(th1(t)) - 2.6536e-6*sin(th1(t))) + 1.3268e-6*sin(th2(t) - 1.5708)*sin(th1(t))) - 1.0*sin(th3(t) - 1.5708)*(sin(th2(t) - 1.5708)*(1.0*cos(th1(t)) - 2.6536e-6*sin(th1(t))) - 1.3268e-6*cos(th2(t) - 1.5708)*sin(th1(t))))))*(5.0418e-7*cos(th1(t))*sin(th2(t)) + 0.02*cos(th5(t))*(cos(th4(t) - 3.1416)*(cos(th3(t) - 1.5708)*(cos(th2(t) - 1.5708)*(2.6536e-6*cos(th1(t)) + 1.0*sin(th1(t))) - 1.3268e-6*sin(th2(t) - 1.5708)*cos(th1(t))) - 1.0*sin(th3(t) - 1.5708)*(sin(th2(t) - 1.5708)*(2.6536e-6*cos(th1(t)) + 1.0*sin(th1(t))) + 1.3268e-6*cos(th2(t) - 1.5708)*cos(th1(t)))) + sin(th4(t) - 3.1416)*(cos(th3(t) - 1.5708)*(sin(th2(t) - 1.5708)*(2.6536e-6*cos(th1(t)) + 1.0*sin(th1(t))) + 1.3268e-6*cos(th2(t) - 1.5708)*cos(th1(t))) + sin(th3(t) - 1.5708)*(cos(th2(t) - 1.5708)*(2.6536e-6*cos(th1(t)) + 1.0*sin(th1(t))) - 1.3268e-6*sin(th2(t) - 1.5708)*cos(th1(t))))) + 0.38*sin(th4(t))*(cos(th3(t) - 1.5708)*(sin(th2(t) - 1.5708)*(2.6536e-6*cos(th1(t)) + 1.0*sin(th1(t))) + 1.3268e-6*cos(th2(t) - 1.5708)*cos(th1(t))) + sin(th3(t) - 1.5708)*(cos(th2(t) - 1.5708)*(2.6536e-6*cos(th1(t)) + 1.0*sin(th1(t))) - 1.3268e-6*sin(th2(t) - 1.5708)*cos(th1(t)))) - 0.38*cos(th3(t))*(cos(th2(t) - 1.5708)*(2.6536e-6*cos(th1(t)) + 1.0*sin(th1(t))) - 1.3268e-6*sin(th2(t) - 1.5708)*cos(th1(t))) - 0.38*cos(th2(t))*(2.6536e-6*cos(th1(t)) + 1.0*sin(th1(t))) + 0.38*sin(th3(t))*(sin(th2(t) - 1.5708)*(2.6536e-6*cos(th1(t)) + 1.0*sin(th1(t))) + 1.3268e-6*cos(th2(t) - 1.5708)*cos(th1(t))) - 0.38*cos(th4(t))*(cos(th3(t) - 1.5708)*(cos(th2(t) - 1.5708)*(2.6536e-6*cos(th1(t)) + 1.0*sin(th1(t))) - 1.3268e-6*sin(th2(t) - 1.5708)*cos(th1(t))) - 1.0*sin(th3(t) - 1.5708)*(sin(th2(t) - 1.5708)*(2.6536e-6*cos(th1(t)) + 1.0*sin(th1(t))) + 1.3268e-6*cos(th2(t) - 1.5708)*cos(th1(t)))) + 0.02*sin(th5(t))*(1.0*sin(th4(t) - 3.1416)*(cos(th3(t) - 1.5708)*(cos(th2(t) - 1.5708)*(2.6536e-6*cos(th1(t)) + 1.0*sin(th1(t))) - 1.3268e-6*sin(th2(t) - 1.5708)*cos(th1(t))) - 1.0*sin(th3(t) - 1.5708)*(sin(th2(t) - 1.5708)*(2.6536e-6*cos(th1(t)) + 1.0*sin(th1(t))) + 1.3268e-6*cos(th2(t) - 1.5708)*cos(th1(t)))) - cos(th4(t) - 3.1416)*(cos(th3(t) - 1.5708)*(sin(th2(t) - 1.5708)*(2.6536e-6*cos(th1(t)) + 1.0*sin(th1(t))) + 1.3268e-6*cos(th2(t) - 1.5708)*cos(th1(t))) + sin(th3(t) - 1.5708)*(cos(th2(t) - 1.5708)*(2.6536e-6*cos(th1(t)) + 1.0*sin(th1(t))) - 1.3268e-6*sin(th2(t) - 1.5708)*cos(th1(t)))))) + 0.13038*(0.02*cos(th5(t))*(sin(th4(t) - 3.1416)*(sin(th3(t) - 1.5708)*(sin(th2(t) - 1.5708)*(2.6536e-6*cos(th1(t)) + 1.0*sin(th1(t))) + 1.3268e-6*cos(th2(t) - 1.5708)*cos(th1(t))) - cos(th3(t) - 1.5708)*(1.0*cos(th2(t) - 1.5708)*(2.6536e-6*cos(th1(t)) + 1.0*sin(th1(t))) - 1.3268e-6*sin(th2(t) - 1.5708)*cos(th1(t)))) + cos(th4(t) - 3.1416)*(cos(th3(t) - 1.5708)*(sin(th2(t) - 1.5708)*(2.6536e-6*cos(th1(t)) + 1.0*sin(th1(t))) + 1.3268e-6*cos(th2(t) - 1.5708)*cos(th1(t))) + 1.0*sin(th3(t) - 1.5708)*(1.0*cos(th2(t) - 1.5708)*(2.6536e-6*cos(th1(t)) + 1.0*sin(th1(t))) - 1.3268e-6*sin(th2(t) - 1.5708)*cos(th1(t))))) - 0.02*sin(th5(t))*(cos(th4(t) - 3.1416)*(sin(th3(t) - 1.5708)*(sin(th2(t) - 1.5708)*(2.6536e-6*cos(th1(t)) + 1.0*sin(th1(t))) + 1.3268e-6*cos(th2(t) - 1.5708)*cos(th1(t))) - cos(th3(t) - 1.5708)*(1.0*cos(th2(t) - 1.5708)*(2.6536e-6*cos(th1(t)) + 1.0*sin(th1(t))) - 1.3268e-6*sin(th2(t) - 1.5708)*cos(th1(t)))) - 1.0*sin(th4(t) - 3.1416)*(cos(th3(t) - 1.5708)*(sin(th2(t) - 1.5708)*(2.6536e-6*cos(th1(t)) + 1.0*sin(th1(t))) + 1.3268e-6*cos(th2(t) - 1.5708)*cos(th1(t))) + 1.0*sin(th3(t) - 1.5708)*(1.0*cos(th2(t) - 1.5708)*(2.6536e-6*cos(th1(t)) + 1.0*sin(th1(t))) - 1.3268e-6*sin(th2(t) - 1.5708)*cos(th1(t))))))*(5.0418e-7*sin(th1(t))*sin(th2(t)) - 0.02*cos(th5(t))*(cos(th4(t) - 3.1416)*(cos(th3(t) - 1.5708)*(cos(th2(t) - 1.5708)*(1.0*cos(th1(t)) - 2.6536e-6*sin(th1(t))) + 1.3268e-6*sin(th2(t) - 1.5708)*sin(th1(t))) - sin(th3(t) - 1.5708)*(1.0*sin(th2(t) - 1.5708)*(1.0*cos(th1(t)) - 2.6536e-6*sin(th1(t))) - 1.3268e-6*cos(th2(t) - 1.5708)*sin(th1(t)))) + 1.0*sin(th4(t) - 3.1416)*(1.0*sin(th3(t) - 1.5708)*(cos(th2(t) - 1.5708)*(1.0*cos(th1(t)) - 2.6536e-6*sin(th1(t))) + 1.3268e-6*sin(th2(t) - 1.5708)*sin(th1(t))) + cos(th3(t) - 1.5708)*(1.0*sin(th2(t) - 1.5708)*(1.0*cos(th1(t)) - 2.6536e-6*sin(th1(t))) - 1.3268e-6*cos(th2(t) - 1.5708)*sin(th1(t))))) + 0.38*cos(th2(t))*(1.0*cos(th1(t)) - 2.6536e-6*sin(th1(t))) + 0.38*cos(th3(t))*(cos(th2(t) - 1.5708)*(1.0*cos(th1(t)) - 2.6536e-6*sin(th1(t))) + 1.3268e-6*sin(th2(t) - 1.5708)*sin(th1(t))) + 0.38*cos(th4(t))*(cos(th3(t) - 1.5708)*(cos(th2(t) - 1.5708)*(1.0*cos(th1(t)) - 2.6536e-6*sin(th1(t))) + 1.3268e-6*sin(th2(t) - 1.5708)*sin(th1(t))) - sin(th3(t) - 1.5708)*(1.0*sin(th2(t) - 1.5708)*(1.0*cos(th1(t)) - 2.6536e-6*sin(th1(t))) - 1.3268e-6*cos(th2(t) - 1.5708)*sin(th1(t)))) - 0.38*sin(th3(t))*(1.0*sin(th2(t) - 1.5708)*(1.0*cos(th1(t)) - 2.6536e-6*sin(th1(t))) - 1.3268e-6*cos(th2(t) - 1.5708)*sin(th1(t))) - 0.38*sin(th4(t))*(1.0*sin(th3(t) - 1.5708)*(cos(th2(t) - 1.5708)*(1.0*cos(th1(t)) - 2.6536e-6*sin(th1(t))) + 1.3268e-6*sin(th2(t) - 1.5708)*sin(th1(t))) + cos(th3(t) - 1.5708)*(1.0*sin(th2(t) - 1.5708)*(1.0*cos(th1(t)) - 2.6536e-6*sin(th1(t))) - 1.3268e-6*cos(th2(t) - 1.5708)*sin(th1(t)))) - 0.02*sin(th5(t))*(sin(th4(t) - 3.1416)*(cos(th3(t) - 1.5708)*(cos(th2(t) - 1.5708)*(1.0*cos(th1(t)) - 2.6536e-6*sin(th1(t))) + 1.3268e-6*sin(th2(t) - 1.5708)*sin(th1(t))) - sin(th3(t) - 1.5708)*(1.0*sin(th2(t) - 1.5708)*(1.0*cos(th1(t)) - 2.6536e-6*sin(th1(t))) - 1.3268e-6*cos(th2(t) - 1.5708)*sin(th1(t)))) - cos(th4(t) - 3.1416)*(1.0*sin(th3(t) - 1.5708)*(cos(th2(t) - 1.5708)*(1.0*cos(th1(t)) - 2.6536e-6*sin(th1(t))) + 1.3268e-6*sin(th2(t) - 1.5708)*sin(th1(t))) + cos(th3(t) - 1.5708)*(1.0*sin(th2(t) - 1.5708)*(1.0*cos(th1(t)) - 2.6536e-6*sin(th1(t))) - 1.3268e-6*cos(th2(t) - 1.5708)*sin(th1(t)))))) + 0.00018665;
M52 = 0.13038*(0.02*sin(th5(t))*(cos(th4(t) - 3.1416)*(cos(th3(t) - 1.5708)*(3.5208e-12*cos(th2(t) - 1.5708) + 1.0*sin(th2(t) - 1.5708)) + sin(th3(t) - 1.5708)*(1.0*cos(th2(t) - 1.5708) - 3.5208e-12*sin(th2(t) - 1.5708))) - 1.0*sin(th4(t) - 3.1416)*(cos(th3(t) - 1.5708)*(1.0*cos(th2(t) - 1.5708) - 3.5208e-12*sin(th2(t) - 1.5708)) - 1.0*sin(th3(t) - 1.5708)*(3.5208e-12*cos(th2(t) - 1.5708) + 1.0*sin(th2(t) - 1.5708)))) - 0.02*cos(th5(t))*(sin(th4(t) - 3.1416)*(cos(th3(t) - 1.5708)*(3.5208e-12*cos(th2(t) - 1.5708) + 1.0*sin(th2(t) - 1.5708)) + sin(th3(t) - 1.5708)*(1.0*cos(th2(t) - 1.5708) - 3.5208e-12*sin(th2(t) - 1.5708))) + cos(th4(t) - 3.1416)*(cos(th3(t) - 1.5708)*(1.0*cos(th2(t) - 1.5708) - 3.5208e-12*sin(th2(t) - 1.5708)) - 1.0*sin(th3(t) - 1.5708)*(3.5208e-12*cos(th2(t) - 1.5708) + 1.0*sin(th2(t) - 1.5708)))))*(0.38*cos(th2(t)) - 1.3379e-12*sin(th2(t)) - 0.38*sin(th3(t))*(3.5208e-12*cos(th2(t) - 1.5708) + 1.0*sin(th2(t) - 1.5708)) + 0.02*sin(th5(t))*(cos(th4(t) - 3.1416)*(cos(th3(t) - 1.5708)*(3.5208e-12*cos(th2(t) - 1.5708) + 1.0*sin(th2(t) - 1.5708)) + sin(th3(t) - 1.5708)*(1.0*cos(th2(t) - 1.5708) - 3.5208e-12*sin(th2(t) - 1.5708))) - 1.0*sin(th4(t) - 3.1416)*(cos(th3(t) - 1.5708)*(1.0*cos(th2(t) - 1.5708) - 3.5208e-12*sin(th2(t) - 1.5708)) - 1.0*sin(th3(t) - 1.5708)*(3.5208e-12*cos(th2(t) - 1.5708) + 1.0*sin(th2(t) - 1.5708)))) - 0.38*sin(th4(t))*(cos(th3(t) - 1.5708)*(3.5208e-12*cos(th2(t) - 1.5708) + 1.0*sin(th2(t) - 1.5708)) + sin(th3(t) - 1.5708)*(1.0*cos(th2(t) - 1.5708) - 3.5208e-12*sin(th2(t) - 1.5708))) + 0.38*cos(th4(t))*(cos(th3(t) - 1.5708)*(1.0*cos(th2(t) - 1.5708) - 3.5208e-12*sin(th2(t) - 1.5708)) - 1.0*sin(th3(t) - 1.5708)*(3.5208e-12*cos(th2(t) - 1.5708) + 1.0*sin(th2(t) - 1.5708))) + 0.38*cos(th3(t))*(1.0*cos(th2(t) - 1.5708) - 3.5208e-12*sin(th2(t) - 1.5708)) - 0.02*cos(th5(t))*(sin(th4(t) - 3.1416)*(cos(th3(t) - 1.5708)*(3.5208e-12*cos(th2(t) - 1.5708) + 1.0*sin(th2(t) - 1.5708)) + sin(th3(t) - 1.5708)*(1.0*cos(th2(t) - 1.5708) - 3.5208e-12*sin(th2(t) - 1.5708))) + cos(th4(t) - 3.1416)*(cos(th3(t) - 1.5708)*(1.0*cos(th2(t) - 1.5708) - 3.5208e-12*sin(th2(t) - 1.5708)) - 1.0*sin(th3(t) - 1.5708)*(3.5208e-12*cos(th2(t) - 1.5708) + 1.0*sin(th2(t) - 1.5708))))) - 0.13038*(0.02*sin(th5(t))*(sin(th4(t) - 3.1416)*(cos(th3(t) - 1.5708)*(sin(th2(t) - 1.5708)*(1.0*cos(th1(t)) - 2.6536e-6*sin(th1(t))) - 1.3268e-6*cos(th2(t) - 1.5708)*sin(th1(t))) + sin(th3(t) - 1.5708)*(cos(th2(t) - 1.5708)*(1.0*cos(th1(t)) - 2.6536e-6*sin(th1(t))) + 1.3268e-6*sin(th2(t) - 1.5708)*sin(th1(t)))) + cos(th4(t) - 3.1416)*(cos(th3(t) - 1.5708)*(cos(th2(t) - 1.5708)*(1.0*cos(th1(t)) - 2.6536e-6*sin(th1(t))) + 1.3268e-6*sin(th2(t) - 1.5708)*sin(th1(t))) - 1.0*sin(th3(t) - 1.5708)*(sin(th2(t) - 1.5708)*(1.0*cos(th1(t)) - 2.6536e-6*sin(th1(t))) - 1.3268e-6*cos(th2(t) - 1.5708)*sin(th1(t))))) + 0.02*cos(th5(t))*(cos(th4(t) - 3.1416)*(cos(th3(t) - 1.5708)*(sin(th2(t) - 1.5708)*(1.0*cos(th1(t)) - 2.6536e-6*sin(th1(t))) - 1.3268e-6*cos(th2(t) - 1.5708)*sin(th1(t))) + sin(th3(t) - 1.5708)*(cos(th2(t) - 1.5708)*(1.0*cos(th1(t)) - 2.6536e-6*sin(th1(t))) + 1.3268e-6*sin(th2(t) - 1.5708)*sin(th1(t)))) - 1.0*sin(th4(t) - 3.1416)*(cos(th3(t) - 1.5708)*(cos(th2(t) - 1.5708)*(1.0*cos(th1(t)) - 2.6536e-6*sin(th1(t))) + 1.3268e-6*sin(th2(t) - 1.5708)*sin(th1(t))) - 1.0*sin(th3(t) - 1.5708)*(sin(th2(t) - 1.5708)*(1.0*cos(th1(t)) - 2.6536e-6*sin(th1(t))) - 1.3268e-6*cos(th2(t) - 1.5708)*sin(th1(t))))))*(0.38*cos(th4(t))*(cos(th3(t) - 1.5708)*(sin(th2(t) - 1.5708)*(1.0*cos(th1(t)) - 2.6536e-6*sin(th1(t))) - 1.3268e-6*cos(th2(t) - 1.5708)*sin(th1(t))) + sin(th3(t) - 1.5708)*(cos(th2(t) - 1.5708)*(1.0*cos(th1(t)) - 2.6536e-6*sin(th1(t))) + 1.3268e-6*sin(th2(t) - 1.5708)*sin(th1(t)))) - 5.0418e-7*cos(th2(t))*sin(th1(t)) + 0.38*cos(th3(t))*(sin(th2(t) - 1.5708)*(1.0*cos(th1(t)) - 2.6536e-6*sin(th1(t))) - 1.3268e-6*cos(th2(t) - 1.5708)*sin(th1(t))) + 0.38*sin(th2(t))*(1.0*cos(th1(t)) - 2.6536e-6*sin(th1(t))) + 0.38*sin(th3(t))*(cos(th2(t) - 1.5708)*(1.0*cos(th1(t)) - 2.6536e-6*sin(th1(t))) + 1.3268e-6*sin(th2(t) - 1.5708)*sin(th1(t))) - 0.02*sin(th5(t))*(sin(th4(t) - 3.1416)*(cos(th3(t) - 1.5708)*(sin(th2(t) - 1.5708)*(1.0*cos(th1(t)) - 2.6536e-6*sin(th1(t))) - 1.3268e-6*cos(th2(t) - 1.5708)*sin(th1(t))) + sin(th3(t) - 1.5708)*(cos(th2(t) - 1.5708)*(1.0*cos(th1(t)) - 2.6536e-6*sin(th1(t))) + 1.3268e-6*sin(th2(t) - 1.5708)*sin(th1(t)))) + cos(th4(t) - 3.1416)*(cos(th3(t) - 1.5708)*(cos(th2(t) - 1.5708)*(1.0*cos(th1(t)) - 2.6536e-6*sin(th1(t))) + 1.3268e-6*sin(th2(t) - 1.5708)*sin(th1(t))) - 1.0*sin(th3(t) - 1.5708)*(sin(th2(t) - 1.5708)*(1.0*cos(th1(t)) - 2.6536e-6*sin(th1(t))) - 1.3268e-6*cos(th2(t) - 1.5708)*sin(th1(t))))) + 0.38*sin(th4(t))*(cos(th3(t) - 1.5708)*(cos(th2(t) - 1.5708)*(1.0*cos(th1(t)) - 2.6536e-6*sin(th1(t))) + 1.3268e-6*sin(th2(t) - 1.5708)*sin(th1(t))) - 1.0*sin(th3(t) - 1.5708)*(sin(th2(t) - 1.5708)*(1.0*cos(th1(t)) - 2.6536e-6*sin(th1(t))) - 1.3268e-6*cos(th2(t) - 1.5708)*sin(th1(t)))) - 0.02*cos(th5(t))*(cos(th4(t) - 3.1416)*(cos(th3(t) - 1.5708)*(sin(th2(t) - 1.5708)*(1.0*cos(th1(t)) - 2.6536e-6*sin(th1(t))) - 1.3268e-6*cos(th2(t) - 1.5708)*sin(th1(t))) + sin(th3(t) - 1.5708)*(cos(th2(t) - 1.5708)*(1.0*cos(th1(t)) - 2.6536e-6*sin(th1(t))) + 1.3268e-6*sin(th2(t) - 1.5708)*sin(th1(t)))) - 1.0*sin(th4(t) - 3.1416)*(cos(th3(t) - 1.5708)*(cos(th2(t) - 1.5708)*(1.0*cos(th1(t)) - 2.6536e-6*sin(th1(t))) + 1.3268e-6*sin(th2(t) - 1.5708)*sin(th1(t))) - 1.0*sin(th3(t) - 1.5708)*(sin(th2(t) - 1.5708)*(1.0*cos(th1(t)) - 2.6536e-6*sin(th1(t))) - 1.3268e-6*cos(th2(t) - 1.5708)*sin(th1(t)))))) - 0.13038*(0.02*cos(th5(t))*(sin(th4(t) - 3.1416)*(sin(th3(t) - 1.5708)*(sin(th2(t) - 1.5708)*(2.6536e-6*cos(th1(t)) + 1.0*sin(th1(t))) + 1.3268e-6*cos(th2(t) - 1.5708)*cos(th1(t))) - cos(th3(t) - 1.5708)*(1.0*cos(th2(t) - 1.5708)*(2.6536e-6*cos(th1(t)) + 1.0*sin(th1(t))) - 1.3268e-6*sin(th2(t) - 1.5708)*cos(th1(t)))) + cos(th4(t) - 3.1416)*(cos(th3(t) - 1.5708)*(sin(th2(t) - 1.5708)*(2.6536e-6*cos(th1(t)) + 1.0*sin(th1(t))) + 1.3268e-6*cos(th2(t) - 1.5708)*cos(th1(t))) + 1.0*sin(th3(t) - 1.5708)*(1.0*cos(th2(t) - 1.5708)*(2.6536e-6*cos(th1(t)) + 1.0*sin(th1(t))) - 1.3268e-6*sin(th2(t) - 1.5708)*cos(th1(t))))) - 0.02*sin(th5(t))*(cos(th4(t) - 3.1416)*(sin(th3(t) - 1.5708)*(sin(th2(t) - 1.5708)*(2.6536e-6*cos(th1(t)) + 1.0*sin(th1(t))) + 1.3268e-6*cos(th2(t) - 1.5708)*cos(th1(t))) - cos(th3(t) - 1.5708)*(1.0*cos(th2(t) - 1.5708)*(2.6536e-6*cos(th1(t)) + 1.0*sin(th1(t))) - 1.3268e-6*sin(th2(t) - 1.5708)*cos(th1(t)))) - 1.0*sin(th4(t) - 3.1416)*(cos(th3(t) - 1.5708)*(sin(th2(t) - 1.5708)*(2.6536e-6*cos(th1(t)) + 1.0*sin(th1(t))) + 1.3268e-6*cos(th2(t) - 1.5708)*cos(th1(t))) + 1.0*sin(th3(t) - 1.5708)*(1.0*cos(th2(t) - 1.5708)*(2.6536e-6*cos(th1(t)) + 1.0*sin(th1(t))) - 1.3268e-6*sin(th2(t) - 1.5708)*cos(th1(t))))))*(0.38*cos(th3(t))*(sin(th2(t) - 1.5708)*(2.6536e-6*cos(th1(t)) + 1.0*sin(th1(t))) + 1.3268e-6*cos(th2(t) - 1.5708)*cos(th1(t))) + 0.38*sin(th2(t))*(2.6536e-6*cos(th1(t)) + 1.0*sin(th1(t))) - 0.38*sin(th4(t))*(sin(th3(t) - 1.5708)*(sin(th2(t) - 1.5708)*(2.6536e-6*cos(th1(t)) + 1.0*sin(th1(t))) + 1.3268e-6*cos(th2(t) - 1.5708)*cos(th1(t))) - cos(th3(t) - 1.5708)*(1.0*cos(th2(t) - 1.5708)*(2.6536e-6*cos(th1(t)) + 1.0*sin(th1(t))) - 1.3268e-6*sin(th2(t) - 1.5708)*cos(th1(t)))) + 0.38*sin(th3(t))*(1.0*cos(th2(t) - 1.5708)*(2.6536e-6*cos(th1(t)) + 1.0*sin(th1(t))) - 1.3268e-6*sin(th2(t) - 1.5708)*cos(th1(t))) - 0.02*cos(th5(t))*(sin(th4(t) - 3.1416)*(sin(th3(t) - 1.5708)*(sin(th2(t) - 1.5708)*(2.6536e-6*cos(th1(t)) + 1.0*sin(th1(t))) + 1.3268e-6*cos(th2(t) - 1.5708)*cos(th1(t))) - cos(th3(t) - 1.5708)*(1.0*cos(th2(t) - 1.5708)*(2.6536e-6*cos(th1(t)) + 1.0*sin(th1(t))) - 1.3268e-6*sin(th2(t) - 1.5708)*cos(th1(t)))) + cos(th4(t) - 3.1416)*(cos(th3(t) - 1.5708)*(sin(th2(t) - 1.5708)*(2.6536e-6*cos(th1(t)) + 1.0*sin(th1(t))) + 1.3268e-6*cos(th2(t) - 1.5708)*cos(th1(t))) + 1.0*sin(th3(t) - 1.5708)*(1.0*cos(th2(t) - 1.5708)*(2.6536e-6*cos(th1(t)) + 1.0*sin(th1(t))) - 1.3268e-6*sin(th2(t) - 1.5708)*cos(th1(t))))) + 0.38*cos(th4(t))*(cos(th3(t) - 1.5708)*(sin(th2(t) - 1.5708)*(2.6536e-6*cos(th1(t)) + 1.0*sin(th1(t))) + 1.3268e-6*cos(th2(t) - 1.5708)*cos(th1(t))) + 1.0*sin(th3(t) - 1.5708)*(1.0*cos(th2(t) - 1.5708)*(2.6536e-6*cos(th1(t)) + 1.0*sin(th1(t))) - 1.3268e-6*sin(th2(t) - 1.5708)*cos(th1(t)))) + 0.02*sin(th5(t))*(cos(th4(t) - 3.1416)*(sin(th3(t) - 1.5708)*(sin(th2(t) - 1.5708)*(2.6536e-6*cos(th1(t)) + 1.0*sin(th1(t))) + 1.3268e-6*cos(th2(t) - 1.5708)*cos(th1(t))) - cos(th3(t) - 1.5708)*(1.0*cos(th2(t) - 1.5708)*(2.6536e-6*cos(th1(t)) + 1.0*sin(th1(t))) - 1.3268e-6*sin(th2(t) - 1.5708)*cos(th1(t)))) - 1.0*sin(th4(t) - 3.1416)*(cos(th3(t) - 1.5708)*(sin(th2(t) - 1.5708)*(2.6536e-6*cos(th1(t)) + 1.0*sin(th1(t))) + 1.3268e-6*cos(th2(t) - 1.5708)*cos(th1(t))) + 1.0*sin(th3(t) - 1.5708)*(1.0*cos(th2(t) - 1.5708)*(2.6536e-6*cos(th1(t)) + 1.0*sin(th1(t))) - 1.3268e-6*sin(th2(t) - 1.5708)*cos(th1(t))))) + 5.0418e-7*cos(th1(t))*cos(th2(t))) + 0.00018665;
M53 = 0.00018665 - 0.13038*(0.02*cos(th5(t))*(sin(th4(t) - 3.1416)*(sin(th3(t) - 1.5708)*(sin(th2(t) - 1.5708)*(2.6536e-6*cos(th1(t)) + 1.0*sin(th1(t))) + 1.3268e-6*cos(th2(t) - 1.5708)*cos(th1(t))) - cos(th3(t) - 1.5708)*(1.0*cos(th2(t) - 1.5708)*(2.6536e-6*cos(th1(t)) + 1.0*sin(th1(t))) - 1.3268e-6*sin(th2(t) - 1.5708)*cos(th1(t)))) + cos(th4(t) - 3.1416)*(cos(th3(t) - 1.5708)*(sin(th2(t) - 1.5708)*(2.6536e-6*cos(th1(t)) + 1.0*sin(th1(t))) + 1.3268e-6*cos(th2(t) - 1.5708)*cos(th1(t))) + 1.0*sin(th3(t) - 1.5708)*(1.0*cos(th2(t) - 1.5708)*(2.6536e-6*cos(th1(t)) + 1.0*sin(th1(t))) - 1.3268e-6*sin(th2(t) - 1.5708)*cos(th1(t))))) - 0.02*sin(th5(t))*(cos(th4(t) - 3.1416)*(sin(th3(t) - 1.5708)*(sin(th2(t) - 1.5708)*(2.6536e-6*cos(th1(t)) + 1.0*sin(th1(t))) + 1.3268e-6*cos(th2(t) - 1.5708)*cos(th1(t))) - cos(th3(t) - 1.5708)*(1.0*cos(th2(t) - 1.5708)*(2.6536e-6*cos(th1(t)) + 1.0*sin(th1(t))) - 1.3268e-6*sin(th2(t) - 1.5708)*cos(th1(t)))) - 1.0*sin(th4(t) - 3.1416)*(cos(th3(t) - 1.5708)*(sin(th2(t) - 1.5708)*(2.6536e-6*cos(th1(t)) + 1.0*sin(th1(t))) + 1.3268e-6*cos(th2(t) - 1.5708)*cos(th1(t))) + 1.0*sin(th3(t) - 1.5708)*(1.0*cos(th2(t) - 1.5708)*(2.6536e-6*cos(th1(t)) + 1.0*sin(th1(t))) - 1.3268e-6*sin(th2(t) - 1.5708)*cos(th1(t))))))*(0.38*cos(th3(t))*(sin(th2(t) - 1.5708)*(2.6536e-6*cos(th1(t)) + 1.0*sin(th1(t))) + 1.3268e-6*cos(th2(t) - 1.5708)*cos(th1(t))) - 0.38*sin(th4(t))*(sin(th3(t) - 1.5708)*(sin(th2(t) - 1.5708)*(2.6536e-6*cos(th1(t)) + 1.0*sin(th1(t))) + 1.3268e-6*cos(th2(t) - 1.5708)*cos(th1(t))) - cos(th3(t) - 1.5708)*(1.0*cos(th2(t) - 1.5708)*(2.6536e-6*cos(th1(t)) + 1.0*sin(th1(t))) - 1.3268e-6*sin(th2(t) - 1.5708)*cos(th1(t)))) + 0.38*sin(th3(t))*(1.0*cos(th2(t) - 1.5708)*(2.6536e-6*cos(th1(t)) + 1.0*sin(th1(t))) - 1.3268e-6*sin(th2(t) - 1.5708)*cos(th1(t))) - 0.02*cos(th5(t))*(sin(th4(t) - 3.1416)*(sin(th3(t) - 1.5708)*(sin(th2(t) - 1.5708)*(2.6536e-6*cos(th1(t)) + 1.0*sin(th1(t))) + 1.3268e-6*cos(th2(t) - 1.5708)*cos(th1(t))) - cos(th3(t) - 1.5708)*(1.0*cos(th2(t) - 1.5708)*(2.6536e-6*cos(th1(t)) + 1.0*sin(th1(t))) - 1.3268e-6*sin(th2(t) - 1.5708)*cos(th1(t)))) + cos(th4(t) - 3.1416)*(cos(th3(t) - 1.5708)*(sin(th2(t) - 1.5708)*(2.6536e-6*cos(th1(t)) + 1.0*sin(th1(t))) + 1.3268e-6*cos(th2(t) - 1.5708)*cos(th1(t))) + 1.0*sin(th3(t) - 1.5708)*(1.0*cos(th2(t) - 1.5708)*(2.6536e-6*cos(th1(t)) + 1.0*sin(th1(t))) - 1.3268e-6*sin(th2(t) - 1.5708)*cos(th1(t))))) + 0.38*cos(th4(t))*(cos(th3(t) - 1.5708)*(sin(th2(t) - 1.5708)*(2.6536e-6*cos(th1(t)) + 1.0*sin(th1(t))) + 1.3268e-6*cos(th2(t) - 1.5708)*cos(th1(t))) + 1.0*sin(th3(t) - 1.5708)*(1.0*cos(th2(t) - 1.5708)*(2.6536e-6*cos(th1(t)) + 1.0*sin(th1(t))) - 1.3268e-6*sin(th2(t) - 1.5708)*cos(th1(t)))) + 0.02*sin(th5(t))*(cos(th4(t) - 3.1416)*(sin(th3(t) - 1.5708)*(sin(th2(t) - 1.5708)*(2.6536e-6*cos(th1(t)) + 1.0*sin(th1(t))) + 1.3268e-6*cos(th2(t) - 1.5708)*cos(th1(t))) - cos(th3(t) - 1.5708)*(1.0*cos(th2(t) - 1.5708)*(2.6536e-6*cos(th1(t)) + 1.0*sin(th1(t))) - 1.3268e-6*sin(th2(t) - 1.5708)*cos(th1(t)))) - 1.0*sin(th4(t) - 3.1416)*(cos(th3(t) - 1.5708)*(sin(th2(t) - 1.5708)*(2.6536e-6*cos(th1(t)) + 1.0*sin(th1(t))) + 1.3268e-6*cos(th2(t) - 1.5708)*cos(th1(t))) + 1.0*sin(th3(t) - 1.5708)*(1.0*cos(th2(t) - 1.5708)*(2.6536e-6*cos(th1(t)) + 1.0*sin(th1(t))) - 1.3268e-6*sin(th2(t) - 1.5708)*cos(th1(t)))))) - 0.13038*(0.02*sin(th5(t))*(cos(th4(t) - 3.1416)*(cos(th3(t) - 1.5708)*(3.5208e-12*cos(th2(t) - 1.5708) + 1.0*sin(th2(t) - 1.5708)) + sin(th3(t) - 1.5708)*(1.0*cos(th2(t) - 1.5708) - 3.5208e-12*sin(th2(t) - 1.5708))) - 1.0*sin(th4(t) - 3.1416)*(cos(th3(t) - 1.5708)*(1.0*cos(th2(t) - 1.5708) - 3.5208e-12*sin(th2(t) - 1.5708)) - 1.0*sin(th3(t) - 1.5708)*(3.5208e-12*cos(th2(t) - 1.5708) + 1.0*sin(th2(t) - 1.5708)))) - 0.02*cos(th5(t))*(sin(th4(t) - 3.1416)*(cos(th3(t) - 1.5708)*(3.5208e-12*cos(th2(t) - 1.5708) + 1.0*sin(th2(t) - 1.5708)) + sin(th3(t) - 1.5708)*(1.0*cos(th2(t) - 1.5708) - 3.5208e-12*sin(th2(t) - 1.5708))) + cos(th4(t) - 3.1416)*(cos(th3(t) - 1.5708)*(1.0*cos(th2(t) - 1.5708) - 3.5208e-12*sin(th2(t) - 1.5708)) - 1.0*sin(th3(t) - 1.5708)*(3.5208e-12*cos(th2(t) - 1.5708) + 1.0*sin(th2(t) - 1.5708)))))*(0.38*sin(th3(t))*(3.5208e-12*cos(th2(t) - 1.5708) + 1.0*sin(th2(t) - 1.5708)) - 0.02*sin(th5(t))*(cos(th4(t) - 3.1416)*(cos(th3(t) - 1.5708)*(3.5208e-12*cos(th2(t) - 1.5708) + 1.0*sin(th2(t) - 1.5708)) + sin(th3(t) - 1.5708)*(1.0*cos(th2(t) - 1.5708) - 3.5208e-12*sin(th2(t) - 1.5708))) - 1.0*sin(th4(t) - 3.1416)*(cos(th3(t) - 1.5708)*(1.0*cos(th2(t) - 1.5708) - 3.5208e-12*sin(th2(t) - 1.5708)) - 1.0*sin(th3(t) - 1.5708)*(3.5208e-12*cos(th2(t) - 1.5708) + 1.0*sin(th2(t) - 1.5708)))) + 0.38*sin(th4(t))*(cos(th3(t) - 1.5708)*(3.5208e-12*cos(th2(t) - 1.5708) + 1.0*sin(th2(t) - 1.5708)) + sin(th3(t) - 1.5708)*(1.0*cos(th2(t) - 1.5708) - 3.5208e-12*sin(th2(t) - 1.5708))) - 0.38*cos(th4(t))*(cos(th3(t) - 1.5708)*(1.0*cos(th2(t) - 1.5708) - 3.5208e-12*sin(th2(t) - 1.5708)) - 1.0*sin(th3(t) - 1.5708)*(3.5208e-12*cos(th2(t) - 1.5708) + 1.0*sin(th2(t) - 1.5708))) - 0.38*cos(th3(t))*(1.0*cos(th2(t) - 1.5708) - 3.5208e-12*sin(th2(t) - 1.5708)) + 0.02*cos(th5(t))*(sin(th4(t) - 3.1416)*(cos(th3(t) - 1.5708)*(3.5208e-12*cos(th2(t) - 1.5708) + 1.0*sin(th2(t) - 1.5708)) + sin(th3(t) - 1.5708)*(1.0*cos(th2(t) - 1.5708) - 3.5208e-12*sin(th2(t) - 1.5708))) + cos(th4(t) - 3.1416)*(cos(th3(t) - 1.5708)*(1.0*cos(th2(t) - 1.5708) - 3.5208e-12*sin(th2(t) - 1.5708)) - 1.0*sin(th3(t) - 1.5708)*(3.5208e-12*cos(th2(t) - 1.5708) + 1.0*sin(th2(t) - 1.5708))))) - 0.13038*(0.02*sin(th5(t))*(sin(th4(t) - 3.1416)*(cos(th3(t) - 1.5708)*(sin(th2(t) - 1.5708)*(1.0*cos(th1(t)) - 2.6536e-6*sin(th1(t))) - 1.3268e-6*cos(th2(t) - 1.5708)*sin(th1(t))) + sin(th3(t) - 1.5708)*(cos(th2(t) - 1.5708)*(1.0*cos(th1(t)) - 2.6536e-6*sin(th1(t))) + 1.3268e-6*sin(th2(t) - 1.5708)*sin(th1(t)))) + cos(th4(t) - 3.1416)*(cos(th3(t) - 1.5708)*(cos(th2(t) - 1.5708)*(1.0*cos(th1(t)) - 2.6536e-6*sin(th1(t))) + 1.3268e-6*sin(th2(t) - 1.5708)*sin(th1(t))) - 1.0*sin(th3(t) - 1.5708)*(sin(th2(t) - 1.5708)*(1.0*cos(th1(t)) - 2.6536e-6*sin(th1(t))) - 1.3268e-6*cos(th2(t) - 1.5708)*sin(th1(t))))) + 0.02*cos(th5(t))*(cos(th4(t) - 3.1416)*(cos(th3(t) - 1.5708)*(sin(th2(t) - 1.5708)*(1.0*cos(th1(t)) - 2.6536e-6*sin(th1(t))) - 1.3268e-6*cos(th2(t) - 1.5708)*sin(th1(t))) + sin(th3(t) - 1.5708)*(cos(th2(t) - 1.5708)*(1.0*cos(th1(t)) - 2.6536e-6*sin(th1(t))) + 1.3268e-6*sin(th2(t) - 1.5708)*sin(th1(t)))) - 1.0*sin(th4(t) - 3.1416)*(cos(th3(t) - 1.5708)*(cos(th2(t) - 1.5708)*(1.0*cos(th1(t)) - 2.6536e-6*sin(th1(t))) + 1.3268e-6*sin(th2(t) - 1.5708)*sin(th1(t))) - 1.0*sin(th3(t) - 1.5708)*(sin(th2(t) - 1.5708)*(1.0*cos(th1(t)) - 2.6536e-6*sin(th1(t))) - 1.3268e-6*cos(th2(t) - 1.5708)*sin(th1(t))))))*(0.38*cos(th4(t))*(cos(th3(t) - 1.5708)*(sin(th2(t) - 1.5708)*(1.0*cos(th1(t)) - 2.6536e-6*sin(th1(t))) - 1.3268e-6*cos(th2(t) - 1.5708)*sin(th1(t))) + sin(th3(t) - 1.5708)*(cos(th2(t) - 1.5708)*(1.0*cos(th1(t)) - 2.6536e-6*sin(th1(t))) + 1.3268e-6*sin(th2(t) - 1.5708)*sin(th1(t)))) + 0.38*cos(th3(t))*(sin(th2(t) - 1.5708)*(1.0*cos(th1(t)) - 2.6536e-6*sin(th1(t))) - 1.3268e-6*cos(th2(t) - 1.5708)*sin(th1(t))) + 0.38*sin(th3(t))*(cos(th2(t) - 1.5708)*(1.0*cos(th1(t)) - 2.6536e-6*sin(th1(t))) + 1.3268e-6*sin(th2(t) - 1.5708)*sin(th1(t))) - 0.02*sin(th5(t))*(sin(th4(t) - 3.1416)*(cos(th3(t) - 1.5708)*(sin(th2(t) - 1.5708)*(1.0*cos(th1(t)) - 2.6536e-6*sin(th1(t))) - 1.3268e-6*cos(th2(t) - 1.5708)*sin(th1(t))) + sin(th3(t) - 1.5708)*(cos(th2(t) - 1.5708)*(1.0*cos(th1(t)) - 2.6536e-6*sin(th1(t))) + 1.3268e-6*sin(th2(t) - 1.5708)*sin(th1(t)))) + cos(th4(t) - 3.1416)*(cos(th3(t) - 1.5708)*(cos(th2(t) - 1.5708)*(1.0*cos(th1(t)) - 2.6536e-6*sin(th1(t))) + 1.3268e-6*sin(th2(t) - 1.5708)*sin(th1(t))) - 1.0*sin(th3(t) - 1.5708)*(sin(th2(t) - 1.5708)*(1.0*cos(th1(t)) - 2.6536e-6*sin(th1(t))) - 1.3268e-6*cos(th2(t) - 1.5708)*sin(th1(t))))) + 0.38*sin(th4(t))*(cos(th3(t) - 1.5708)*(cos(th2(t) - 1.5708)*(1.0*cos(th1(t)) - 2.6536e-6*sin(th1(t))) + 1.3268e-6*sin(th2(t) - 1.5708)*sin(th1(t))) - 1.0*sin(th3(t) - 1.5708)*(sin(th2(t) - 1.5708)*(1.0*cos(th1(t)) - 2.6536e-6*sin(th1(t))) - 1.3268e-6*cos(th2(t) - 1.5708)*sin(th1(t)))) - 0.02*cos(th5(t))*(cos(th4(t) - 3.1416)*(cos(th3(t) - 1.5708)*(sin(th2(t) - 1.5708)*(1.0*cos(th1(t)) - 2.6536e-6*sin(th1(t))) - 1.3268e-6*cos(th2(t) - 1.5708)*sin(th1(t))) + sin(th3(t) - 1.5708)*(cos(th2(t) - 1.5708)*(1.0*cos(th1(t)) - 2.6536e-6*sin(th1(t))) + 1.3268e-6*sin(th2(t) - 1.5708)*sin(th1(t)))) - 1.0*sin(th4(t) - 3.1416)*(cos(th3(t) - 1.5708)*(cos(th2(t) - 1.5708)*(1.0*cos(th1(t)) - 2.6536e-6*sin(th1(t))) + 1.3268e-6*sin(th2(t) - 1.5708)*sin(th1(t))) - 1.0*sin(th3(t) - 1.5708)*(sin(th2(t) - 1.5708)*(1.0*cos(th1(t)) - 2.6536e-6*sin(th1(t))) - 1.3268e-6*cos(th2(t) - 1.5708)*sin(th1(t))))));
M54 = 0.13038*(0.02*cos(th5(t))*(sin(th4(t) - 3.1416)*(sin(th3(t) - 1.5708)*(sin(th2(t) - 1.5708)*(2.6536e-6*cos(th1(t)) + 1.0*sin(th1(t))) + 1.3268e-6*cos(th2(t) - 1.5708)*cos(th1(t))) - cos(th3(t) - 1.5708)*(1.0*cos(th2(t) - 1.5708)*(2.6536e-6*cos(th1(t)) + 1.0*sin(th1(t))) - 1.3268e-6*sin(th2(t) - 1.5708)*cos(th1(t)))) + cos(th4(t) - 3.1416)*(cos(th3(t) - 1.5708)*(sin(th2(t) - 1.5708)*(2.6536e-6*cos(th1(t)) + 1.0*sin(th1(t))) + 1.3268e-6*cos(th2(t) - 1.5708)*cos(th1(t))) + 1.0*sin(th3(t) - 1.5708)*(1.0*cos(th2(t) - 1.5708)*(2.6536e-6*cos(th1(t)) + 1.0*sin(th1(t))) - 1.3268e-6*sin(th2(t) - 1.5708)*cos(th1(t))))) - 0.02*sin(th5(t))*(cos(th4(t) - 3.1416)*(sin(th3(t) - 1.5708)*(sin(th2(t) - 1.5708)*(2.6536e-6*cos(th1(t)) + 1.0*sin(th1(t))) + 1.3268e-6*cos(th2(t) - 1.5708)*cos(th1(t))) - cos(th3(t) - 1.5708)*(1.0*cos(th2(t) - 1.5708)*(2.6536e-6*cos(th1(t)) + 1.0*sin(th1(t))) - 1.3268e-6*sin(th2(t) - 1.5708)*cos(th1(t)))) - 1.0*sin(th4(t) - 3.1416)*(cos(th3(t) - 1.5708)*(sin(th2(t) - 1.5708)*(2.6536e-6*cos(th1(t)) + 1.0*sin(th1(t))) + 1.3268e-6*cos(th2(t) - 1.5708)*cos(th1(t))) + 1.0*sin(th3(t) - 1.5708)*(1.0*cos(th2(t) - 1.5708)*(2.6536e-6*cos(th1(t)) + 1.0*sin(th1(t))) - 1.3268e-6*sin(th2(t) - 1.5708)*cos(th1(t))))))*(0.38*sin(th4(t))*(sin(th3(t) - 1.5708)*(sin(th2(t) - 1.5708)*(2.6536e-6*cos(th1(t)) + 1.0*sin(th1(t))) + 1.3268e-6*cos(th2(t) - 1.5708)*cos(th1(t))) - cos(th3(t) - 1.5708)*(1.0*cos(th2(t) - 1.5708)*(2.6536e-6*cos(th1(t)) + 1.0*sin(th1(t))) - 1.3268e-6*sin(th2(t) - 1.5708)*cos(th1(t)))) - 0.02*cos(th5(t))*(sin(th4(t) - 3.1416)*(sin(th3(t) - 1.5708)*(sin(th2(t) - 1.5708)*(2.6536e-6*cos(th1(t)) + 1.0*sin(th1(t))) + 1.3268e-6*cos(th2(t) - 1.5708)*cos(th1(t))) - cos(th3(t) - 1.5708)*(1.0*cos(th2(t) - 1.5708)*(2.6536e-6*cos(th1(t)) + 1.0*sin(th1(t))) - 1.3268e-6*sin(th2(t) - 1.5708)*cos(th1(t)))) + cos(th4(t) - 3.1416)*(cos(th3(t) - 1.5708)*(sin(th2(t) - 1.5708)*(2.6536e-6*cos(th1(t)) + 1.0*sin(th1(t))) + 1.3268e-6*cos(th2(t) - 1.5708)*cos(th1(t))) + 1.0*sin(th3(t) - 1.5708)*(1.0*cos(th2(t) - 1.5708)*(2.6536e-6*cos(th1(t)) + 1.0*sin(th1(t))) - 1.3268e-6*sin(th2(t) - 1.5708)*cos(th1(t))))) - 0.38*cos(th4(t))*(cos(th3(t) - 1.5708)*(sin(th2(t) - 1.5708)*(2.6536e-6*cos(th1(t)) + 1.0*sin(th1(t))) + 1.3268e-6*cos(th2(t) - 1.5708)*cos(th1(t))) + 1.0*sin(th3(t) - 1.5708)*(1.0*cos(th2(t) - 1.5708)*(2.6536e-6*cos(th1(t)) + 1.0*sin(th1(t))) - 1.3268e-6*sin(th2(t) - 1.5708)*cos(th1(t)))) + 0.02*sin(th5(t))*(cos(th4(t) - 3.1416)*(sin(th3(t) - 1.5708)*(sin(th2(t) - 1.5708)*(2.6536e-6*cos(th1(t)) + 1.0*sin(th1(t))) + 1.3268e-6*cos(th2(t) - 1.5708)*cos(th1(t))) - cos(th3(t) - 1.5708)*(1.0*cos(th2(t) - 1.5708)*(2.6536e-6*cos(th1(t)) + 1.0*sin(th1(t))) - 1.3268e-6*sin(th2(t) - 1.5708)*cos(th1(t)))) - 1.0*sin(th4(t) - 3.1416)*(cos(th3(t) - 1.5708)*(sin(th2(t) - 1.5708)*(2.6536e-6*cos(th1(t)) + 1.0*sin(th1(t))) + 1.3268e-6*cos(th2(t) - 1.5708)*cos(th1(t))) + 1.0*sin(th3(t) - 1.5708)*(1.0*cos(th2(t) - 1.5708)*(2.6536e-6*cos(th1(t)) + 1.0*sin(th1(t))) - 1.3268e-6*sin(th2(t) - 1.5708)*cos(th1(t)))))) - 0.13038*(0.02*sin(th5(t))*(cos(th4(t) - 3.1416)*(cos(th3(t) - 1.5708)*(3.5208e-12*cos(th2(t) - 1.5708) + 1.0*sin(th2(t) - 1.5708)) + sin(th3(t) - 1.5708)*(1.0*cos(th2(t) - 1.5708) - 3.5208e-12*sin(th2(t) - 1.5708))) - 1.0*sin(th4(t) - 3.1416)*(cos(th3(t) - 1.5708)*(1.0*cos(th2(t) - 1.5708) - 3.5208e-12*sin(th2(t) - 1.5708)) - 1.0*sin(th3(t) - 1.5708)*(3.5208e-12*cos(th2(t) - 1.5708) + 1.0*sin(th2(t) - 1.5708)))) - 0.02*cos(th5(t))*(sin(th4(t) - 3.1416)*(cos(th3(t) - 1.5708)*(3.5208e-12*cos(th2(t) - 1.5708) + 1.0*sin(th2(t) - 1.5708)) + sin(th3(t) - 1.5708)*(1.0*cos(th2(t) - 1.5708) - 3.5208e-12*sin(th2(t) - 1.5708))) + cos(th4(t) - 3.1416)*(cos(th3(t) - 1.5708)*(1.0*cos(th2(t) - 1.5708) - 3.5208e-12*sin(th2(t) - 1.5708)) - 1.0*sin(th3(t) - 1.5708)*(3.5208e-12*cos(th2(t) - 1.5708) + 1.0*sin(th2(t) - 1.5708)))))*(0.02*sin(th5(t))*(cos(th4(t) - 3.1416)*(cos(th3(t) - 1.5708)*(3.5208e-12*cos(th2(t) - 1.5708) + 1.0*sin(th2(t) - 1.5708)) + sin(th3(t) - 1.5708)*(1.0*cos(th2(t) - 1.5708) - 3.5208e-12*sin(th2(t) - 1.5708))) - 1.0*sin(th4(t) - 3.1416)*(cos(th3(t) - 1.5708)*(1.0*cos(th2(t) - 1.5708) - 3.5208e-12*sin(th2(t) - 1.5708)) - 1.0*sin(th3(t) - 1.5708)*(3.5208e-12*cos(th2(t) - 1.5708) + 1.0*sin(th2(t) - 1.5708)))) + 0.38*sin(th4(t))*(cos(th3(t) - 1.5708)*(3.5208e-12*cos(th2(t) - 1.5708) + 1.0*sin(th2(t) - 1.5708)) + sin(th3(t) - 1.5708)*(1.0*cos(th2(t) - 1.5708) - 3.5208e-12*sin(th2(t) - 1.5708))) - 0.38*cos(th4(t))*(cos(th3(t) - 1.5708)*(1.0*cos(th2(t) - 1.5708) - 3.5208e-12*sin(th2(t) - 1.5708)) - 1.0*sin(th3(t) - 1.5708)*(3.5208e-12*cos(th2(t) - 1.5708) + 1.0*sin(th2(t) - 1.5708))) - 0.02*cos(th5(t))*(sin(th4(t) - 3.1416)*(cos(th3(t) - 1.5708)*(3.5208e-12*cos(th2(t) - 1.5708) + 1.0*sin(th2(t) - 1.5708)) + sin(th3(t) - 1.5708)*(1.0*cos(th2(t) - 1.5708) - 3.5208e-12*sin(th2(t) - 1.5708))) + cos(th4(t) - 3.1416)*(cos(th3(t) - 1.5708)*(1.0*cos(th2(t) - 1.5708) - 3.5208e-12*sin(th2(t) - 1.5708)) - 1.0*sin(th3(t) - 1.5708)*(3.5208e-12*cos(th2(t) - 1.5708) + 1.0*sin(th2(t) - 1.5708))))) - 0.13038*(0.02*sin(th5(t))*(sin(th4(t) - 3.1416)*(cos(th3(t) - 1.5708)*(sin(th2(t) - 1.5708)*(1.0*cos(th1(t)) - 2.6536e-6*sin(th1(t))) - 1.3268e-6*cos(th2(t) - 1.5708)*sin(th1(t))) + sin(th3(t) - 1.5708)*(cos(th2(t) - 1.5708)*(1.0*cos(th1(t)) - 2.6536e-6*sin(th1(t))) + 1.3268e-6*sin(th2(t) - 1.5708)*sin(th1(t)))) + cos(th4(t) - 3.1416)*(cos(th3(t) - 1.5708)*(cos(th2(t) - 1.5708)*(1.0*cos(th1(t)) - 2.6536e-6*sin(th1(t))) + 1.3268e-6*sin(th2(t) - 1.5708)*sin(th1(t))) - 1.0*sin(th3(t) - 1.5708)*(sin(th2(t) - 1.5708)*(1.0*cos(th1(t)) - 2.6536e-6*sin(th1(t))) - 1.3268e-6*cos(th2(t) - 1.5708)*sin(th1(t))))) + 0.02*cos(th5(t))*(cos(th4(t) - 3.1416)*(cos(th3(t) - 1.5708)*(sin(th2(t) - 1.5708)*(1.0*cos(th1(t)) - 2.6536e-6*sin(th1(t))) - 1.3268e-6*cos(th2(t) - 1.5708)*sin(th1(t))) + sin(th3(t) - 1.5708)*(cos(th2(t) - 1.5708)*(1.0*cos(th1(t)) - 2.6536e-6*sin(th1(t))) + 1.3268e-6*sin(th2(t) - 1.5708)*sin(th1(t)))) - 1.0*sin(th4(t) - 3.1416)*(cos(th3(t) - 1.5708)*(cos(th2(t) - 1.5708)*(1.0*cos(th1(t)) - 2.6536e-6*sin(th1(t))) + 1.3268e-6*sin(th2(t) - 1.5708)*sin(th1(t))) - 1.0*sin(th3(t) - 1.5708)*(sin(th2(t) - 1.5708)*(1.0*cos(th1(t)) - 2.6536e-6*sin(th1(t))) - 1.3268e-6*cos(th2(t) - 1.5708)*sin(th1(t))))))*(0.38*cos(th4(t))*(cos(th3(t) - 1.5708)*(sin(th2(t) - 1.5708)*(1.0*cos(th1(t)) - 2.6536e-6*sin(th1(t))) - 1.3268e-6*cos(th2(t) - 1.5708)*sin(th1(t))) + sin(th3(t) - 1.5708)*(cos(th2(t) - 1.5708)*(1.0*cos(th1(t)) - 2.6536e-6*sin(th1(t))) + 1.3268e-6*sin(th2(t) - 1.5708)*sin(th1(t)))) + 0.02*sin(th5(t))*(sin(th4(t) - 3.1416)*(cos(th3(t) - 1.5708)*(sin(th2(t) - 1.5708)*(1.0*cos(th1(t)) - 2.6536e-6*sin(th1(t))) - 1.3268e-6*cos(th2(t) - 1.5708)*sin(th1(t))) + sin(th3(t) - 1.5708)*(cos(th2(t) - 1.5708)*(1.0*cos(th1(t)) - 2.6536e-6*sin(th1(t))) + 1.3268e-6*sin(th2(t) - 1.5708)*sin(th1(t)))) + cos(th4(t) - 3.1416)*(cos(th3(t) - 1.5708)*(cos(th2(t) - 1.5708)*(1.0*cos(th1(t)) - 2.6536e-6*sin(th1(t))) + 1.3268e-6*sin(th2(t) - 1.5708)*sin(th1(t))) - 1.0*sin(th3(t) - 1.5708)*(sin(th2(t) - 1.5708)*(1.0*cos(th1(t)) - 2.6536e-6*sin(th1(t))) - 1.3268e-6*cos(th2(t) - 1.5708)*sin(th1(t))))) + 0.38*sin(th4(t))*(cos(th3(t) - 1.5708)*(cos(th2(t) - 1.5708)*(1.0*cos(th1(t)) - 2.6536e-6*sin(th1(t))) + 1.3268e-6*sin(th2(t) - 1.5708)*sin(th1(t))) - 1.0*sin(th3(t) - 1.5708)*(sin(th2(t) - 1.5708)*(1.0*cos(th1(t)) - 2.6536e-6*sin(th1(t))) - 1.3268e-6*cos(th2(t) - 1.5708)*sin(th1(t)))) + 0.02*cos(th5(t))*(cos(th4(t) - 3.1416)*(cos(th3(t) - 1.5708)*(sin(th2(t) - 1.5708)*(1.0*cos(th1(t)) - 2.6536e-6*sin(th1(t))) - 1.3268e-6*cos(th2(t) - 1.5708)*sin(th1(t))) + sin(th3(t) - 1.5708)*(cos(th2(t) - 1.5708)*(1.0*cos(th1(t)) - 2.6536e-6*sin(th1(t))) + 1.3268e-6*sin(th2(t) - 1.5708)*sin(th1(t)))) - 1.0*sin(th4(t) - 3.1416)*(cos(th3(t) - 1.5708)*(cos(th2(t) - 1.5708)*(1.0*cos(th1(t)) - 2.6536e-6*sin(th1(t))) + 1.3268e-6*sin(th2(t) - 1.5708)*sin(th1(t))) - 1.0*sin(th3(t) - 1.5708)*(sin(th2(t) - 1.5708)*(1.0*cos(th1(t)) - 2.6536e-6*sin(th1(t))) - 1.3268e-6*cos(th2(t) - 1.5708)*sin(th1(t)))))) + 0.00018665;
M55 = 0.13038*(0.02*sin(th5(t))*(sin(th4(t) - 3.1416)*(cos(th3(t) - 1.5708)*(sin(th2(t) - 1.5708)*(1.0*cos(th1(t)) - 2.6536e-6*sin(th1(t))) - 1.3268e-6*cos(th2(t) - 1.5708)*sin(th1(t))) + sin(th3(t) - 1.5708)*(cos(th2(t) - 1.5708)*(1.0*cos(th1(t)) - 2.6536e-6*sin(th1(t))) + 1.3268e-6*sin(th2(t) - 1.5708)*sin(th1(t)))) + cos(th4(t) - 3.1416)*(cos(th3(t) - 1.5708)*(cos(th2(t) - 1.5708)*(1.0*cos(th1(t)) - 2.6536e-6*sin(th1(t))) + 1.3268e-6*sin(th2(t) - 1.5708)*sin(th1(t))) - 1.0*sin(th3(t) - 1.5708)*(sin(th2(t) - 1.5708)*(1.0*cos(th1(t)) - 2.6536e-6*sin(th1(t))) - 1.3268e-6*cos(th2(t) - 1.5708)*sin(th1(t))))) + 0.02*cos(th5(t))*(cos(th4(t) - 3.1416)*(cos(th3(t) - 1.5708)*(sin(th2(t) - 1.5708)*(1.0*cos(th1(t)) - 2.6536e-6*sin(th1(t))) - 1.3268e-6*cos(th2(t) - 1.5708)*sin(th1(t))) + sin(th3(t) - 1.5708)*(cos(th2(t) - 1.5708)*(1.0*cos(th1(t)) - 2.6536e-6*sin(th1(t))) + 1.3268e-6*sin(th2(t) - 1.5708)*sin(th1(t)))) - 1.0*sin(th4(t) - 3.1416)*(cos(th3(t) - 1.5708)*(cos(th2(t) - 1.5708)*(1.0*cos(th1(t)) - 2.6536e-6*sin(th1(t))) + 1.3268e-6*sin(th2(t) - 1.5708)*sin(th1(t))) - 1.0*sin(th3(t) - 1.5708)*(sin(th2(t) - 1.5708)*(1.0*cos(th1(t)) - 2.6536e-6*sin(th1(t))) - 1.3268e-6*cos(th2(t) - 1.5708)*sin(th1(t))))))^2 + 0.13038*(0.02*sin(th5(t))*(cos(th4(t) - 3.1416)*(cos(th3(t) - 1.5708)*(3.5208e-12*cos(th2(t) - 1.5708) + 1.0*sin(th2(t) - 1.5708)) + sin(th3(t) - 1.5708)*(1.0*cos(th2(t) - 1.5708) - 3.5208e-12*sin(th2(t) - 1.5708))) - 1.0*sin(th4(t) - 3.1416)*(cos(th3(t) - 1.5708)*(1.0*cos(th2(t) - 1.5708) - 3.5208e-12*sin(th2(t) - 1.5708)) - 1.0*sin(th3(t) - 1.5708)*(3.5208e-12*cos(th2(t) - 1.5708) + 1.0*sin(th2(t) - 1.5708)))) - 0.02*cos(th5(t))*(sin(th4(t) - 3.1416)*(cos(th3(t) - 1.5708)*(3.5208e-12*cos(th2(t) - 1.5708) + 1.0*sin(th2(t) - 1.5708)) + sin(th3(t) - 1.5708)*(1.0*cos(th2(t) - 1.5708) - 3.5208e-12*sin(th2(t) - 1.5708))) + cos(th4(t) - 3.1416)*(cos(th3(t) - 1.5708)*(1.0*cos(th2(t) - 1.5708) - 3.5208e-12*sin(th2(t) - 1.5708)) - 1.0*sin(th3(t) - 1.5708)*(3.5208e-12*cos(th2(t) - 1.5708) + 1.0*sin(th2(t) - 1.5708)))))^2 + 0.13038*(0.02*cos(th5(t))*(sin(th4(t) - 3.1416)*(sin(th3(t) - 1.5708)*(sin(th2(t) - 1.5708)*(2.6536e-6*cos(th1(t)) + 1.0*sin(th1(t))) + 1.3268e-6*cos(th2(t) - 1.5708)*cos(th1(t))) - cos(th3(t) - 1.5708)*(1.0*cos(th2(t) - 1.5708)*(2.6536e-6*cos(th1(t)) + 1.0*sin(th1(t))) - 1.3268e-6*sin(th2(t) - 1.5708)*cos(th1(t)))) + cos(th4(t) - 3.1416)*(cos(th3(t) - 1.5708)*(sin(th2(t) - 1.5708)*(2.6536e-6*cos(th1(t)) + 1.0*sin(th1(t))) + 1.3268e-6*cos(th2(t) - 1.5708)*cos(th1(t))) + 1.0*sin(th3(t) - 1.5708)*(1.0*cos(th2(t) - 1.5708)*(2.6536e-6*cos(th1(t)) + 1.0*sin(th1(t))) - 1.3268e-6*sin(th2(t) - 1.5708)*cos(th1(t))))) - 0.02*sin(th5(t))*(cos(th4(t) - 3.1416)*(sin(th3(t) - 1.5708)*(sin(th2(t) - 1.5708)*(2.6536e-6*cos(th1(t)) + 1.0*sin(th1(t))) + 1.3268e-6*cos(th2(t) - 1.5708)*cos(th1(t))) - cos(th3(t) - 1.5708)*(1.0*cos(th2(t) - 1.5708)*(2.6536e-6*cos(th1(t)) + 1.0*sin(th1(t))) - 1.3268e-6*sin(th2(t) - 1.5708)*cos(th1(t)))) - 1.0*sin(th4(t) - 3.1416)*(cos(th3(t) - 1.5708)*(sin(th2(t) - 1.5708)*(2.6536e-6*cos(th1(t)) + 1.0*sin(th1(t))) + 1.3268e-6*cos(th2(t) - 1.5708)*cos(th1(t))) + 1.0*sin(th3(t) - 1.5708)*(1.0*cos(th2(t) - 1.5708)*(2.6536e-6*cos(th1(t)) + 1.0*sin(th1(t))) - 1.3268e-6*sin(th2(t) - 1.5708)*cos(th1(t))))))^2 + 0.00018665;

M_matrix = [
    M11, M12, M13, M14, M15;
    M21, M22, M23, M24, M25;
    M31, M32, M33, M34, M35;
    M41, M42, M43, M44, M45;
    M51, M52, M53, M54, M55
    ];


M_inverse = inv(M_matrix);
